simulink model "simulator_prototype_v2"  (R2021b)
(part 10 of 12)

t7179 = ct{2001};
t7181 = ct{2002};
t7185 = ct{2003};
t7187 = ct{2004};
t7188 = ct{2005};
t7193 = ct{2006};
t7195 = ct{2007};
t7198 = ct{2008};
t7200 = ct{2009};
t7201 = ct{2010};
t7204 = ct{2011};
t7209 = ct{2012};
t721 = ct{2013};
t7210 = ct{2014};
t7211 = ct{2015};
t7215 = ct{2016};
t7219 = ct{2017};
t722 = ct{2018};
t7222 = ct{2019};
t7232 = ct{2020};
t7233 = ct{2021};
t7236 = ct{2022};
t7238 = ct{2023};
t7239 = ct{2024};
t724 = ct{2025};
t7240 = ct{2026};
t7245 = ct{2027};
t7248 = ct{2028};
t725 = ct{2029};
t7257 = ct{2030};
t7259 = ct{2031};
t7263 = ct{2032};
t7264 = ct{2033};
t7265 = ct{2034};
t7271 = ct{2035};
t7277 = ct{2036};
t7278 = ct{2037};
t7280 = ct{2038};
t7281 = ct{2039};
t7282 = ct{2040};
t7292 = ct{2041};
t7293 = ct{2042};
t7294 = ct{2043};
t7295 = ct{2044};
t7296 = ct{2045};
t7297 = ct{2046};
t73 = ct{2047};
t7302 = ct{2048};
t7303 = ct{2049};
t7304 = ct{2050};
t7305 = ct{2051};
t7308 = ct{2052};
t7309 = ct{2053};
t7328 = ct{2054};
t7349 = ct{2055};
t7350 = ct{2056};
t7358 = ct{2057};
t7371 = ct{2058};
t7394 = ct{2059};
t7407 = ct{2060};
t7427 = ct{2061};
t7452 = ct{2062};
t7453 = ct{2063};
t7454 = ct{2064};
t7459 = ct{2065};
t7478 = ct{2066};
t7479 = ct{2067};
t749 = ct{2068};
t7530 = ct{2069};
t7534 = ct{2070};
t7553 = ct{2071};
t7566 = ct{2072};
t7567 = ct{2073};
t7606 = ct{2074};
t762 = ct{2075};
t7661 = ct{2076};
t768 = ct{2077};
t7730 = ct{2078};
t7731 = ct{2079};
t7732 = ct{2080};
t7733 = ct{2081};
t7734 = ct{2082};
t777 = ct{2083};
t7790 = ct{2084};
t7791 = ct{2085};
t792 = ct{2086};
t793 = ct{2087};
t801 = ct{2088};
t802 = ct{2089};
t808 = ct{2090};
t813 = ct{2091};
t819 = ct{2092};
t821 = ct{2093};
t850 = ct{2094};
t855 = ct{2095};
t874 = ct{2096};
t878 = ct{2097};
t941 = ct{2098};
t948 = ct{2099};
t951 = ct{2100};
t97 = ct{2101};
t7547 = t4790+t4791+t5152+t5153+t5233+t5234+t5238+t5244+t5277+t5280+t5281+t5287;
t7665 = t50.*t189.*t7661.*9.543032792050485e-17;
t4804 = -t4803;
t4810 = -t4806;
t4939 = t27.*t4933;
t4944 = t27.*t4936;
t5324 = t3586+t3587+t4037+t4042;
t5343 = t3632+t3633+t4086+t4096;
t5368 = t3709+t3713+t4146+t4153;
t5373 = -t5372;
t5439 = -t5436;
t5529 = -t5527;
t5614 = -t5612;
t5656 = -t5654;
t5710 = t4308+t5310;
t5713 = t4310+t5312;
t5738 = t4356+t5327;
t5800 = t56+t73+t5797;
t5801 = t71+t97+t5797;
t5811 = -t5810;
t5823 = -t5822;
t5893 = -t5892;
t5895 = t329+t346+t5849;
t5898 = t354+t387+t5849;
t5920 = -t5919;
t5949 = -t5948;
t5964 = -t5962;
t5976 = t4666+t5647;
t6025 = -t6023;
t6045 = t4316+t5182+t5186;
t6056 = -t6055;
t6072 = -t6070;
t6079 = -t6036.*(t1477-t2502);
t6080 = -t6077;
t6082 = t3057.*t6037;
t6083 = t6036.*(t1477-t2502);
t6122 = -t6121;
t6125 = -t6124;
t6127 = -t6126;
t6149 = -t6146;
t6166 = -t6164;
t6181 = -t6179;
t6192 = t188.*t6170.*8.595599785252598e-1;
t6194 = -t6191;
t6196 = t50.*t189.*t6170.*9.543032792050485e-17;
t6208 = t640+t668+t669+t677+t1604+t1605+t1607+t1628+t2302+t2670+t2680+t2693+t2700+t3276+t3291+t3307+t3589+t3596+t3603+t3616+t4043+t4044;
t6216 = -t6214;
t6229 = t5797.*(t2694-t2701+t3036-t3043).*(t1513+t1879+t2598+t2820+t2834+t3117+t3118).*7.26735e-3;
t6233 = t201.*t6203.*6.246723209935546e-3;
t6249 = -t6246;
t6254 = t50.*t202.*t6203.*6.935255936130809e-19;
t6259 = t3985.*t6036;
t6263 = -t6037.*(t3235-t3535);
t6265 = t3996.*t6036;
t6266 = t3992.*t6037;
t6286 = -t6284;
t6288 = t682+t715+t716+t725+t1741+t1742+t1750+t1754+t2401+t2697+t2712+t2715+t2721+t3324+t3336+t3357+t3635+t3639+t3643+t3657+t4097+t4098;
t6295 = -t6294;
t6300 = t3386.*t6172;
t6342 = t5849.*(t2674-t2676+t3022-t3027).*(t1488+t1874+t2519+t2740+t2747+t3096+t3097);
t6347 = -t6345;
t6358 = -t6309.*(t1477-t2502);
t6361 = t3057.*t6312;
t6362 = t6309.*(t1477-t2502);
t6392 = t3210.*t6332;
t6395 = -t6393;
t6412 = t4899+t4904+t4905+t4910;
t6413 = t4900+t4902+t4906+t4908;
t6415 = t3483.*t6332;
t6438 = t5983.*(t2694-t2701+t3036-t3043).*(t1513+t1879+t2598+t2820+t2834+t3117+t3118).*7.26735e-3;
t6443 = t3901.*t5985.*(t1513+t1879+t2598+t2820+t2834+t3117+t3118).*(-7.26735e-3);
t6444 = t3901.*t5985.*(t1513+t1879+t2598+t2820+t2834+t3117+t3118).*7.26735e-3;
t6454 = t3985.*t6309;
t6457 = -t6312.*(t3235-t3535);
t6459 = t3877.*t6332;
t6460 = t3992.*t6312;
t6461 = t6312.*(t3235-t3535);
t6462 = t3996.*t6309;
t6472 = t4510.*t6172;
t6475 = -t6172.*(t3544-t4013);
t6488 = -t6487;
t6510 = t3667+t3676+t4796+t4799+t4802+t4812;
t6513 = t3673+t3674+t4794+t4801+t4806+t4808;
t6524 = -t6522;
t6561 = t4994+t6195;
t6583 = -t6582;
t6587 = t3745+t3758+t4921+t4924+t4933+t4943;
t6588 = t3748+t3751+t4918+t4927+t4936+t4938;
t6589 = t3748+t3753+t4913+t4927+t4936+t4941;
t6590 = t3746+t3762+t4919+t4922+t4934+t4946;
t6595 = t5013+t6243;
t6609 = -t6607;
t6610 = -t6608;
t6617 = t5067+t5071+t5078+t5087;
t6618 = t5059+t5074+t5081+t5086;
t6619 = t5066+t5068+t5079+t5089;
t6620 = t5062+t5074+t5081+t5083;
t6625 = t27.*t2363.*t6594;
t6636 = t3003.*t6594;
t6650 = t3057.*t6594;
t6651 = -t6594.*(t1477-t2502);
t6704 = -t27.*t6594.*(t1896-t3232);
t6705 = t27.*t3528.*t6594;
t6712 = -t6708;
t6718 = t5181+t5183+t5187+t5188;
t6725 = t5798.*t5849;
t6727 = t5799.*t5849;
t6731 = t5797.*t5884;
t6766 = t3985.*t6594;
t6767 = -t6594.*(t3235-t3535);
t6768 = t3992.*t6594;
t6769 = t6594.*(t3235-t3535);
t6770 = t3996.*t6594;
t6773 = -t6772;
t6774 = -t3210.*(-t5181+t5185+t4541.*(t2813-t2835+t18.*(t1456-t2355).*1.02e-6+t23.*(t1456-t2355).*9.0e-8)+t4125.*(t3544-t4013));
t6775 = t3210.*(-t5181+t5185+t4541.*(t2813-t2835+t18.*(t1456-t2355).*1.02e-6+t23.*(t1456-t2355).*9.0e-8)+t4125.*(t3544-t4013));
t6791 = -t3483.*(-t5181+t5185+t4541.*(t2813-t2835+t18.*(t1456-t2355).*1.02e-6+t23.*(t1456-t2355).*9.0e-8)+t4125.*(t3544-t4013));
t6792 = t3483.*(-t5181+t5185+t4541.*(t2813-t2835+t18.*(t1456-t2355).*1.02e-6+t23.*(t1456-t2355).*9.0e-8)+t4125.*(t3544-t4013));
t6806 = t4313+t4320+t4882+t4883+t4980+t4981;
t6808 = t3875+t4276+t4970+t4972+t5006+t5008;
t6810 = -t6809;
t6817 = -t3877.*(-t5181+t5185+t4541.*(t2813-t2835+t18.*(t1456-t2355).*1.02e-6+t23.*(t1456-t2355).*9.0e-8)+t4125.*(t3544-t4013));
t6818 = t3877.*(-t5181+t5185+t4541.*(t2813-t2835+t18.*(t1456-t2355).*1.02e-6+t23.*(t1456-t2355).*9.0e-8)+t4125.*(t3544-t4013));
t6834 = -t3957.*(-t5181+t5185+t4541.*(t2813-t2835+t18.*(t1456-t2355).*1.02e-6+t23.*(t1456-t2355).*9.0e-8)+t4125.*(t3544-t4013));
t6865 = -t6863;
t6875 = t5884.*t5983;
t6877 = t5888.*t5983;
t6896 = t3819+t3821+t5106+t5119+t5134+t5138;
t6897 = t3816+t3828+t5112+t5114+t5133+t5142;
t6898 = t3814+t3833+t5113+t5117+t5132+t5139;
t6899 = t3821+t3826+t5109+t5119+t5134+t5137;
t6903 = t4814.*t6594;
t6906 = -t6594.*(t4127+t33.*(t1959-t3306+t38.*t1022.*(t855-t878).*2.196325630278387e-1));
t6918 = t3210.*t6855;
t6942 = t3483.*t6855;
t6957 = -t6956;
t6964 = -t3385.*(t3817-t5119-t5134+t5135+t3057.*(t2337+t18.*(t1456-t2355)).*9.3e-7+t4491.*(t3235-t3535).*9.3e-7);
t6967 = -t3386.*(t3811+t3833-t5114+t5117-t5133+t5139);
t6971 = t3386.*(t3811+t3833-t5114+t5117-t5133+t5139);
t6982 = t3877.*t6855;
t7071 = -t4510.*(t3811+t3833-t5114+t5117-t5133+t5139);
t7074 = -t4514.*(t3817-t5119-t5134+t5135+t3057.*(t2337+t18.*(t1456-t2355)).*9.3e-7+t4491.*(t3235-t3535).*9.3e-7);
t7078 = -t4541.*(t3817-t5119-t5134+t5135+t3057.*(t2337+t18.*(t1456-t2355)).*9.3e-7+t4491.*(t3235-t3535).*9.3e-7);
t7082 = (t3544-t4013).*(t3811+t3833-t5114+t5117-t5133+t5139);
t7097 = -t7096;
t7104 = -t7102;
t7119 = -t7118;
t7121 = -t7120;
t7162 = -t5797.*(t4795.*(t1896-t3232).*7.26735e-3+t2363.*(t684+t685-t710+t724+t1686-t1690+t1700+t1701+t2371+t2698+t2707-t2716+t2719+t3319-t3327-t3341-t3620+t3622+t3634-t3638+t4076+t4077).*7.26735e-3);
t7163 = t5797.*(t4795.*(t1896-t3232).*7.26735e-3+t2363.*(t684+t685-t710+t724+t1686-t1690+t1700+t1701+t2371+t2698+t2707-t2716+t2719+t3319-t3327-t3341-t3620+t3622+t3634-t3638+t4076+t4077).*7.26735e-3);
t7168 = -t5849.*(t4758.*(t1861-t3214)+t2297.*(t642+t643-t667+t674+t1587+t1606+t1608+t1609+t2295+t2671+t2683+t2684-t2695+t3272+t3290-t3296+t3576+t3582+t3588-t3593+t4015+t4016));
t7192 = t4297+t5000+t5101+t5102+t5604+t5606;
t7207 = t3473+t3479+t3757+t3759+t4629+t4631+t4635+t4637+t4915+t4925+t4940+t4942;
t7208 = t3475+t3477+t3749+t3768+t4628+t4633+t4634+t4639+t4917+t4920+t4935+t4947;
t7275 = t3683+t3686+t3815+t3834+t4836+t4847+t4853+t4859+t5104+t5108+t5136+t5143;
t7276 = t3682+t3687+t3822+t3827+t4835+t4845+t4852+t4858+t5103+t5116+t5140+t5141;
t7283 = -t7282;
et292 = t3681+t3684-t3834+t4849+t4857-t5104+t5105-t5136+t3360.*(t1477-t2502).*9.3e-7+t3996.*(t3493-t3972).*9.0e-8+t18.*t3946.*(t3235-t3535).*9.0e-8;
et293 = t23.*t3946.*(t3235-t3535).*9.3e-7;
t7288 = -t3385.*(et292+et293);
t7289 = -t3386.*(t3680+t3685-t3827+t4848+t4856-t5103+t5111-t5140+t18.*t4833+t3360.*(t1477-t2502).*9.0e-8+t3996.*(t3493-t3972).*1.02e-6+t23.*t3946.*(t3235-t3535).*9.0e-8);
t7290 = t3386.*(t3680+t3685-t3827+t4848+t4856-t5103+t5111-t5140+t18.*t4833+t3360.*(t1477-t2502).*9.0e-8+t3996.*(t3493-t3972).*1.02e-6+t23.*t3946.*(t3235-t3535).*9.0e-8);
t7298 = t5926+t6081+t6503;
t7314 = -t4510.*(t3680+t3685-t3827+t4848+t4856-t5103+t5111-t5140+t18.*t4833+t3360.*(t1477-t2502).*9.0e-8+t3996.*(t3493-t3972).*1.02e-6+t23.*t3946.*(t3235-t3535).*9.0e-8);
et294 = t3681+t3684-t3834+t4849+t4857-t5104+t5105-t5136+t3360.*(t1477-t2502).*9.3e-7+t3996.*(t3493-t3972).*9.0e-8+t18.*t3946.*(t3235-t3535).*9.0e-8;
et295 = t23.*t3946.*(t3235-t3535).*9.3e-7;
t7315 = -t4514.*(et294+et295);
et296 = t3681+t3684-t3834+t4849+t4857-t5104+t5105-t5136+t3360.*(t1477-t2502).*9.3e-7+t3996.*(t3493-t3972).*9.0e-8+t18.*t3946.*(t3235-t3535).*9.0e-8;
et297 = t23.*t3946.*(t3235-t3535).*9.3e-7;
t7316 = -t4541.*(et296+et297);
t7317 = (t3544-t4013).*(t3680+t3685-t3827+t4848+t4856-t5103+t5111-t5140+t18.*t4833+t3360.*(t1477-t2502).*9.0e-8+t3996.*(t3493-t3972).*1.02e-6+t23.*t3946.*(t3235-t3535).*9.0e-8);
t7325 = t5979+t6258+t6581;
t7326 = t5982+t6264+t6580;
t7353 = t4961+t5201+t6182+t7028;
t7364 = t3057.*t7358;
t7365 = t4982+t5226+t6225+t7062;
t7369 = t3522+t3530+t3533+t3539+t5073+t5075+t5080+t5088+t5386+t5387+t5391+t5395;
t7370 = t3526+t3527+t3532+t3542+t5070+t5077+t5084+t5085+t5385+t5390+t5392+t5393;
t7373 = t6123+t6363+t6793;
t7374 = -t2307.*(-t6123+t6359+t3057.*(-t4437-t4438+t4741+t4767+t3942.*(t2694-t2701+t3036-t3043).*4.0e-8+t3946.*(t2694-t2701+t3036-t3043).*2.4e-7));
t7375 = t2307.*(-t6123+t6359+t3057.*(-t4437-t4438+t4741+t4767+t3942.*(t2694-t2701+t3036-t3043).*4.0e-8+t3946.*(t2694-t2701+t3036-t3043).*2.4e-7));
t7376 = -t7358.*(t3235-t3535);
t7377 = t3992.*t7358;
t7378 = t7358.*(t3235-t3535);
t7413 = t3690+t3729+t3769+t3770+t5156+t5166+t5171+t5172+t5446+t5457+t5461+t5462;
t7414 = t3705+t3715+t3760+t3776+t5157+t5161+t5170+t5173+t5451+t5452+t5458+t5465;
et298 = t3385;
et299 = -t3705+t3706+t3756+t3774+t5158-t5170+t5448+t5449-t5458-t5465+t4491.*(t1005+t26.*(t1941-t3308+t39.*t1022.*(t855-t878).*2.196325630278387e-1)).*9.0e-8+t4113.*(t3493-t3972).*9.0e-8;
et300 = -1.0;
t7428 = et298.*et299.*et300;
et301 = t3385;
et302 = -t3705+t3706+t3756+t3774+t5158-t5170+t5448+t5449-t5458-t5465+t4491.*(t1005+t26.*(t1941-t3308+t39.*t1022.*(t855-t878).*2.196325630278387e-1)).*9.0e-8+t4113.*(t3493-t3972).*9.0e-8;
t7429 = et301.*et302;
t7430 = -t3386.*(-t3690+t3724+t3765+t3767+t5162-t5171+t5445+t5455-t5461-t5462+t4491.*(t1005+t26.*(t1941-t3308+t39.*t1022.*(t855-t878).*2.196325630278387e-1)).*1.02e-6+t4113.*(t3493-t3972).*1.02e-6);
t7434 = t6213+t6455+t6889;
t7455 = -t7453;
t7460 = -t3484.*(t6214+t3996.*(t4737+t4744+t4751+t3942.*(t2694-t2701+t3036-t3043).*5.7e-7)+t3992.*(-t4437-t4438+t4741+t4767+t3942.*(t2694-t2701+t3036-t3043).*4.0e-8+t3946.*(t2694-t2701+t3036-t3043).*2.4e-7));
t7461 = t3484.*(t6214+t3996.*(t4737+t4744+t4751+t3942.*(t2694-t2701+t3036-t3043).*5.7e-7)+t3992.*(-t4437-t4438+t4741+t4767+t3942.*(t2694-t2701+t3036-t3043).*4.0e-8+t3946.*(t2694-t2701+t3036-t3043).*2.4e-7));
t7468 = -t4510.*(-t3690+t3724+t3765+t3767+t5162-t5171+t5445+t5455-t5461-t5462+t4491.*(t1005+t26.*(t1941-t3308+t39.*t1022.*(t855-t878).*2.196325630278387e-1)).*1.02e-6+t4113.*(t3493-t3972).*1.02e-6);
et303 = t4514;
et304 = -t3705+t3706+t3756+t3774+t5158-t5170+t5448+t5449-t5458-t5465+t4491.*(t1005+t26.*(t1941-t3308+t39.*t1022.*(t855-t878).*2.196325630278387e-1)).*9.0e-8+t4113.*(t3493-t3972).*9.0e-8;
et305 = -1.0;
t7469 = et303.*et304.*et305;
t7470 = t4510.*(-t3690+t3724+t3765+t3767+t5162-t5171+t5445+t5455-t5461-t5462+t4491.*(t1005+t26.*(t1941-t3308+t39.*t1022.*(t855-t878).*2.196325630278387e-1)).*1.02e-6+t4113.*(t3493-t3972).*1.02e-6);
et306 = t4514;
et307 = -t3705+t3706+t3756+t3774+t5158-t5170+t5448+t5449-t5458-t5465+t4491.*(t1005+t26.*(t1941-t3308+t39.*t1022.*(t855-t878).*2.196325630278387e-1)).*9.0e-8+t4113.*(t3493-t3972).*9.0e-8;
t7471 = et306.*et307;
et308 = t4541;
et309 = -t3705+t3706+t3756+t3774+t5158-t5170+t5448+t5449-t5458-t5465+t4491.*(t1005+t26.*(t1941-t3308+t39.*t1022.*(t855-t878).*2.196325630278387e-1)).*9.0e-8+t4113.*(t3493-t3972).*9.0e-8;
et310 = -1.0;
t7472 = et308.*et309.*et310;
et311 = t3544-t4013;
et312 = -t3690+t3724+t3765+t3767+t5162-t5171+t5445+t5455-t5461-t5462+t4491.*(t1005+t26.*(t1941-t3308+t39.*t1022.*(t855-t878).*2.196325630278387e-1)).*1.02e-6+t4113.*(t3493-t3972).*1.02e-6;
t7473 = et311.*et312;
t7502 = t5454+t5456+t5460+t5466+t5545+t5546+t5550+t5556;
t7503 = t5450+t5459+t5463+t5464+t5542+t5551+t5553+t5554;
t7504 = -t3385.*(t5453-t5460+t5543+t5544-t5550-t5556+t4865.*(t3951+t18.*(t1861-t3214)).*9.3e-7+t4860.*(t3493-t3972).*9.0e-8);
t7505 = -t3386.*(t5447-t5463+t5541+t5547-t5553-t5554+t4865.*(t3951+t18.*(t1861-t3214)).*9.0e-8+t4860.*(t3493-t3972).*1.02e-6);
t7506 = t3386.*(t5447-t5463+t5541+t5547-t5553-t5554+t4865.*(t3951+t18.*(t1861-t3214)).*9.0e-8+t4860.*(t3493-t3972).*1.02e-6);
t7521 = t5884.*t7371;
t7523 = t5888.*t7371;
t7529 = -t4510.*(t5447-t5463+t5541+t5547-t5553-t5554+t4865.*(t3951+t18.*(t1861-t3214)).*9.0e-8+t4860.*(t3493-t3972).*1.02e-6);
t7531 = -t4514.*(t5453-t5460+t5543+t5544-t5550-t5556+t4865.*(t3951+t18.*(t1861-t3214)).*9.3e-7+t4860.*(t3493-t3972).*9.0e-8);
t7532 = t4510.*(t5447-t5463+t5541+t5547-t5553-t5554+t4865.*(t3951+t18.*(t1861-t3214)).*9.0e-8+t4860.*(t3493-t3972).*1.02e-6);
t7533 = t4514.*(t5453-t5460+t5543+t5544-t5550-t5556+t4865.*(t3951+t18.*(t1861-t3214)).*9.3e-7+t4860.*(t3493-t3972).*9.0e-8);
t7535 = -t4541.*(t5453-t5460+t5543+t5544-t5550-t5556+t4865.*(t3951+t18.*(t1861-t3214)).*9.3e-7+t4860.*(t3493-t3972).*9.0e-8);
t7536 = (t3544-t4013).*(t5447-t5463+t5541+t5547-t5553-t5554+t4865.*(t3951+t18.*(t1861-t3214)).*9.0e-8+t4860.*(t3493-t3972).*1.02e-6);
t7555 = t3795+t3801+t3803+t3804+t5418+t5419+t5421+t5424+t5569+t5570+t5574+t5579;
t7556 = t3797+t3798+t3799+t3806+t5416+t5420+t5422+t5423+t5564+t5573+t5576+t5577;
t7599 = -t7371.*(t4795.*(t1896-t3232).*7.26735e-3+t2363.*(t684+t685-t710+t724+t1686-t1690+t1700+t1701+t2371+t2698+t2707-t2716+t2719+t3319-t3327-t3341-t3620+t3622+t3634-t3638+t4076+t4077).*7.26735e-3);
t7600 = t7371.*(t4795.*(t1896-t3232).*7.26735e-3+t2363.*(t684+t685-t710+t724+t1686-t1690+t1700+t1701+t2371+t2698+t2707-t2716+t2719+t3319-t3327-t3341-t3620+t3622+t3634-t3638+t4076+t4077).*7.26735e-3);
t7637 = t5804+t5911+t5978+t6148+t6343+t6531;
t7757 = t6049+t6135+t6212+t6410+t6634+t6814;
t7758 = t6050+t6137+t6215+t6411+t6635+t6815;
t7810 = -t3209.*(-t6068+t6327-t6927+t7096+t7236+t27.*t6594.*(t1896-t3232));
t7811 = t3209.*(-t6068+t6327-t6927+t7096+t7236+t27.*t6594.*(t1896-t3232));
t7813 = (t1861-t3214).*(-t6068+t6327-t6927+t7096+t7236+t27.*t6594.*(t1896-t3232));
t7815 = (t2674-t2676+t3022-t3027).*(-t6068+t6327-t6927+t7096+t7236+t27.*t6594.*(t1896-t3232));
et313 = -t7281+t7452+t6001.*(t1005+t26.*(t1941-t3308+t39.*t1022.*(t855-t878).*2.196325630278387e-1))+t6594.*(t4127+t33.*(t1959-t3306+t38.*t1022.*(t855-t878).*2.196325630278387e-1))+t7193.*(t1896-t3232);
et314 = t4817.*(t3424-t3437+t4552+t4556+t3942.*(t1896-t3232).*5.7e-7+t3946.*(t1896-t3232).*4.0e-8);
t7922 = -t3209.*(et313+et314);
et315 = -t7281+t7452+t6001.*(t1005+t26.*(t1941-t3308+t39.*t1022.*(t855-t878).*2.196325630278387e-1))+t6594.*(t4127+t33.*(t1959-t3306+t38.*t1022.*(t855-t878).*2.196325630278387e-1))+t7193.*(t1896-t3232);
et316 = t4817.*(t3424-t3437+t4552+t4556+t3942.*(t1896-t3232).*5.7e-7+t3946.*(t1896-t3232).*4.0e-8);
t7923 = t3209.*(et315+et316);
et317 = -t7281+t7452+t6001.*(t1005+t26.*(t1941-t3308+t39.*t1022.*(t855-t878).*2.196325630278387e-1))+t6594.*(t4127+t33.*(t1959-t3306+t38.*t1022.*(t855-t878).*2.196325630278387e-1))+t7193.*(t1896-t3232);
et318 = t4817.*(t3424-t3437+t4552+t4556+t3942.*(t1896-t3232).*5.7e-7+t3946.*(t1896-t3232).*4.0e-8);
t7925 = (et317+et318).*(t1861-t3214);
et319 = -t7281+t7452+t6001.*(t1005+t26.*(t1941-t3308+t39.*t1022.*(t855-t878).*2.196325630278387e-1))+t6594.*(t4127+t33.*(t1959-t3306+t38.*t1022.*(t855-t878).*2.196325630278387e-1))+t7193.*(t1896-t3232);
et320 = t4817.*(t3424-t3437+t4552+t4556+t3942.*(t1896-t3232).*5.7e-7+t3946.*(t1896-t3232).*4.0e-8);
t7927 = (et319+et320).*(t2674-t2676+t3022-t3027);
t7952 = t6126+t6354+t6789+t7280+t7328+t7553;
t7961 = t6346+t6573+t6993+t7293+t7349+t7566;
t5355 = t50.*t189.*t5324.*9.543032792050485e-17;
t5363 = t2297.*t5324;
t5376 = t50.*t202.*t5343.*6.935255936130809e-19;
t5401 = t2363.*t5343.*7.26735e-3;
t5905 = t3901.*t5324.*(t1513+t1879+t2598+t2820+t2834+t3117+t3118).*(-7.26735e-3);
t5906 = t3901.*t5324.*(t1513+t1879+t2598+t2820+t2834+t3117+t3118).*7.26735e-3;
t5934 = -t3877.*t5368.*(t1488+t1874+t2519+t2740+t2747+t3096+t3097);
t6084 = -t6082;
t6089 = t5710.*(t2694-t2701+t3036-t3043).*(t1513+t1879+t2598+t2820+t2834+t3117+t3118).*7.26735e-3;
t6093 = t3901.*t5713.*(t1513+t1879+t2598+t2820+t2834+t3117+t3118).*(-7.26735e-3);
t6106 = -t3877.*t5738.*(t1488+t1874+t2519+t2740+t2747+t3096+t3097);
t6108 = t3901.*t3918.*t5800.*7.26735e-3;
t6110 = t3901.*t3918.*t5801.*7.26735e-3;
t6117 = t3901.*t3984.*t5800.*7.26735e-3;
t6118 = t3901.*t3984.*t5801.*7.26735e-3;
t6131 = t3901.*t4149.*t5800.*7.26735e-3;
t6133 = t3901.*t4149.*t5801.*7.26735e-3;
t6193 = -t6192;
t6197 = -t6196;
t6226 = t3877.*t3892.*t5895;
t6228 = t3877.*t3892.*t5898;
t6231 = -t6229;
t6240 = t3877.*t3941.*t5895;
t6242 = t3877.*t3941.*t5898;
t6255 = -t6254;
t6256 = t5800.*(t2694-t2701+t3036-t3043).*(t1513+t1879+t2598+t2820+t2834+t3117+t3118).*7.26735e-3;
t6261 = -t6259;
t6283 = t3877.*t4108.*t5895;
t6287 = t3877.*t4108.*t5898;
t6290 = t2297.*t6208;
t6291 = t2307.*t6208;
t6292 = t2338.*t6208;
t6301 = -t6300;
t6316 = t2363.*t6288.*7.26735e-3;
t6318 = t2388.*t6288.*7.26735e-3;
t6319 = t2419.*t6288.*7.26735e-3;
t6334 = t3877.*t4298.*t5895;
t6336 = t3877.*t4298.*t5898;
t6352 = t5895.*(t2674-t2676+t3022-t3027).*(t1488+t1874+t2519+t2740+t2747+t3096+t3097);
t6364 = -t6361;
t6376 = t5314.*t5800;
t6379 = t5314.*t5801;
t6385 = t5321.*t5800;
t6386 = t5321.*t5801;
t6420 = t5368.*t5800;
t6421 = t5368.*t5801;
t6425 = t5220.*t5895;
t6429 = t5220.*t5898;
t6432 = t3901.*t5976.*(t1513+t1879+t2598+t2820+t2834+t3117+t3118).*(-7.26735e-3);
t6448 = t5262.*t5895;
t6449 = t5262.*t5898;
t6469 = t5324.*t5895;
t6470 = t5324.*t5898;
t6476 = t3385.*t6412;
t6478 = t3386.*t6413;
et321 = -t2306-t2317+t3144+t3147+t35.*t941.*t948.*(t850-t874).*3.775747223193135e-1;
et322 = t36.*t941.*t948.*(t850-t874).*2.244797987218524e-1;
t6499 = t5895.*(et321+et322).*(t1488+t1874+t2519+t2740+t2747+t3096+t3097);
et323 = -t2306-t2317+t3144+t3147+t35.*t941.*t948.*(t850-t874).*3.775747223193135e-1;
et324 = t36.*t941.*t948.*(t850-t874).*2.244797987218524e-1;
t6501 = t5898.*(et323+et324).*(t1488+t1874+t2519+t2740+t2747+t3096+t3097);
t6509 = t3670+t3672+t4793+t4800+t4807+t4810;
t6512 = t3669+t3676+t4796+t4798+t4804+t4812;
t6535 = t34.*t3057.*t6510;
t6537 = t28.*t3057.*t6513;
t6540 = t3142.*t6510;
t6541 = t3141.*t6513;
t6546 = t3250.*t6513;
t6547 = -t6510.*(t2527-t3009);
t6549 = t3385.*t6510;
t6551 = t3386.*t6510;
t6553 = t3385.*t6513;
t6556 = t3386.*t6513;
t6562 = t5738.*t5800;
t6563 = t5738.*t5801;
t6596 = t4510.*t6413;
t6597 = t4514.*t6412;
t6598 = t4541.*t6412;
t6599 = -t6413.*(t3544-t4013);
t6621 = t5710.*t5884;
t6623 = t5710.*t5888;
t6626 = t5713.*t5895;
t6628 = t5713.*t5898;
t6637 = -t34.*t6510.*(t3235-t3535);
t6638 = t34.*t3992.*t6510;
t6639 = t34.*t6510.*(t3235-t3535);
t6640 = -t28.*t6513.*(t3235-t3535);
t6641 = t28.*t3992.*t6513;
t6642 = t28.*t6513.*(t3235-t3535);
t6643 = t34.*t3057.*t6587;
t6644 = t28.*t3057.*t6588;
t6656 = t3141.*t6588;
t6657 = t3142.*t6587;
t6665 = t3250.*t6588;
t6666 = -t6587.*(t2527-t3009);
t6668 = t6587.*(t2527-t3009);
t6669 = t4245.*t6510;
t6670 = t4246.*t6513;
t6671 = t4247.*t6510;
t6674 = t4248.*t6513;
t6675 = t28.*t3057.*t6620;
t6676 = t34.*t3057.*t6617;
t6677 = t3385.*t6587;
t6678 = t3385.*t6588;
t6679 = t3385.*t6589;
t6680 = t3386.*t6587;
t6681 = t3386.*t6588;
t6684 = t3386.*t6590;
t6695 = t3141.*t6620;
t6697 = t3142.*t6617;
t6701 = t3250.*t6620;
t6702 = -t6617.*(t2527-t3009);
t6709 = t3385.*t6617;
t6710 = t3385.*t6618;
t6711 = t3385.*t6620;
t6713 = t3386.*t6617;
t6715 = t3386.*t6619;
t6716 = t3386.*t6620;
t6726 = t5800.*t5843;
t6729 = t5801.*t5843;
t6730 = -t6727;
t6732 = t5796.*t5895;
t6734 = t5799.*t5895;
t6735 = t5801.*t5884;
t6737 = t4510.*t6510;
t6740 = t4514.*t6510;
t6741 = t4510.*t6513;
t6742 = t4514.*t6513;
t6745 = t4541.*t6510;
t6746 = -t6510.*(t3544-t4013);
t6747 = t4541.*t6513;
t6749 = -t6513.*(t3544-t4013);
t6757 = -t34.*t6587.*(t3235-t3535);
t6758 = -t28.*t6588.*(t3235-t3535);
t6759 = t34.*t3992.*t6587;
t6760 = t28.*t3992.*t6588;
t6771 = -t6770;
t6778 = t4245.*t6587;
t6780 = t4246.*t6588;
t6781 = t4247.*t6587;
t6782 = t4248.*t6588;
t6784 = -t28.*t6620.*(t3235-t3535);
t6785 = -t34.*t6617.*(t3235-t3535);
t6786 = t28.*t3992.*t6620;
t6787 = t34.*t3992.*t6617;
t6798 = t4245.*t6617;
t6800 = t4246.*t6620;
t6801 = t4247.*t6617;
t6802 = t4248.*t6620;
t6819 = t4510.*t6587;
t6820 = t4510.*t6588;
t6821 = t4510.*t6590;
t6822 = t4514.*t6587;
t6824 = t4514.*t6588;
t6825 = t4514.*t6589;
t6826 = t4541.*t6587;
t6827 = t4541.*t6588;
t6828 = t4541.*t6589;
t6829 = -t6587.*(t3544-t4013);
t6830 = -t6588.*(t3544-t4013);
t6831 = -t6590.*(t3544-t4013);
t6832 = t6587.*(t3544-t4013);
t6836 = t4510.*t6617;
t6837 = t4510.*t6619;
t6838 = t4510.*t6620;
t6839 = t3918.*t6561.*(t2694-t2701+t3036-t3043).*(-7.26735e-3);
t6840 = t4514.*t6617;
t6841 = t4514.*t6618;
t6843 = t4514.*t6620;
t6844 = t4541.*t6617;
t6845 = t4541.*t6618;
t6846 = t4541.*t6620;
t6847 = -t6617.*(t3544-t4013);
t6848 = -t6619.*(t3544-t4013);
t6849 = -t6620.*(t3544-t4013);
t6850 = t6617.*(t3544-t4013);
t6856 = t3984.*t6561.*(t2694-t2701+t3036-t3043).*(-7.26735e-3);
t6857 = t3210.*t6806;
t6867 = t4149.*t6561.*(t2694-t2701+t3036-t3043).*(-7.26735e-3);
t6868 = t4149.*t6561.*(t2694-t2701+t3036-t3043).*7.26735e-3;
t6869 = t3210.*t6808;
t6871 = t5895.*t5976;
t6872 = t5898.*t5976;
t6876 = -t6875;
t6878 = -t6877;
t6879 = t5895.*t5985;
t6881 = t5898.*t5985;
t6886 = -t3892.*t6595.*(t2674-t2676+t3022-t3027);
t6891 = t3483.*t6806;
t6901 = t3483.*t6808;
t6904 = -t4108.*t6595.*(t2674-t2676+t3022-t3027);
t6905 = t4108.*t6595.*(t2674-t2676+t3022-t3027);
t6919 = -t6918;
t6929 = t34.*t3057.*t6898;
t6930 = t28.*t3057.*t6899;
t6934 = t3877.*t6806;
t6935 = -t4298.*t6595.*(t2674-t2676+t3022-t3027);
t6936 = t3141.*t6899;
t6938 = t3142.*t6898;
t6945 = t3957.*t6806;
t6946 = t5293.*t6510;
t6947 = t5295.*t6510;
t6948 = t6513.*(t4840-t34.*(t1005+t26.*(t1941-t3308+t39.*t1022.*(t855-t878).*2.196325630278387e-1)));
t6949 = t3877.*t6808;
t6952 = -t6513.*(t4133-t4843);
t6959 = t3250.*t6899;
t6960 = -t6898.*(t2527-t3009);
t6961 = t3957.*t6808;
t6965 = t3385.*t6898;
t6966 = t3385.*t6899;
t6968 = t3386.*t6898;
t6970 = t3386.*t6899;
t6983 = -t6982;
et325 = t3563.*1.33637554986e-4+t3693-t3694+t33.*(t1896-t3232).*4.36041e-5;
et326 = t33.*t34.*(t1896-t3232).*7.26350557185e-5;
t6991 = -t6561.*(et325+et326);
t6996 = -t34.*t6898.*(t3235-t3535);
t6997 = -t28.*t6899.*(t3235-t3535);
t6998 = t34.*t3992.*t6898;
t6999 = t28.*t3992.*t6899;
t7002 = -t6595.*(t3505.*1.838876e-2-t3570+t3571+t22.*(t1861-t3214).*(3.0./5.0e+2)+t22.*t23.*(t1861-t3214).*9.99471e-3);
t7003 = -t6561.*(t3349-t3649+t28.*(t3235-t3535).*1.33637554986e-4+t34.*(t3235-t3535).*7.26350557185e-5);
t7010 = t5258.*t6595;
t7011 = t6588.*(t4840-t34.*(t1005+t26.*(t1941-t3308+t39.*t1022.*(t855-t878).*2.196325630278387e-1)));
t7013 = t5293.*t6587;
t7014 = t5295.*t6587;
t7016 = -t6588.*(t4133-t4843);
t7019 = t4245.*t6898;
t7020 = t4246.*t6899;
t7021 = t4247.*t6898;
t7024 = t4248.*t6899;
t7030 = -t6561.*(t3547.*1.33637554986e-4+t4119-t4120+t34.*(t1896-t3232).*7.26350557185e-5);
t7035 = t6620.*(t4840-t34.*(t1005+t26.*(t1941-t3308+t39.*t1022.*(t855-t878).*2.196325630278387e-1)));
t7036 = t5293.*t6617;
t7037 = t5295.*t6617;
t7038 = -t6620.*(t4133-t4843);
t7040 = -t6595.*(-t4007+t4011+t18.*(t1861-t3214).*1.838876e-2+t23.*(t1861-t3214).*9.99471e-3);
t7072 = t4510.*t6898;
t7073 = t4510.*t6899;
t7075 = t4514.*t6898;
t7077 = t4514.*t6899;
t7079 = -t4822.*t6595.*(t1488+t1874+t2519+t2740+t2747+t3096+t3097);
t7080 = t4541.*t6898;
t7081 = t4541.*t6899;
t7083 = -t6898.*(t3544-t4013);
t7084 = -t6899.*(t3544-t4013);
t7085 = t6898.*(t3544-t4013);
t7105 = t5737.*t6561;
tau_c = ft_15({t1005,t1022,t1089,t1104,t1105,t1108,t1115,t1121,t1158,t1159,t1196,t1205,t1210,t1212,t1217,t1218,t123,t1237,t1238,t1288,t1289,t1302,t1303,t1319,t1320,t1336,t1348,t1350,t1351,t1360,t1369,t1378,t1396,t14,t140,t1425,t1435,t1456,t1477,t1488,t15,t1513,t1539,t1554,t1577,t1578,t1586,t1587,t16,t1600,t1606,t1608,t1609,t1629,t1637,t1640,t1641,t1659,t1661,t1666,t1667,t1683,t1686,t1690,t1692,t17,t1700,t1701,t1705,t1712,t1758,t1759,t1775,t1776,t18,t1861,t1874,t1879,t188,t1881,t189,t1896,t19,t1901,t1941,t1959,t1973,t1993,t1994,t2,t20,t201,t202,t2023,t2053,t2060,t2089,t2090,t2098,t2099,t21,t2117,t2120,t2122,t2123,t2139,t2140,t2147,t2152,t2154,t2155,t2159,t2165,t2174,t2183,t2187,t2193,t2194,t2195,t2199,t22,t2203,t2215,t2219,t2222,t2223,t2239,t2240,t2256,t2257,t2292,t2295,t2297,t23,t2303,t2306,t2307,t2308,t2317,t2337,t2338,t2339,t2355,t236,t2361,t2362,t2363,t2367,t2368,t237,t2371,t2378,t238,t2388,t24,t241,t2414,t2419,t244,t25,t2502,t2510,t2519,t2527,t2530,t2555,t2556,t2572,t2583,t2598,t26,t2605,t2606,t2612,t2613,t2618,t2619,t262,t264,t2651,t2652,t2671,t2674,t2676,t2683,t2684,t2689,t2694,t2695,t2698,t27,t2701,t2707,t2716,t2719,t2740,t2747,t2754,t28,t2801,t2804,t2813,t2814,t2820,t2831,t2834,t2835,t2838,t2850,t2851,t2953,t2963,t2964,t2975,t2979,t2990,t2991,t2994,t3,t30,t3009,t3022,t3027,t3030,t3036,t3043,t3047,t3054,t3056,t3057,t3064,t3072,t3080,t3096,t3097,t31,t3109,t3117,t3118,t3121,t3122,t3128,t313,t3130,t3131,t3132,t314,t3144,t3147,t3156,t3157,t3170,t3189,t3190,t32,t3200,t3206,t3209,t321,t3210,t3214,t3228,t3229,t3230,t3231,t3232,t3235,t3269,t3270,t3272,t3283,t3290,t3292,t3296,t33,t3305,t3306,t3308,t3313,t3318,t3319,t332,t3327,t3330,t3334,t3341,t3349,t335,t3359,t3360,t3376,t3385,t3386,t3395,t3399,t34,t3405,t3409,t3410,t3412,t3417,t3420,t3421,t3423,t3424,t3435,t3437,t3455,t3465,t3468,t3470,t3480,t3481,t3483,t3484,t3493,t3498,t35,t350,t3505,t3524,t3528,t3535,t3544,t3547,t3560,t3563,t3570,t3571,t3576,t3582,t3588,t3590,t3593,t36,t3617,t3618,t3619,t3620,t3621,t3622,t3628,t3634,t3637,t3638,t3649,t366,t3664,t3665,t3680,t3681,t3684,t3685,t3689,t3693,t3694,t3708,t3714,t3716,t3723,t3732,t3734,t3735,t3744,t3755,t3763,t3764,t3766,t3771,t3772,t3775,t3778,t3779,t3782,t3783,t3784,t3790,t3791,t3794,t38,t3811,t3817,t3827,t3833,t3834,t3847,t3849,t3850,t3861,t3862,t3863,t3865,t3866,t3869,t3870,t3871,t3872,t3877,t3880,t3882,t3891,t3892,t3893,t3898,t39,t3901,t3904,t3910,t3918,t3922,t3928,t3934,t3940,t3941,t3942,t3946,t3951,t3957,t3959,t3967,t3972,t3974,t3984,t3985,t3992,t3996,t4,t4007,t4011,t4013,t4015,t4016,t4027,t4062,t4071,t4072,t4076,t4077,t4080,t410,t4106,t4108,t4109,t4119,t4120,t4127,t4133,t4134,t4149,t4152,t4154,t4155,t4160,t4163,t4173,t4175,t4196,t42,t4200,t4201,t4219,t4220,t4221,t4227,t4228,t4230,t4231,t4238,t4239,t4242,t4243,t4244,t4255,t4256,t4257,t4259,t4264,t4266,t4277,t4279,t4280,t4281,t4285,t4287,t4291,t4292,t4295,t4298,t43,t4304,t4311,t4321,t4322,t4323,t4324,t4362,t4363,t4400,t4405,t4406,t4409,t4413,t4421,t4428,t4429,t4432,t4436,t4437,t4438,t4444,t4447,t4458,t4491,t4496,t4499,t4500,t4504,t4507,t4510,t4513,t4514,t4519,t4520,t4531,t4540,t4541,t4543,t4552,t4554,t4555,t4556,t4560,t4571,t4572,t4576,t4579,t4582,t4588,t4589,t4595,t4599,t46,t4602,t4610,t4612,t4613,t4614,t4615,t4617,t4620,t4640,t4641,t4642,t4644,t4645,t4647,t4650,t4652,t4655,t4658,t4661,t4663,t4664,t4667,t4669,t4679,t4680,t4682,t4683,t4686,t4688,t4699,t47,t4702,t4703,t4704,t4705,t4737,t4741,t4742,t4744,t4751,t4752,t4758,t4767,t4772,t4777,t4780,t4785,t4786,t4788,t4789,t4792,t4795,t4805,t4809,t4814,t4816,t4817,t4819,t4822,t4823,t4824,t4826,t4829,t4833,t4840,t4842,t4843,t4848,t4849,t4850,t4851,t4856,t4857,t4860,t4865,t4868,t4869,t4870,t4871,t4872,t4874,t4875,t4898,t4911,t4926,t4929,t4930,t4931,t4932,t4939,t4944,t4945,t4948,t4950,t4952,t4953,t4954,t4956,t4958,t4959,t4960,t4962,t4963,t4965,t4974,t4975,t4976,t4977,t4983,t4984,t4985,t4986,t4987,t4992,t4995,t4998,t5,t50,t5005,t5007,t5014,t5031,t5033,t5034,t5035,t5036,t5038,t5039,t5040,t5041,t5042,t5047,t5048,t5049,t5051,t5052,t5055,t5056,t5057,t5058,t5063,t5069,t5076,t5092,t5103,t5104,t5105,t5111,t5114,t5117,t5119,t5133,t5134,t5135,t5136,t5139,t5140,t5144,t5147,t5148,t5149,t5150,t5151,t5152,t5155,t5164,t5184,t5186,t5189,t5191,t5192,t5195,t5196,t5198,t5202,t5203,t5204,t5207,t5209,t5210,t5220,t5223,t5224,t5225,t5227,t5230,t5231,t5235,t5240,t5241,t5243,t5245,t5246,t5247,t5248,t5250,t5252,t5254,t5257,t5262,t5273,t5276,t5277,t5278,t5281,t5282,t5285,t5286,t5288,t5289,t5291,t5293,t5295,t5301,t5304,t5306,t5307,t5308,t5314,t5316,t5317,t5320,t5321,t5322,t5324,t5328,t5329,t5330,t5331,t5332,t5335,t5337,t5338,t5339,t5340,t5342,t5344,t5345,t5346,t5347,t5348,t5349,t5350,t5355,t5356,t5357,t5358,t5359,t5361,t5362,t5363,t5365,t5367,t5368,t5372,t5373,t5376,t5377,t5379,t5380,t5381,t5383,t5384,t5388,t5389,t5396,t5397,t5399,t5400,t5401,t5402,t5403,t5405,t5407,t5411,t5412,t5413,t5414,t5426,t5427,t5428,t5429,t5432,t5433,t5434,t5435,t5436,t5437,t5438,t5439,t5440,t5441,t5443,t5444,t5453,t5460,t5468,t5480,t5481,t5482,t5483,t5484,t5486,t5487,t5488,t5489,t5490,t5491,t5492,t5493,t5494,t5495,t5496,t5498,t5499,t5500,t5501,t5502,t5503,t5504,t5505,t5506,t5507,t5509,t5512,t5513,t5514,t5515,t5516,t5517,t5518,t5520,t5521,t5522,t5523,t5524,t5525,t5526,t5527,t5528,t5529,t5530,t5531,t5532,t5533,t5534,t5535,t5536,t5537,t5538,t5539,t5543,t5544,t5550,t5552,t5556,t5557,t5558,t5559,t5561,t5563,t5566,t5568,t5575,t5578,t5580,t5581,t5582,t5583,t5585,t5586,t5588,t5589,t5592,t5593,t5594,t5595,t5596,t5597,t56,t5601,t5602,t5612,t5613,t5614,t5615,t5617,t5619,t5620,t5621,t5622,t5623,t5624,t5625,t5626,t5627,t5628,t5629,t5631,t5632,t5635,t5636,t5639,t5650,t5651,t5652,t5653,t5654,t5655,t5656,t5657,t5658,t5659,t5660,t5662,t5663,t5664,t5665,t5666,t5670,t5671,t5674,t5675,t5678,t5679,t5681,t5682,t5685,t5687,t5689,t5693,t5694,t5695,t5696,t5698,t5700,t5701,t5702,t5703,t5704,t5705,t5706,t5707,t5708,t5709,t5710,t5711,t5712,t5713,t5714,t5715,t5716,t5717,t5718,t5720,t5721,t5722,t5723,t5725,t5726,t5727,t5728,t5730,t5731,t5733,t5735,t5738,t5739,t5740,t5741,t5742,t5743,t5745,t5746,t5748,t5749,t5750,t5751,t5756,t5757,t5760,t5761,t5762,t5763,t5764,t5765,t5770,t5771,t5772,t5773,t5775,t5776,t5777,t5778,t5779,t5781,t5782,t5783,t5785,t5786,t5787,t5788,t5791,t5792,t5793,t5794,t5796,t5797,t5798,t5799,t5800,t5801,t5805,t5808,t5809,t5810,t5811,t5813,t5815,t5816,t5818,t5819,t5820,t5821,t5822,t5823,t5824,t5825,t5829,t5831,t5832,t5833,t5835,t5836,t5837,t5838,t5842,t5843,t5844,t5845,t5846,t5847,t5848,t5849,t5850,t5851,t5852,t5853,t5854,t5855,t5857,t5858,t5859,t5860,t5861,t5862,t5863,t5864,t5865,t5866,t5868,t5870,t5871,t5873,t5874,t5875,t5876,t5877,t5879,t5881,t5882,t5883,t5884,t5885,t5886,t5887,t5888,t5889,t5890,t5891,t5892,t5893,t5894,t5895,t5896,t5898,t5899,t5900,t5902,t5904,t5906,t5907,t5908,t5910,t5912,t5913,t5914,t5916,t5917,t5918,t5919,t5920,t5922,t5923,t5924,t5925,t5927,t5929,t5930,t5932,t5933,t5934,t5936,t5938,t5939,t5940,t5943,t5944,t5945,t5946,t5947,t5948,t5949,t5951,t5952,t5953,t5954,t5956,t5957,t5958,t5959,t5960,t5963,t5964,t5966,t5968,t5969,t5970,t5972,t5973,t5975,t5976,t5977,t5981,t5983,t5985,t5987,t5989,t5990,t5991,t5994,t5996,t5997,t5998,t6,t60,t6001,t6002,t6004,t6005,t6007,t6008,t6009,t6010,t6017,t6018,t6019,t6020,t6021,t6022,t6023,t6024,t6025,t6028,t6030,t6031,t6034,t6035,t6037,t6039,t6043,t6044,t6046,t6047,t6048,t6051,t6053,t6054,t6055,t6058,t6062,t6064,t6066,t6067,t6068,t6069,t6070,t6071,t6072,t6073,t6075,t6076,t6077,t6079,t6080,t6082,t6083,t6084,t6088,t6089,t6091,t6092,t6093,t6095,t6096,t6098,t6099,t6101,t6102,t6103,t6104,t6105,t6106,t6107,t6108,t6110,t6112,t6113,t6114,t6116,t6117,t6118,t6119,t6120,t6121,t6122,t6123,t6124,t6125,t6129,t6130,t6131,t6133,t6139,t6141,t6142,t6143,t6144,t6147,t6149,t6150,t6154,t6155,t6156,t6157,t6160,t6161,t6162,t6166,t6168,t6169,t6172,t6178,t6179,t6180,t6181,t6183,t6184,t6185,t6190,t6191,t6193,t6194,t6197,t6198,t6199,t6200,t6202,t6206,t6207,t6209,t6210,t6211,t6214,t6216,t6218,t6219,t6221,t6222,t6223,t6224,t6226,t6228,t6229,t6231,t6232,t6233,t6234,t6235,t6237,t6238,t6239,t6240,t6241,t6242,t6244,t6245,t6247,t6248,t6249,t6250,t6251,t6252,t6253,t6255,t6256,t6257,t6259,t6260,t6261,t6262,t6263,t6265,t6266,t6267,t6270,t6272,t6273,t6274,t6275,t6277,t6282,t6283,t6286,t6287,t6289,t6290,t6291,t6292,t6293,t6294,t6295,t6296,t6297,t6298,t6299,t6300,t6301,t6302,t6303,t6304,t6305,t6316,t6317,t6318,t6319,t6321,t6322,t6323,t6328,t6330,t6331,t6333,t6334,t6336,t6338,t6339,t6341,t6342,t6344,t6345,t6347,t6348,t6349,t6351,t6352,t6356,t6357,t6358,t6359,t6360,t6361,t6362,t6364,t6365,t6366,t6367,t6368,t6369,t6370,t6371,t6372,t6373,t6374,t6375,t6376,t6378,t6379,t6382,t6384,t6385,t6386,t6387,t6388,t6389,t6390,t6391,t6392,t6394,t6395,t6396,t6397,t6398,t6399,t6400,t6401,t6403,t6404,t6406,t6407,t6413,t6414,t6415,t6417,t6419,t642,t6420,t6421,t6422,t6423,t6424,t6425,t6427,t6429,t643,t6431,t6432,t6433,t6434,t6435,t6436,t6437,t6438,t6439,t6441,t6442,t6444,t6445,t6446,t6447,t6448,t6449,t6450,t6451,t6452,t6453,t6454,t6456,t6459,t6460,t6461,t6462,t6463,t6464,t6466,t6468,t6469,t6470,t6471,t6472,t6473,t6474,t6475,t6476,t6478,t6480,t6481,t6482,t6483,t6484,t6485,t6486,t6488,t6489,t649,t6490,t6491,t6492,t6493,t6494,t6495,t6496,t6497,t6499,t6501,t6504,t6505,t6507,t6508,t6509,t6510,t6511,t6512,t6515,t6518,t6519,t6521,t6522,t6523,t6524,t6525,t6526,t6527,t6528,t6529,t6532,t6533,t6534,t6535,t6537,t6540,t6541,t6543,t6544,t6545,t6546,t6547,t6549,t6551,t6553,t6556,t6559,t6560,t6561,t6562,t6563,t6565,t6566,t6568,t6570,t6571,t6572,t6574,t6577,t6578,t6583,t6584,t6585,t6586,t6587,t6588,t6591,t6592,t6593,t6595,t6596,t6597,t6598,t6599,t6600,t6601,t6603,t6604,t6605,t6608,t6609,t6610,t6611,t6612,t6613,t6614,t6617,t6620,t6621,t6623,t6625,t6626,t6628,t6636,t6638,t6639,t6641,t6642,t6643,t6644,t6645,t6649,t6650,t6651,t6656,t6657,t6658,t6660,t6663,t6664,t6665,t6668,t6669,t667,t6670,t6671,t6674,t6675,t6676,t6677,t6678,t6679,t6680,t6681,t6684,t6688,t6689,t6690,t6691,t6692,t6695,t6697,t670,t6701,t6702,t6703,t6704,t6705,t6707,t6709,t6710,t6711,t6712,t6713,t6715,t6716,t6720,t6722,t6725,t6726,t6727,t6729,t6730,t6731,t6732,t6734,t6735,t6737,t674,t6740,t6741,t6742,t6745,t6746,t6747,t6749,t6752,t6753,t6754,t6755,t6756,t6757,t6758,t6759,t6760,t6763,t6764,t6765,t6766,t6767,t6768,t6769,t6770,t6771,t6772,t6773,t6774,t6775,t6776,t6777,t6778,t6780,t6781,t6782,t6784,t6785,t6786,t6787,t6788,t6792,t6794,t6795,t6796,t6797,t6798,t6800,t6801,t6802,t6807,t6809,t6810,t6811,t6812,t6813,t6816,t6818,t6819,t6820,t6821,t6822,t6824,t6825,t6826,t6827,t6828,t6830,t6831,t6832,t6833,t6834,t6836,t6837,t6838,t6839,t684,t6840,t6841,t6843,t6844,t6845,t6846,t6848,t6849,t685,t6850,t6854,t6856,t6857,t686,t6860,t6861,t6863,t6864,t6865,t6866,t6868,t6869,t687,t6871,t6872,t6873,t6876,t6878,t6879,t6881,t6884,t6885,t6886,t6887,t6888,t6890,t6891,t6892,t6893,t6898,t6899,t6900,t6901,t6903,t6905,t6906,t6910,t6913,t6916,t6917,t6919,t6920,t6924,t6925,t6926,t6927,t6928,t6929,t6930,t6932,t6933,t6934,t6935,t6936,t6937,t6938,t6942,t6943,t6944,t6945,t6946,t6947,t6948,t6949,t6952,t6954,t6955,t6956,t6957,t6958,t6959,t6960,t6961,t6964,t6965,t6966,t6968,t6970,t6971,t6972,t6973,t6975,t6979,t6983,t6984,t6986,t6988,t6989,t6991,t6992,t6993,t6996,t6997,t6998,t6999,t7,t7003,t7010,t7011,t7012,t7013,t7014,t7015,t7016,t7018,t7019,t7020,t7021,t7024,t7029,t7030,t7035,t7036,t7037,t7038,t7039,t7040,t7041,t7050,t7051,t7053,t7054,t7055,t7056,t7057,t7058,t7060,t7061,t7068,t707,t7071,t7072,t7073,t7074,t7075,t7077,t7078,t7079,t708,t7080,t7081,t7082,t7084,t7085,t7087,t7089,t7091,t7093,t7094,t7097,t7098,t7099,t710,t7101,t7103,t7104,t7105,t7107,t7108,t7114,t7119,t7121,t7127,t7128,t7141,t7148,t7152,t7157,t7163,t7168,t7174,t7177,t7179,t7181,t7185,t7187,t7188,t7192,t7195,t7198,t7200,t7201,t7204,t7207,t7208,t7209,t721,t7210,t7211,t7215,t7219,t722,t7222,t7232,t7233,t7238,t7239,t724,t7240,t7245,t7248,t7257,t7259,t7263,t7264,t7265,t7271,t7277,t7278,t7281,t7282,t7283,t7288,t7290,t7292,t7293,t7294,t7295,t7296,t7297,t7298,t7302,t7303,t7304,t7305,t7308,t7309,t7314,t7315,t7316,t7317,t7325,t7326,t7349,t7350,t7353,t7364,t7365,t7369,t7370,t7371,t7375,t7376,t7377,t7378,t7394,t7407,t7427,t7429,t7430,t7453,t7454,t7455,t7459,t7461,t7470,t7471,t7472,t7473,t7478,t7479,t749,t7504,t7505,t7506,t7521,t7523,t7530,t7532,t7533,t7534,t7535,t7536,t7555,t7556,t7566,t7567,t7600,t7606,t762,t7637,t7665,t768,t7730,t7731,t7732,t7733,t7734,t7757,t7758,t777,t7790,t7791,t7811,t7813,t7815,t792,t7922,t7923,t7925,t7927,t793,t7952,t801,t802,t808,t813,t819,t821,t850,t855,t874,t878,t941,t948,t951});
end
function tau_c = ft_15(ct)
t1005 = ct{1};
t1022 = ct{2};
t1089 = ct{3};
t1104 = ct{4};
t1105 = ct{5};
t1108 = ct{6};
t1115 = ct{7};
t1121 = ct{8};
t1158 = ct{9};
t1159 = ct{10};
t1196 = ct{11};
t1205 = ct{12};
t1210 = ct{13};
t1212 = ct{14};
t1217 = ct{15};
t1218 = ct{16};
t123 = ct{17};
t1237 = ct{18};
t1238 = ct{19};
t1288 = ct{20};
t1289 = ct{21};
t1302 = ct{22};
t1303 = ct{23};
t1319 = ct{24};
t1320 = ct{25};
t1336 = ct{26};
t1348 = ct{27};
t1350 = ct{28};
t1351 = ct{29};
t1360 = ct{30};
t1369 = ct{31};
t1378 = ct{32};
t1396 = ct{33};
t14 = ct{34};
t140 = ct{35};
t1425 = ct{36};
t1435 = ct{37};
t1456 = ct{38};
t1477 = ct{39};
t1488 = ct{40};
t15 = ct{41};
t1513 = ct{42};
t1539 = ct{43};
t1554 = ct{44};
t1577 = ct{45};
t1578 = ct{46};
t1586 = ct{47};
t1587 = ct{48};
t16 = ct{49};
t1600 = ct{50};
t1606 = ct{51};
t1608 = ct{52};
t1609 = ct{53};
t1629 = ct{54};
t1637 = ct{55};
t1640 = ct{56};
t1641 = ct{57};
t1659 = ct{58};
t1661 = ct{59};
t1666 = ct{60};
t1667 = ct{61};
t1683 = ct{62};
t1686 = ct{63};
t1690 = ct{64};
t1692 = ct{65};
t17 = ct{66};
t1700 = ct{67};
t1701 = ct{68};
t1705 = ct{69};
t1712 = ct{70};
t1758 = ct{71};
t1759 = ct{72};
t1775 = ct{73};
t1776 = ct{74};
t18 = ct{75};
t1861 = ct{76};
t1874 = ct{77};
t1879 = ct{78};
t188 = ct{79};
t1881 = ct{80};
t189 = ct{81};
t1896 = ct{82};
t19 = ct{83};
t1901 = ct{84};
t1941 = ct{85};
t1959 = ct{86};
t1973 = ct{87};
t1993 = ct{88};
t1994 = ct{89};
t2 = ct{90};
t20 = ct{91};
t201 = ct{92};
t202 = ct{93};
t2023 = ct{94};
t2053 = ct{95};
t2060 = ct{96};
t2089 = ct{97};
t2090 = ct{98};
t2098 = ct{99};
t2099 = ct{100};
t21 = ct{101};
t2117 = ct{102};
t2120 = ct{103};
t2122 = ct{104};
t2123 = ct{105};
t2139 = ct{106};
t2140 = ct{107};
t2147 = ct{108};
t2152 = ct{109};
t2154 = ct{110};
t2155 = ct{111};
t2159 = ct{112};
t2165 = ct{113};
t2174 = ct{114};
t2183 = ct{115};
t2187 = ct{116};
t2193 = ct{117};
t2194 = ct{118};
t2195 = ct{119};
t2199 = ct{120};
t22 = ct{121};
t2203 = ct{122};
t2215 = ct{123};
t2219 = ct{124};
t2222 = ct{125};
t2223 = ct{126};
t2239 = ct{127};
t2240 = ct{128};
t2256 = ct{129};
t2257 = ct{130};
t2292 = ct{131};
t2295 = ct{132};
t2297 = ct{133};
t23 = ct{134};
t2303 = ct{135};
t2306 = ct{136};
t2307 = ct{137};
t2308 = ct{138};
t2317 = ct{139};
t2337 = ct{140};
t2338 = ct{141};
t2339 = ct{142};
t2355 = ct{143};
t236 = ct{144};
t2361 = ct{145};
t2362 = ct{146};
t2363 = ct{147};
t2367 = ct{148};
t2368 = ct{149};
t237 = ct{150};
t2371 = ct{151};
t2378 = ct{152};
t238 = ct{153};
t2388 = ct{154};
t24 = ct{155};
t241 = ct{156};
t2414 = ct{157};
t2419 = ct{158};
t244 = ct{159};
t25 = ct{160};
t2502 = ct{161};
t2510 = ct{162};
t2519 = ct{163};
t2527 = ct{164};
t2530 = ct{165};
t2555 = ct{166};
t2556 = ct{167};
t2572 = ct{168};
t2583 = ct{169};
t2598 = ct{170};
t26 = ct{171};
t2605 = ct{172};
t2606 = ct{173};
t2612 = ct{174};
t2613 = ct{175};
t2618 = ct{176};
t2619 = ct{177};
t262 = ct{178};
t264 = ct{179};
t2651 = ct{180};
t2652 = ct{181};
t2671 = ct{182};
t2674 = ct{183};
t2676 = ct{184};
t2683 = ct{185};
t2684 = ct{186};
t2689 = ct{187};
t2694 = ct{188};
t2695 = ct{189};
t2698 = ct{190};
t27 = ct{191};
t2701 = ct{192};
t2707 = ct{193};
t2716 = ct{194};
t2719 = ct{195};
t2740 = ct{196};
t2747 = ct{197};
t2754 = ct{198};
t28 = ct{199};
t2801 = ct{200};
t2804 = ct{201};
t2813 = ct{202};
t2814 = ct{203};
t2820 = ct{204};
t2831 = ct{205};
t2834 = ct{206};
t2835 = ct{207};
t2838 = ct{208};
t2850 = ct{209};
t2851 = ct{210};
t2953 = ct{211};
t2963 = ct{212};
t2964 = ct{213};
t2975 = ct{214};
t2979 = ct{215};
t2990 = ct{216};
t2991 = ct{217};
t2994 = ct{218};
t3 = ct{219};
t30 = ct{220};
t3009 = ct{221};
t3022 = ct{222};
t3027 = ct{223};
t3030 = ct{224};
t3036 = ct{225};
t3043 = ct{226};
t3047 = ct{227};
t3054 = ct{228};
t3056 = ct{229};
t3057 = ct{230};
t3064 = ct{231};
t3072 = ct{232};
t3080 = ct{233};
t3096 = ct{234};
t3097 = ct{235};
t31 = ct{236};
t3109 = ct{237};
t3117 = ct{238};
t3118 = ct{239};
t3121 = ct{240};
t3122 = ct{241};
t3128 = ct{242};
t313 = ct{243};
t3130 = ct{244};
t3131 = ct{245};
t3132 = ct{246};
t314 = ct{247};
t3144 = ct{248};
t3147 = ct{249};
t3156 = ct{250};
t3157 = ct{251};
t3170 = ct{252};
t3189 = ct{253};
t3190 = ct{254};
t32 = ct{255};
t3200 = ct{256};
t3206 = ct{257};
t3209 = ct{258};
t321 = ct{259};
t3210 = ct{260};
t3214 = ct{261};
t3228 = ct{262};
t3229 = ct{263};
t3230 = ct{264};
t3231 = ct{265};
t3232 = ct{266};
t3235 = ct{267};
t3269 = ct{268};
t3270 = ct{269};
t3272 = ct{270};
t3283 = ct{271};
t3290 = ct{272};
t3292 = ct{273};
t3296 = ct{274};
t33 = ct{275};
t3305 = ct{276};
t3306 = ct{277};
t3308 = ct{278};
t3313 = ct{279};
t3318 = ct{280};
t3319 = ct{281};
t332 = ct{282};
t3327 = ct{283};
t3330 = ct{284};
t3334 = ct{285};
t3341 = ct{286};
t3349 = ct{287};
t335 = ct{288};
t3359 = ct{289};
t3360 = ct{290};
t3376 = ct{291};
t3385 = ct{292};
t3386 = ct{293};
t3395 = ct{294};
t3399 = ct{295};
t34 = ct{296};
t3405 = ct{297};
t3409 = ct{298};
t3410 = ct{299};
t3412 = ct{300};
t3417 = ct{301};
t3420 = ct{302};
t3421 = ct{303};
t3423 = ct{304};
t3424 = ct{305};
t3435 = ct{306};
t3437 = ct{307};
t3455 = ct{308};
t3465 = ct{309};
t3468 = ct{310};
t3470 = ct{311};
t3480 = ct{312};
t3481 = ct{313};
t3483 = ct{314};
t3484 = ct{315};
t3493 = ct{316};
t3498 = ct{317};
t35 = ct{318};
t350 = ct{319};
t3505 = ct{320};
t3524 = ct{321};
t3528 = ct{322};
t3535 = ct{323};
t3544 = ct{324};
t3547 = ct{325};
t3560 = ct{326};
t3563 = ct{327};
t3570 = ct{328};
t3571 = ct{329};
t3576 = ct{330};
t3582 = ct{331};
t3588 = ct{332};
t3590 = ct{333};
t3593 = ct{334};
t36 = ct{335};
t3617 = ct{336};
t3618 = ct{337};
t3619 = ct{338};
t3620 = ct{339};
t3621 = ct{340};
t3622 = ct{341};
t3628 = ct{342};
t3634 = ct{343};
t3637 = ct{344};
t3638 = ct{345};
t3649 = ct{346};
t366 = ct{347};
t3664 = ct{348};
t3665 = ct{349};
t3680 = ct{350};
t3681 = ct{351};
t3684 = ct{352};
t3685 = ct{353};
t3689 = ct{354};
t3693 = ct{355};
t3694 = ct{356};
t3708 = ct{357};
t3714 = ct{358};
t3716 = ct{359};
t3723 = ct{360};
t3732 = ct{361};
t3734 = ct{362};
t3735 = ct{363};
t3744 = ct{364};
t3755 = ct{365};
t3763 = ct{366};
t3764 = ct{367};
t3766 = ct{368};
t3771 = ct{369};
t3772 = ct{370};
t3775 = ct{371};
t3778 = ct{372};
t3779 = ct{373};
t3782 = ct{374};
t3783 = ct{375};
t3784 = ct{376};
t3790 = ct{377};
t3791 = ct{378};
t3794 = ct{379};
t38 = ct{380};
t3811 = ct{381};
t3817 = ct{382};
t3827 = ct{383};
t3833 = ct{384};
t3834 = ct{385};
t3847 = ct{386};
t3849 = ct{387};
t3850 = ct{388};
t3861 = ct{389};
t3862 = ct{390};
t3863 = ct{391};
t3865 = ct{392};
t3866 = ct{393};
t3869 = ct{394};
t3870 = ct{395};
t3871 = ct{396};
t3872 = ct{397};
t3877 = ct{398};
t3880 = ct{399};
t3882 = ct{400};
t3891 = ct{401};
t3892 = ct{402};
t3893 = ct{403};
t3898 = ct{404};
t39 = ct{405};
t3901 = ct{406};
t3904 = ct{407};
t3910 = ct{408};
t3918 = ct{409};
t3922 = ct{410};
t3928 = ct{411};
t3934 = ct{412};
t3940 = ct{413};
t3941 = ct{414};
t3942 = ct{415};
t3946 = ct{416};
t3951 = ct{417};
t3957 = ct{418};
t3959 = ct{419};
t3967 = ct{420};
t3972 = ct{421};
t3974 = ct{422};
t3984 = ct{423};
t3985 = ct{424};
t3992 = ct{425};
t3996 = ct{426};
t4 = ct{427};
t4007 = ct{428};
t4011 = ct{429};
t4013 = ct{430};
t4015 = ct{431};
t4016 = ct{432};
t4027 = ct{433};
t4062 = ct{434};
t4071 = ct{435};
t4072 = ct{436};
t4076 = ct{437};
t4077 = ct{438};
t4080 = ct{439};
t410 = ct{440};
t4106 = ct{441};
t4108 = ct{442};
t4109 = ct{443};
t4119 = ct{444};
t4120 = ct{445};
t4127 = ct{446};
t4133 = ct{447};
t4134 = ct{448};
t4149 = ct{449};
t4152 = ct{450};
t4154 = ct{451};
t4155 = ct{452};
t4160 = ct{453};
t4163 = ct{454};
t4173 = ct{455};
t4175 = ct{456};
t4196 = ct{457};
t42 = ct{458};
t4200 = ct{459};
t4201 = ct{460};
t4219 = ct{461};
t4220 = ct{462};
t4221 = ct{463};
t4227 = ct{464};
t4228 = ct{465};
t4230 = ct{466};
t4231 = ct{467};
t4238 = ct{468};
t4239 = ct{469};
t4242 = ct{470};
t4243 = ct{471};
t4244 = ct{472};
t4255 = ct{473};
t4256 = ct{474};
t4257 = ct{475};
t4259 = ct{476};
t4264 = ct{477};
t4266 = ct{478};
t4277 = ct{479};
t4279 = ct{480};
t4280 = ct{481};
t4281 = ct{482};
t4285 = ct{483};
t4287 = ct{484};
t4291 = ct{485};
t4292 = ct{486};
t4295 = ct{487};
t4298 = ct{488};
t43 = ct{489};
t4304 = ct{490};
t4311 = ct{491};
t4321 = ct{492};
t4322 = ct{493};
t4323 = ct{494};
t4324 = ct{495};
t4362 = ct{496};
t4363 = ct{497};
t4400 = ct{498};
t4405 = ct{499};
t4406 = ct{500};
t4409 = ct{501};
t4413 = ct{502};
t4421 = ct{503};
t4428 = ct{504};
t4429 = ct{505};
t4432 = ct{506};
t4436 = ct{507};
t4437 = ct{508};
t4438 = ct{509};
t4444 = ct{510};
t4447 = ct{511};
t4458 = ct{512};
t4491 = ct{513};
t4496 = ct{514};
t4499 = ct{515};
t4500 = ct{516};
t4504 = ct{517};
t4507 = ct{518};
t4510 = ct{519};
t4513 = ct{520};
t4514 = ct{521};
t4519 = ct{522};
t4520 = ct{523};
t4531 = ct{524};
t4540 = ct{525};
t4541 = ct{526};
t4543 = ct{527};
t4552 = ct{528};
t4554 = ct{529};
t4555 = ct{530};
t4556 = ct{531};
t4560 = ct{532};
t4571 = ct{533};
t4572 = ct{534};
t4576 = ct{535};
t4579 = ct{536};
t4582 = ct{537};
t4588 = ct{538};
t4589 = ct{539};
t4595 = ct{540};
t4599 = ct{541};
t46 = ct{542};
t4602 = ct{543};
t4610 = ct{544};
t4612 = ct{545};
t4613 = ct{546};
t4614 = ct{547};
t4615 = ct{548};
t4617 = ct{549};
t4620 = ct{550};
t4640 = ct{551};
t4641 = ct{552};
t4642 = ct{553};
t4644 = ct{554};
t4645 = ct{555};
t4647 = ct{556};
t4650 = ct{557};
t4652 = ct{558};
t4655 = ct{559};
t4658 = ct{560};
t4661 = ct{561};
t4663 = ct{562};
t4664 = ct{563};
t4667 = ct{564};
t4669 = ct{565};
t4679 = ct{566};
t4680 = ct{567};
t4682 = ct{568};
t4683 = ct{569};
t4686 = ct{570};
t4688 = ct{571};
t4699 = ct{572};
t47 = ct{573};
t4702 = ct{574};
t4703 = ct{575};
t4704 = ct{576};
t4705 = ct{577};
t4737 = ct{578};
t4741 = ct{579};
t4742 = ct{580};
t4744 = ct{581};
t4751 = ct{582};
t4752 = ct{583};
t4758 = ct{584};
t4767 = ct{585};
t4772 = ct{586};
t4777 = ct{587};
t4780 = ct{588};
t4785 = ct{589};
t4786 = ct{590};
t4788 = ct{591};
t4789 = ct{592};
t4792 = ct{593};
t4795 = ct{594};
t4805 = ct{595};
t4809 = ct{596};
t4814 = ct{597};
t4816 = ct{598};
t4817 = ct{599};
t4819 = ct{600};
t4822 = ct{601};
t4823 = ct{602};
t4824 = ct{603};
t4826 = ct{604};
t4829 = ct{605};
t4833 = ct{606};
t4840 = ct{607};
t4842 = ct{608};
t4843 = ct{609};
t4848 = ct{610};
t4849 = ct{611};
t4850 = ct{612};
t4851 = ct{613};
t4856 = ct{614};
t4857 = ct{615};
t4860 = ct{616};
t4865 = ct{617};
t4868 = ct{618};
t4869 = ct{619};
t4870 = ct{620};
t4871 = ct{621};
t4872 = ct{622};
t4874 = ct{623};
t4875 = ct{624};
t4898 = ct{625};
t4911 = ct{626};
t4926 = ct{627};
t4929 = ct{628};
t4930 = ct{629};
t4931 = ct{630};
t4932 = ct{631};
t4939 = ct{632};
t4944 = ct{633};
t4945 = ct{634};
t4948 = ct{635};
t4950 = ct{636};
t4952 = ct{637};
t4953 = ct{638};
t4954 = ct{639};
t4956 = ct{640};
t4958 = ct{641};
t4959 = ct{642};
t4960 = ct{643};
t4962 = ct{644};
t4963 = ct{645};
t4965 = ct{646};
t4974 = ct{647};
t4975 = ct{648};
t4976 = ct{649};
t4977 = ct{650};
t4983 = ct{651};
t4984 = ct{652};
t4985 = ct{653};
t4986 = ct{654};
t4987 = ct{655};
t4992 = ct{656};
t4995 = ct{657};
t4998 = ct{658};
t5 = ct{659};
t50 = ct{660};
t5005 = ct{661};
t5007 = ct{662};
t5014 = ct{663};
t5031 = ct{664};
t5033 = ct{665};
t5034 = ct{666};
t5035 = ct{667};
t5036 = ct{668};
t5038 = ct{669};
t5039 = ct{670};
t5040 = ct{671};
t5041 = ct{672};
t5042 = ct{673};
t5047 = ct{674};
t5048 = ct{675};
t5049 = ct{676};
t5051 = ct{677};
t5052 = ct{678};
t5055 = ct{679};
t5056 = ct{680};
t5057 = ct{681};
t5058 = ct{682};
t5063 = ct{683};
t5069 = ct{684};
t5076 = ct{685};
t5092 = ct{686};
t5103 = ct{687};
t5104 = ct{688};
t5105 = ct{689};
t5111 = ct{690};
t5114 = ct{691};
t5117 = ct{692};
t5119 = ct{693};
t5133 = ct{694};
t5134 = ct{695};
t5135 = ct{696};
t5136 = ct{697};
t5139 = ct{698};
t5140 = ct{699};
t5144 = ct{700};
t5147 = ct{701};
t5148 = ct{702};
t5149 = ct{703};
t5150 = ct{704};
t5151 = ct{705};
t5152 = ct{706};
t5155 = ct{707};
t5164 = ct{708};
t5184 = ct{709};
t5186 = ct{710};
t5189 = ct{711};
t5191 = ct{712};
t5192 = ct{713};
t5195 = ct{714};
t5196 = ct{715};
t5198 = ct{716};
t5202 = ct{717};
t5203 = ct{718};
t5204 = ct{719};
t5207 = ct{720};
t5209 = ct{721};
t5210 = ct{722};
t5220 = ct{723};
t5223 = ct{724};
t5224 = ct{725};
t5225 = ct{726};
t5227 = ct{727};
t5230 = ct{728};
t5231 = ct{729};
t5235 = ct{730};
t5240 = ct{731};
t5241 = ct{732};
t5243 = ct{733};
t5245 = ct{734};
t5246 = ct{735};
t5247 = ct{736};
t5248 = ct{737};
t5250 = ct{738};
t5252 = ct{739};
t5254 = ct{740};
t5257 = ct{741};
t5262 = ct{742};
t5273 = ct{743};
t5276 = ct{744};
t5277 = ct{745};
t5278 = ct{746};
t5281 = ct{747};
t5282 = ct{748};
t5285 = ct{749};
t5286 = ct{750};
t5288 = ct{751};
t5289 = ct{752};
t5291 = ct{753};
t5293 = ct{754};
t5295 = ct{755};
t5301 = ct{756};
t5304 = ct{757};
t5306 = ct{758};
t5307 = ct{759};
t5308 = ct{760};
t5314 = ct{761};
t5316 = ct{762};
t5317 = ct{763};
t5320 = ct{764};
t5321 = ct{765};
t5322 = ct{766};
t5324 = ct{767};
t5328 = ct{768};
t5329 = ct{769};
t5330 = ct{770};
t5331 = ct{771};
t5332 = ct{772};
t5335 = ct{773};
t5337 = ct{774};
t5338 = ct{775};
t5339 = ct{776};
t5340 = ct{777};
t5342 = ct{778};
t5344 = ct{779};
t5345 = ct{780};
t5346 = ct{781};
t5347 = ct{782};
t5348 = ct{783};
t5349 = ct{784};
t5350 = ct{785};
t5355 = ct{786};
t5356 = ct{787};
t5357 = ct{788};
t5358 = ct{789};
t5359 = ct{790};
t5361 = ct{791};
t5362 = ct{792};
t5363 = ct{793};
t5365 = ct{794};
t5367 = ct{795};
t5368 = ct{796};
t5372 = ct{797};
t5373 = ct{798};
t5376 = ct{799};
t5377 = ct{800};
t5379 = ct{801};
t5380 = ct{802};
t5381 = ct{803};
t5383 = ct{804};
t5384 = ct{805};
t5388 = ct{806};
t5389 = ct{807};
t5396 = ct{808};
t5397 = ct{809};
t5399 = ct{810};
t5400 = ct{811};
t5401 = ct{812};
t5402 = ct{813};
t5403 = ct{814};
t5405 = ct{815};
t5407 = ct{816};
t5411 = ct{817};
t5412 = ct{818};
t5413 = ct{819};
t5414 = ct{820};
t5426 = ct{821};
t5427 = ct{822};
t5428 = ct{823};
t5429 = ct{824};
t5432 = ct{825};
t5433 = ct{826};
t5434 = ct{827};
t5435 = ct{828};
t5436 = ct{829};
t5437 = ct{830};
t5438 = ct{831};
t5439 = ct{832};
t5440 = ct{833};
t5441 = ct{834};
t5443 = ct{835};
t5444 = ct{836};
t5453 = ct{837};
t5460 = ct{838};
t5468 = ct{839};
t5480 = ct{840};
t5481 = ct{841};
t5482 = ct{842};
t5483 = ct{843};
t5484 = ct{844};
t5486 = ct{845};
t5487 = ct{846};
t5488 = ct{847};
t5489 = ct{848};
t5490 = ct{849};
t5491 = ct{850};
t5492 = ct{851};
t5493 = ct{852};
t5494 = ct{853};
t5495 = ct{854};
t5496 = ct{855};
t5498 = ct{856};
t5499 = ct{857};
t5500 = ct{858};
t5501 = ct{859};
t5502 = ct{860};
t5503 = ct{861};
t5504 = ct{862};
t5505 = ct{863};
t5506 = ct{864};
t5507 = ct{865};
t5509 = ct{866};
t5512 = ct{867};
t5513 = ct{868};
t5514 = ct{869};
t5515 = ct{870};
t5516 = ct{871};
t5517 = ct{872};
t5518 = ct{873};
t5520 = ct{874};
t5521 = ct{875};
t5522 = ct{876};
t5523 = ct{877};
t5524 = ct{878};
t5525 = ct{879};
t5526 = ct{880};
t5527 = ct{881};
t5528 = ct{882};
t5529 = ct{883};
t5530 = ct{884};
t5531 = ct{885};
t5532 = ct{886};
t5533 = ct{887};
t5534 = ct{888};
t5535 = ct{889};
t5536 = ct{890};
t5537 = ct{891};
t5538 = ct{892};
t5539 = ct{893};
t5543 = ct{894};
t5544 = ct{895};
t5550 = ct{896};
t5552 = ct{897};
t5556 = ct{898};
t5557 = ct{899};
t5558 = ct{900};
t5559 = ct{901};
t5561 = ct{902};
t5563 = ct{903};
t5566 = ct{904};
t5568 = ct{905};
t5575 = ct{906};
t5578 = ct{907};
t5580 = ct{908};
t5581 = ct{909};
t5582 = ct{910};
t5583 = ct{911};
t5585 = ct{912};
t5586 = ct{913};
t5588 = ct{914};
t5589 = ct{915};
t5592 = ct{916};
t5593 = ct{917};
t5594 = ct{918};
t5595 = ct{919};
t5596 = ct{920};
t5597 = ct{921};
t56 = ct{922};
t5601 = ct{923};
t5602 = ct{924};
t5612 = ct{925};
t5613 = ct{926};
t5614 = ct{927};
t5615 = ct{928};
t5617 = ct{929};
t5619 = ct{930};
t5620 = ct{931};
t5621 = ct{932};
t5622 = ct{933};
t5623 = ct{934};
t5624 = ct{935};
t5625 = ct{936};
t5626 = ct{937};
t5627 = ct{938};
t5628 = ct{939};
t5629 = ct{940};
t5631 = ct{941};
t5632 = ct{942};
t5635 = ct{943};
t5636 = ct{944};
t5639 = ct{945};
t5650 = ct{946};
t5651 = ct{947};
t5652 = ct{948};
t5653 = ct{949};
t5654 = ct{950};
t5655 = ct{951};
t5656 = ct{952};
t5657 = ct{953};
t5658 = ct{954};
t5659 = ct{955};
t5660 = ct{956};
t5662 = ct{957};
t5663 = ct{958};
t5664 = ct{959};
t5665 = ct{960};
t5666 = ct{961};
t5670 = ct{962};
t5671 = ct{963};
t5674 = ct{964};
t5675 = ct{965};
t5678 = ct{966};
t5679 = ct{967};
t5681 = ct{968};
t5682 = ct{969};
t5685 = ct{970};
t5687 = ct{971};
t5689 = ct{972};
t5693 = ct{973};
t5694 = ct{974};
t5695 = ct{975};
t5696 = ct{976};
t5698 = ct{977};
t5700 = ct{978};
t5701 = ct{979};
t5702 = ct{980};
t5703 = ct{981};
t5704 = ct{982};
t5705 = ct{983};
t5706 = ct{984};
t5707 = ct{985};
t5708 = ct{986};
t5709 = ct{987};
t5710 = ct{988};
t5711 = ct{989};
t5712 = ct{990};
t5713 = ct{991};
t5714 = ct{992};
t5715 = ct{993};
t5716 = ct{994};
t5717 = ct{995};
t5718 = ct{996};
t5720 = ct{997};
t5721 = ct{998};
t5722 = ct{999};
t5723 = ct{1000};
t5725 = ct{1001};
t5726 = ct{1002};
t5727 = ct{1003};
t5728 = ct{1004};
t5730 = ct{1005};
t5731 = ct{1006};
t5733 = ct{1007};
t5735 = ct{1008};
t5738 = ct{1009};
t5739 = ct{1010};
t5740 = ct{1011};
t5741 = ct{1012};
t5742 = ct{1013};
t5743 = ct{1014};
t5745 = ct{1015};
t5746 = ct{1016};
t5748 = ct{1017};
t5749 = ct{1018};
t5750 = ct{1019};
t5751 = ct{1020};
t5756 = ct{1021};
t5757 = ct{1022};
t5760 = ct{1023};
t5761 = ct{1024};
t5762 = ct{1025};
t5763 = ct{1026};
t5764 = ct{1027};
t5765 = ct{1028};
t5770 = ct{1029};
t5771 = ct{1030};
t5772 = ct{1031};
t5773 = ct{1032};
t5775 = ct{1033};
t5776 = ct{1034};
t5777 = ct{1035};
t5778 = ct{1036};
t5779 = ct{1037};
t5781 = ct{1038};
t5782 = ct{1039};
t5783 = ct{1040};
t5785 = ct{1041};
t5786 = ct{1042};
t5787 = ct{1043};
t5788 = ct{1044};
t5791 = ct{1045};
t5792 = ct{1046};
t5793 = ct{1047};
t5794 = ct{1048};
t5796 = ct{1049};
t5797 = ct{1050};
t5798 = ct{1051};
t5799 = ct{1052};
t5800 = ct{1053};
t5801 = ct{1054};
t5805 = ct{1055};
t5808 = ct{1056};
t5809 = ct{1057};
t5810 = ct{1058};
t5811 = ct{1059};
t5813 = ct{1060};
t5815 = ct{1061};
t5816 = ct{1062};
t5818 = ct{1063};
t5819 = ct{1064};
t5820 = ct{1065};
t5821 = ct{1066};
t5822 = ct{1067};
t5823 = ct{1068};
t5824 = ct{1069};
t5825 = ct{1070};
t5829 = ct{1071};
t5831 = ct{1072};
t5832 = ct{1073};
t5833 = ct{1074};
t5835 = ct{1075};
t5836 = ct{1076};
t5837 = ct{1077};
t5838 = ct{1078};
t5842 = ct{1079};
t5843 = ct{1080};
t5844 = ct{1081};
t5845 = ct{1082};
t5846 = ct{1083};
t5847 = ct{1084};
t5848 = ct{1085};
t5849 = ct{1086};
t5850 = ct{1087};
t5851 = ct{1088};
t5852 = ct{1089};
t5853 = ct{1090};
t5854 = ct{1091};
t5855 = ct{1092};
t5857 = ct{1093};
t5858 = ct{1094};
t5859 = ct{1095};
t5860 = ct{1096};
t5861 = ct{1097};
t5862 = ct{1098};
t5863 = ct{1099};
t5864 = ct{1100};
t5865 = ct{1101};
t5866 = ct{1102};
t5868 = ct{1103};
t5870 = ct{1104};
t5871 = ct{1105};
t5873 = ct{1106};
t5874 = ct{1107};
t5875 = ct{1108};
t5876 = ct{1109};
t5877 = ct{1110};
t5879 = ct{1111};
t5881 = ct{1112};
t5882 = ct{1113};
t5883 = ct{1114};
t5884 = ct{1115};
t5885 = ct{1116};
t5886 = ct{1117};
t5887 = ct{1118};
t5888 = ct{1119};
t5889 = ct{1120};
t5890 = ct{1121};
t5891 = ct{1122};
t5892 = ct{1123};
t5893 = ct{1124};
t5894 = ct{1125};
t5895 = ct{1126};
t5896 = ct{1127};
t5898 = ct{1128};
t5899 = ct{1129};
t5900 = ct{1130};
t5902 = ct{1131};
t5904 = ct{1132};
t5906 = ct{1133};
t5907 = ct{1134};
t5908 = ct{1135};
t5910 = ct{1136};
t5912 = ct{1137};
t5913 = ct{1138};
t5914 = ct{1139};
t5916 = ct{1140};
t5917 = ct{1141};
t5918 = ct{1142};
t5919 = ct{1143};
t5920 = ct{1144};
t5922 = ct{1145};
t5923 = ct{1146};
t5924 = ct{1147};
t5925 = ct{1148};
t5927 = ct{1149};
t5929 = ct{1150};
t5930 = ct{1151};
t5932 = ct{1152};
t5933 = ct{1153};
t5934 = ct{1154};
t5936 = ct{1155};
t5938 = ct{1156};
t5939 = ct{1157};
t5940 = ct{1158};
t5943 = ct{1159};
t5944 = ct{1160};
t5945 = ct{1161};
t5946 = ct{1162};
t5947 = ct{1163};
t5948 = ct{1164};
t5949 = ct{1165};
t5951 = ct{1166};
t5952 = ct{1167};
t5953 = ct{1168};
t5954 = ct{1169};
t5956 = ct{1170};
t5957 = ct{1171};
t5958 = ct{1172};
t5959 = ct{1173};
t5960 = ct{1174};
t5963 = ct{1175};
t5964 = ct{1176};
t5966 = ct{1177};
t5968 = ct{1178};
t5969 = ct{1179};
t5970 = ct{1180};
t5972 = ct{1181};
t5973 = ct{1182};
t5975 = ct{1183};
t5976 = ct{1184};
t5977 = ct{1185};
t5981 = ct{1186};
t5983 = ct{1187};
t5985 = ct{1188};
t5987 = ct{1189};
t5989 = ct{1190};
t5990 = ct{1191};
t5991 = ct{1192};
t5994 = ct{1193};
t5996 = ct{1194};
t5997 = ct{1195};
t5998 = ct{1196};
t6 = ct{1197};
t60 = ct{1198};
t6001 = ct{1199};
t6002 = ct{1200};
t6004 = ct{1201};
t6005 = ct{1202};
t6007 = ct{1203};
t6008 = ct{1204};
t6009 = ct{1205};
t6010 = ct{1206};
t6017 = ct{1207};
t6018 = ct{1208};
t6019 = ct{1209};
t6020 = ct{1210};
t6021 = ct{1211};
t6022 = ct{1212};
t6023 = ct{1213};
t6024 = ct{1214};
t6025 = ct{1215};
t6028 = ct{1216};
t6030 = ct{1217};
t6031 = ct{1218};
t6034 = ct{1219};
t6035 = ct{1220};
t6037 = ct{1221};
t6039 = ct{1222};
t6043 = ct{1223};
t6044 = ct{1224};
t6046 = ct{1225};
t6047 = ct{1226};
t6048 = ct{1227};
t6051 = ct{1228};
t6053 = ct{1229};
t6054 = ct{1230};
t6055 = ct{1231};
t6058 = ct{1232};
t6062 = ct{1233};
t6064 = ct{1234};
t6066 = ct{1235};
t6067 = ct{1236};
t6068 = ct{1237};
t6069 = ct{1238};
t6070 = ct{1239};
t6071 = ct{1240};
t6072 = ct{1241};
t6073 = ct{1242};
t6075 = ct{1243};
t6076 = ct{1244};
t6077 = ct{1245};
t6079 = ct{1246};
t6080 = ct{1247};
t6082 = ct{1248};
t6083 = ct{1249};
t6084 = ct{1250};
t6088 = ct{1251};
t6089 = ct{1252};
t6091 = ct{1253};
t6092 = ct{1254};
t6093 = ct{1255};
t6095 = ct{1256};
t6096 = ct{1257};
t6098 = ct{1258};
t6099 = ct{1259};
t6101 = ct{1260};
t6102 = ct{1261};
t6103 = ct{1262};
t6104 = ct{1263};
t6105 = ct{1264};
t6106 = ct{1265};
t6107 = ct{1266};
t6108 = ct{1267};
t6110 = ct{1268};
t6112 = ct{1269};
t6113 = ct{1270};
t6114 = ct{1271};
t6116 = ct{1272};
t6117 = ct{1273};
t6118 = ct{1274};
t6119 = ct{1275};
t6120 = ct{1276};
t6121 = ct{1277};
t6122 = ct{1278};
t6123 = ct{1279};
t6124 = ct{1280};
t6125 = ct{1281};
t6129 = ct{1282};
t6130 = ct{1283};
t6131 = ct{1284};
t6133 = ct{1285};
t6139 = ct{1286};
t6141 = ct{1287};
t6142 = ct{1288};
t6143 = ct{1289};
t6144 = ct{1290};
t6147 = ct{1291};
t6149 = ct{1292};
t6150 = ct{1293};
t6154 = ct{1294};
t6155 = ct{1295};
t6156 = ct{1296};
t6157 = ct{1297};
t6160 = ct{1298};
t6161 = ct{1299};
t6162 = ct{1300};
t6166 = ct{1301};
t6168 = ct{1302};
t6169 = ct{1303};
t6172 = ct{1304};
t6178 = ct{1305};
t6179 = ct{1306};
t6180 = ct{1307};
t6181 = ct{1308};
t6183 = ct{1309};
t6184 = ct{1310};
t6185 = ct{1311};
t6190 = ct{1312};
t6191 = ct{1313};
t6193 = ct{1314};
t6194 = ct{1315};
t6197 = ct{1316};
t6198 = ct{1317};
t6199 = ct{1318};
t6200 = ct{1319};
t6202 = ct{1320};
t6206 = ct{1321};
t6207 = ct{1322};
t6209 = ct{1323};
t6210 = ct{1324};
t6211 = ct{1325};
t6214 = ct{1326};
t6216 = ct{1327};
t6218 = ct{1328};
t6219 = ct{1329};
t6221 = ct{1330};
t6222 = ct{1331};
t6223 = ct{1332};
t6224 = ct{1333};
t6226 = ct{1334};
t6228 = ct{1335};
t6229 = ct{1336};
t6231 = ct{1337};
t6232 = ct{1338};
t6233 = ct{1339};
t6234 = ct{1340};
t6235 = ct{1341};
t6237 = ct{1342};
t6238 = ct{1343};
t6239 = ct{1344};
t6240 = ct{1345};
t6241 = ct{1346};
t6242 = ct{1347};
t6244 = ct{1348};
t6245 = ct{1349};
t6247 = ct{1350};
t6248 = ct{1351};
t6249 = ct{1352};
t6250 = ct{1353};
t6251 = ct{1354};
t6252 = ct{1355};
t6253 = ct{1356};
t6255 = ct{1357};
t6256 = ct{1358};
t6257 = ct{1359};
t6259 = ct{1360};
t6260 = ct{1361};
t6261 = ct{1362};
t6262 = ct{1363};
t6263 = ct{1364};
t6265 = ct{1365};
t6266 = ct{1366};
t6267 = ct{1367};
t6270 = ct{1368};
t6272 = ct{1369};
t6273 = ct{1370};
t6274 = ct{1371};
t6275 = ct{1372};
t6277 = ct{1373};
t6282 = ct{1374};
t6283 = ct{1375};
t6286 = ct{1376};
t6287 = ct{1377};
t6289 = ct{1378};
t6290 = ct{1379};
t6291 = ct{1380};
t6292 = ct{1381};
t6293 = ct{1382};
t6294 = ct{1383};
t6295 = ct{1384};
t6296 = ct{1385};
t6297 = ct{1386};
t6298 = ct{1387};
t6299 = ct{1388};
t6300 = ct{1389};
t6301 = ct{1390};
t6302 = ct{1391};
t6303 = ct{1392};
t6304 = ct{1393};
t6305 = ct{1394};
t6316 = ct{1395};
t6317 = ct{1396};
t6318 = ct{1397};
t6319 = ct{1398};
t6321 = ct{1399};
t6322 = ct{1400};
t6323 = ct{1401};
t6328 = ct{1402};
t6330 = ct{1403};
t6331 = ct{1404};
t6333 = ct{1405};
t6334 = ct{1406};
t6336 = ct{1407};
t6338 = ct{1408};
t6339 = ct{1409};
t6341 = ct{1410};
t6342 = ct{1411};
t6344 = ct{1412};
t6345 = ct{1413};
t6347 = ct{1414};
t6348 = ct{1415};
t6349 = ct{1416};
t6351 = ct{1417};
t6352 = ct{1418};
t6356 = ct{1419};
t6357 = ct{1420};
t6358 = ct{1421};
t6359 = ct{1422};
t6360 = ct{1423};
t6361 = ct{1424};
t6362 = ct{1425};
t6364 = ct{1426};
t6365 = ct{1427};
t6366 = ct{1428};
t6367 = ct{1429};
t6368 = ct{1430};
t6369 = ct{1431};
t6370 = ct{1432};
t6371 = ct{1433};
t6372 = ct{1434};
t6373 = ct{1435};
t6374 = ct{1436};
t6375 = ct{1437};
t6376 = ct{1438};
t6378 = ct{1439};
t6379 = ct{1440};
t6382 = ct{1441};
t6384 = ct{1442};
t6385 = ct{1443};
t6386 = ct{1444};
t6387 = ct{1445};
t6388 = ct{1446};
t6389 = ct{1447};
t6390 = ct{1448};
t6391 = ct{1449};
t6392 = ct{1450};
t6394 = ct{1451};
t6395 = ct{1452};
t6396 = ct{1453};
t6397 = ct{1454};
t6398 = ct{1455};
t6399 = ct{1456};
t6400 = ct{1457};
t6401 = ct{1458};
t6403 = ct{1459};
t6404 = ct{1460};
t6406 = ct{1461};
t6407 = ct{1462};
t6413 = ct{1463};
t6414 = ct{1464};
t6415 = ct{1465};
t6417 = ct{1466};
t6419 = ct{1467};
t642 = ct{1468};
t6420 = ct{1469};
t6421 = ct{1470};
t6422 = ct{1471};
t6423 = ct{1472};
t6424 = ct{1473};
t6425 = ct{1474};
t6427 = ct{1475};
t6429 = ct{1476};
t643 = ct{1477};
t6431 = ct{1478};
t6432 = ct{1479};
t6433 = ct{1480};
t6434 = ct{1481};
t6435 = ct{1482};
t6436 = ct{1483};
t6437 = ct{1484};
t6438 = ct{1485};
t6439 = ct{1486};
t6441 = ct{1487};
t6442 = ct{1488};
t6444 = ct{1489};
t6445 = ct{1490};
t6446 = ct{1491};
t6447 = ct{1492};
t6448 = ct{1493};
t6449 = ct{1494};
t6450 = ct{1495};
t6451 = ct{1496};
t6452 = ct{1497};
t6453 = ct{1498};
t6454 = ct{1499};
t6456 = ct{1500};
t6459 = ct{1501};
t6460 = ct{1502};
t6461 = ct{1503};
t6462 = ct{1504};
t6463 = ct{1505};
t6464 = ct{1506};
t6466 = ct{1507};
t6468 = ct{1508};
t6469 = ct{1509};
t6470 = ct{1510};
t6471 = ct{1511};
t6472 = ct{1512};
t6473 = ct{1513};
t6474 = ct{1514};
t6475 = ct{1515};
t6476 = ct{1516};
t6478 = ct{1517};
t6480 = ct{1518};
t6481 = ct{1519};
t6482 = ct{1520};
t6483 = ct{1521};
t6484 = ct{1522};
t6485 = ct{1523};
t6486 = ct{1524};
t6488 = ct{1525};
t6489 = ct{1526};
t649 = ct{1527};
t6490 = ct{1528};
t6491 = ct{1529};
t6492 = ct{1530};
t6493 = ct{1531};
t6494 = ct{1532};
t6495 = ct{1533};
t6496 = ct{1534};
t6497 = ct{1535};
t6499 = ct{1536};
t6501 = ct{1537};
t6504 = ct{1538};
t6505 = ct{1539};
t6507 = ct{1540};
t6508 = ct{1541};
t6509 = ct{1542};
t6510 = ct{1543};
t6511 = ct{1544};
t6512 = ct{1545};
t6515 = ct{1546};
t6518 = ct{1547};
t6519 = ct{1548};
t6521 = ct{1549};
t6522 = ct{1550};
t6523 = ct{1551};
t6524 = ct{1552};
t6525 = ct{1553};
t6526 = ct{1554};
t6527 = ct{1555};
t6528 = ct{1556};
t6529 = ct{1557};
t6532 = ct{1558};
t6533 = ct{1559};
t6534 = ct{1560};
t6535 = ct{1561};
t6537 = ct{1562};
t6540 = ct{1563};
t6541 = ct{1564};
t6543 = ct{1565};
t6544 = ct{1566};
t6545 = ct{1567};
t6546 = ct{1568};
t6547 = ct{1569};
t6549 = ct{1570};
t6551 = ct{1571};
t6553 = ct{1572};
t6556 = ct{1573};
t6559 = ct{1574};
t6560 = ct{1575};
t6561 = ct{1576};
t6562 = ct{1577};
t6563 = ct{1578};
t6565 = ct{1579};
t6566 = ct{1580};
t6568 = ct{1581};
t6570 = ct{1582};
t6571 = ct{1583};
t6572 = ct{1584};
t6574 = ct{1585};
t6577 = ct{1586};
t6578 = ct{1587};
t6583 = ct{1588};
t6584 = ct{1589};
t6585 = ct{1590};
t6586 = ct{1591};
t6587 = ct{1592};
t6588 = ct{1593};
t6591 = ct{1594};
t6592 = ct{1595};
t6593 = ct{1596};
t6595 = ct{1597};
t6596 = ct{1598};
t6597 = ct{1599};
t6598 = ct{1600};
t6599 = ct{1601};
t6600 = ct{1602};
t6601 = ct{1603};
t6603 = ct{1604};
t6604 = ct{1605};
t6605 = ct{1606};
t6608 = ct{1607};
t6609 = ct{1608};
t6610 = ct{1609};
t6611 = ct{1610};
t6612 = ct{1611};
t6613 = ct{1612};
t6614 = ct{1613};
t6617 = ct{1614};
t6620 = ct{1615};
t6621 = ct{1616};
t6623 = ct{1617};
t6625 = ct{1618};
t6626 = ct{1619};
t6628 = ct{1620};
t6636 = ct{1621};
t6638 = ct{1622};
t6639 = ct{1623};
t6641 = ct{1624};
t6642 = ct{1625};
t6643 = ct{1626};
t6644 = ct{1627};
t6645 = ct{1628};
t6649 = ct{1629};
t6650 = ct{1630};
t6651 = ct{1631};
t6656 = ct{1632};
t6657 = ct{1633};
t6658 = ct{1634};
t6660 = ct{1635};
t6663 = ct{1636};
t6664 = ct{1637};
t6665 = ct{1638};
t6668 = ct{1639};
t6669 = ct{1640};
t667 = ct{1641};
t6670 = ct{1642};
t6671 = ct{1643};
t6674 = ct{1644};
t6675 = ct{1645};
t6676 = ct{1646};
t6677 = ct{1647};
t6678 = ct{1648};
t6679 = ct{1649};
t6680 = ct{1650};
t6681 = ct{1651};
t6684 = ct{1652};
t6688 = ct{1653};
t6689 = ct{1654};
t6690 = ct{1655};
t6691 = ct{1656};
t6692 = ct{1657};
t6695 = ct{1658};
t6697 = ct{1659};
t670 = ct{1660};
t6701 = ct{1661};
t6702 = ct{1662};
t6703 = ct{1663};
t6704 = ct{1664};
t6705 = ct{1665};
t6707 = ct{1666};
t6709 = ct{1667};
t6710 = ct{1668};
t6711 = ct{1669};
t6712 = ct{1670};
t6713 = ct{1671};
t6715 = ct{1672};
t6716 = ct{1673};
t6720 = ct{1674};
t6722 = ct{1675};
t6725 = ct{1676};
t6726 = ct{1677};
t6727 = ct{1678};
t6729 = ct{1679};
t6730 = ct{1680};
t6731 = ct{1681};
t6732 = ct{1682};
t6734 = ct{1683};
t6735 = ct{1684};
t6737 = ct{1685};
t674 = ct{1686};
t6740 = ct{1687};
t6741 = ct{1688};
t6742 = ct{1689};
t6745 = ct{1690};
t6746 = ct{1691};
t6747 = ct{1692};
t6749 = ct{1693};
t6752 = ct{1694};
t6753 = ct{1695};
t6754 = ct{1696};
t6755 = ct{1697};
t6756 = ct{1698};
t6757 = ct{1699};
t6758 = ct{1700};
t6759 = ct{1701};
t6760 = ct{1702};
t6763 = ct{1703};
t6764 = ct{1704};
t6765 = ct{1705};
t6766 = ct{1706};
t6767 = ct{1707};
t6768 = ct{1708};
t6769 = ct{1709};
t6770 = ct{1710};
t6771 = ct{1711};
t6772 = ct{1712};
t6773 = ct{1713};
t6774 = ct{1714};
t6775 = ct{1715};
t6776 = ct{1716};
t6777 = ct{1717};
t6778 = ct{1718};
t6780 = ct{1719};
t6781 = ct{1720};
t6782 = ct{1721};
t6784 = ct{1722};
t6785 = ct{1723};
t6786 = ct{1724};
t6787 = ct{1725};
t6788 = ct{1726};
t6792 = ct{1727};
t6794 = ct{1728};
t6795 = ct{1729};
t6796 = ct{1730};
t6797 = ct{1731};
t6798 = ct{1732};
t6800 = ct{1733};
t6801 = ct{1734};
t6802 = ct{1735};
t6807 = ct{1736};
t6809 = ct{1737};
t6810 = ct{1738};
t6811 = ct{1739};
t6812 = ct{1740};
t6813 = ct{1741};
t6816 = ct{1742};
t6818 = ct{1743};
t6819 = ct{1744};
t6820 = ct{1745};
t6821 = ct{1746};
t6822 = ct{1747};
t6824 = ct{1748};
t6825 = ct{1749};
t6826 = ct{1750};
t6827 = ct{1751};
t6828 = ct{1752};
t6830 = ct{1753};
t6831 = ct{1754};
t6832 = ct{1755};
t6833 = ct{1756};
t6834 = ct{1757};
t6836 = ct{1758};
t6837 = ct{1759};
t6838 = ct{1760};
t6839 = ct{1761};
t684 = ct{1762};
t6840 = ct{1763};
t6841 = ct{1764};
t6843 = ct{1765};
t6844 = ct{1766};
t6845 = ct{1767};
t6846 = ct{1768};
t6848 = ct{1769};
t6849 = ct{1770};
t685 = ct{1771};
t6850 = ct{1772};
t6854 = ct{1773};
t6856 = ct{1774};
t6857 = ct{1775};
t686 = ct{1776};
t6860 = ct{1777};
t6861 = ct{1778};
t6863 = ct{1779};
t6864 = ct{1780};
t6865 = ct{1781};
t6866 = ct{1782};
t6868 = ct{1783};
t6869 = ct{1784};
t687 = ct{1785};
t6871 = ct{1786};
t6872 = ct{1787};
t6873 = ct{1788};
t6876 = ct{1789};
t6878 = ct{1790};
t6879 = ct{1791};
t6881 = ct{1792};
t6884 = ct{1793};
t6885 = ct{1794};
t6886 = ct{1795};
t6887 = ct{1796};
t6888 = ct{1797};
t6890 = ct{1798};
t6891 = ct{1799};
t6892 = ct{1800};
t6893 = ct{1801};
t6898 = ct{1802};
t6899 = ct{1803};
t6900 = ct{1804};
t6901 = ct{1805};
t6903 = ct{1806};
t6905 = ct{1807};
t6906 = ct{1808};
t6910 = ct{1809};
t6913 = ct{1810};
t6916 = ct{1811};
t6917 = ct{1812};
t6919 = ct{1813};
t6920 = ct{1814};
t6924 = ct{1815};
t6925 = ct{1816};
t6926 = ct{1817};
t6927 = ct{1818};
t6928 = ct{1819};
t6929 = ct{1820};
t6930 = ct{1821};
t6932 = ct{1822};
t6933 = ct{1823};
t6934 = ct{1824};
t6935 = ct{1825};
t6936 = ct{1826};
t6937 = ct{1827};
t6938 = ct{1828};
t6942 = ct{1829};
t6943 = ct{1830};
t6944 = ct{1831};
t6945 = ct{1832};
t6946 = ct{1833};
t6947 = ct{1834};
t6948 = ct{1835};
t6949 = ct{1836};
t6952 = ct{1837};
t6954 = ct{1838};
t6955 = ct{1839};
t6956 = ct{1840};
t6957 = ct{1841};
t6958 = ct{1842};
t6959 = ct{1843};
t6960 = ct{1844};
t6961 = ct{1845};
t6964 = ct{1846};
t6965 = ct{1847};
t6966 = ct{1848};
t6968 = ct{1849};
t6970 = ct{1850};
t6971 = ct{1851};
t6972 = ct{1852};
t6973 = ct{1853};
t6975 = ct{1854};
t6979 = ct{1855};
t6983 = ct{1856};
t6984 = ct{1857};
t6986 = ct{1858};
t6988 = ct{1859};
t6989 = ct{1860};
t6991 = ct{1861};
t6992 = ct{1862};
t6993 = ct{1863};
t6996 = ct{1864};
t6997 = ct{1865};
t6998 = ct{1866};
t6999 = ct{1867};
t7 = ct{1868};
t7003 = ct{1869};
t7010 = ct{1870};
t7011 = ct{1871};
t7012 = ct{1872};
t7013 = ct{1873};
t7014 = ct{1874};
t7015 = ct{1875};
t7016 = ct{1876};
t7018 = ct{1877};
t7019 = ct{1878};
t7020 = ct{1879};
t7021 = ct{1880};
t7024 = ct{1881};
t7029 = ct{1882};
t7030 = ct{1883};
t7035 = ct{1884};
t7036 = ct{1885};
t7037 = ct{1886};
t7038 = ct{1887};
t7039 = ct{1888};
t7040 = ct{1889};
t7041 = ct{1890};
t7050 = ct{1891};
t7051 = ct{1892};
t7053 = ct{1893};
t7054 = ct{1894};
t7055 = ct{1895};
t7056 = ct{1896};
t7057 = ct{1897};
t7058 = ct{1898};
t7060 = ct{1899};
t7061 = ct{1900};
t7068 = ct{1901};
t707 = ct{1902};
t7071 = ct{1903};
t7072 = ct{1904};
t7073 = ct{1905};
t7074 = ct{1906};
t7075 = ct{1907};
t7077 = ct{1908};
t7078 = ct{1909};
t7079 = ct{1910};
t708 = ct{1911};
t7080 = ct{1912};
t7081 = ct{1913};
t7082 = ct{1914};
t7084 = ct{1915};
t7085 = ct{1916};
t7087 = ct{1917};
t7089 = ct{1918};
t7091 = ct{1919};
t7093 = ct{1920};
t7094 = ct{1921};
t7097 = ct{1922};
t7098 = ct{1923};
t7099 = ct{1924};
t710 = ct{1925};
t7101 = ct{1926};
t7103 = ct{1927};
t7104 = ct{1928};
t7105 = ct{1929};
t7107 = ct{1930};
t7108 = ct{1931};
t7114 = ct{1932};
t7119 = ct{1933};
t7121 = ct{1934};
t7127 = ct{1935};
t7128 = ct{1936};
t7141 = ct{1937};
t7148 = ct{1938};
t7152 = ct{1939};
t7157 = ct{1940};
t7163 = ct{1941};
t7168 = ct{1942};
t7174 = ct{1943};
t7177 = ct{1944};
t7179 = ct{1945};
t7181 = ct{1946};
t7185 = ct{1947};
t7187 = ct{1948};
t7188 = ct{1949};
t7192 = ct{1950};
t7195 = ct{1951};
t7198 = ct{1952};
t7200 = ct{1953};
t7201 = ct{1954};
t7204 = ct{1955};
t7207 = ct{1956};
t7208 = ct{1957};
t7209 = ct{1958};
t721 = ct{1959};
t7210 = ct{1960};
t7211 = ct{1961};
t7215 = ct{1962};
t7219 = ct{1963};
t722 = ct{1964};
t7222 = ct{1965};
t7232 = ct{1966};
t7233 = ct{1967};
t7238 = ct{1968};
t7239 = ct{1969};
t724 = ct{1970};
t7240 = ct{1971};
t7245 = ct{1972};
t7248 = ct{1973};
t7257 = ct{1974};
t7259 = ct{1975};
t7263 = ct{1976};
t7264 = ct{1977};
t7265 = ct{1978};
t7271 = ct{1979};
t7277 = ct{1980};
t7278 = ct{1981};
t7281 = ct{1982};
t7282 = ct{1983};
t7283 = ct{1984};
t7288 = ct{1985};
t7290 = ct{1986};
t7292 = ct{1987};
t7293 = ct{1988};
t7294 = ct{1989};
t7295 = ct{1990};
t7296 = ct{1991};
t7297 = ct{1992};
t7298 = ct{1993};
t7302 = ct{1994};
t7303 = ct{1995};
t7304 = ct{1996};
t7305 = ct{1997};
t7308 = ct{1998};
t7309 = ct{1999};
t7314 = ct{2000};
t7315 = ct{2001};
t7316 = ct{2002};
t7317 = ct{2003};
t7325 = ct{2004};
t7326 = ct{2005};
t7349 = ct{2006};
t7350 = ct{2007};
t7353 = ct{2008};
t7364 = ct{2009};
t7365 = ct{2010};
t7369 = ct{2011};
t7370 = ct{2012};
t7371 = ct{2013};
t7375 = ct{2014};
t7376 = ct{2015};
t7377 = ct{2016};
t7378 = ct{2017};
t7394 = ct{2018};
t7407 = ct{2019};
t7427 = ct{2020};
t7429 = ct{2021};
t7430 = ct{2022};
t7453 = ct{2023};
t7454 = ct{2024};
t7455 = ct{2025};
t7459 = ct{2026};
t7461 = ct{2027};
t7470 = ct{2028};
t7471 = ct{2029};
t7472 = ct{2030};
t7473 = ct{2031};
t7478 = ct{2032};
t7479 = ct{2033};
t749 = ct{2034};
t7504 = ct{2035};
t7505 = ct{2036};
t7506 = ct{2037};
t7521 = ct{2038};
t7523 = ct{2039};
t7530 = ct{2040};
t7532 = ct{2041};
t7533 = ct{2042};
t7534 = ct{2043};
t7535 = ct{2044};
t7536 = ct{2045};
t7555 = ct{2046};
t7556 = ct{2047};
t7566 = ct{2048};
t7567 = ct{2049};
t7600 = ct{2050};
t7606 = ct{2051};
t762 = ct{2052};
t7637 = ct{2053};
t7665 = ct{2054};
t768 = ct{2055};
t7730 = ct{2056};
t7731 = ct{2057};
t7732 = ct{2058};
t7733 = ct{2059};
t7734 = ct{2060};
t7757 = ct{2061};
t7758 = ct{2062};
t777 = ct{2063};
t7790 = ct{2064};
t7791 = ct{2065};
t7811 = ct{2066};
t7813 = ct{2067};
t7815 = ct{2068};
t792 = ct{2069};
t7922 = ct{2070};
t7923 = ct{2071};
t7925 = ct{2072};
t7927 = ct{2073};
t793 = ct{2074};
t7952 = ct{2075};
t801 = ct{2076};
t802 = ct{2077};
t808 = ct{2078};
t813 = ct{2079};
t819 = ct{2080};
t821 = ct{2081};
t850 = ct{2082};
t855 = ct{2083};
t874 = ct{2084};
t878 = ct{2085};
t941 = ct{2086};
t948 = ct{2087};
t951 = ct{2088};
t7109 = t5710.*t6595;
t7111 = t5783.*t6561;
t7113 = t5757.*t6595;
t7122 = -t6561.*(t4610+t2363.*(t3547.*1.838876e-2+t4071-t4072+t34.*(t1896-t3232).*9.99471e-3).*7.26735e-3);
t7123 = t6561.*(t4610+t2363.*(t3547.*1.838876e-2+t4071-t4072+t34.*(t1896-t3232).*9.99471e-3).*7.26735e-3);
t7124 = t5800.*t6566;
t7125 = t5801.*t6566;
t7129 = t5895.*t6515;
t7130 = t5898.*t6515;
t7131 = -t6595.*(t5359+t4108.*(t1861-t3214));
t7132 = t6595.*(t5359+t4108.*(t1861-t3214));
t7133 = t6899.*(t4840-t34.*(t1005+t26.*(t1941-t3308+t39.*t1022.*(t855-t878).*2.196325630278387e-1)));
t7134 = t5293.*t6898;
t7135 = t5295.*t6898;
t7136 = -t6899.*(t4133-t4843);
t7138 = t5797.*t6595;
t7142 = t5800.*t6595;
t7150 = t5849.*t6561;
t7158 = t5895.*t6561;
t7166 = -t5800.*(t4795.*(t1896-t3232).*7.26735e-3+t2363.*(t684+t685-t710+t724+t1686-t1690+t1700+t1701+t2371+t2698+t2707-t2716+t2719+t3319-t3327-t3341-t3620+t3622+t3634-t3638+t4076+t4077).*7.26735e-3);
t7170 = -t5895.*(t4758.*(t1861-t3214)+t2297.*(t642+t643-t667+t674+t1587+t1606+t1608+t1609+t2295+t2671+t2683+t2684-t2695+t3272+t3290-t3296+t3576+t3582+t3588-t3593+t4015+t4016));
t7171 = t5895.*(t4758.*(t1861-t3214)+t2297.*(t642+t643-t667+t674+t1587+t1606+t1608+t1609+t2295+t2671+t2683+t2684-t2695+t3272+t3290-t3296+t3576+t3582+t3588-t3593+t4015+t4016));
t7175 = t5983.*t6595;
t7196 = t3210.*t7192;
t7202 = t3483.*t7192;
t7212 = t3877.*t7192;
t7216 = t3957.*t7192;
t7223 = t3385.*t7208;
t7224 = t3386.*t7207;
t7242 = t6595.*(-t2308+t2378+t2510-t2530-t2975+t2979+t3893+t4106+t4152+t4155+t4805+t4809);
t7249 = t6561.*t6565;
t7252 = t4510.*t7207;
t7253 = t4514.*t7208;
t7254 = t4541.*t7208;
t7255 = -t7207.*(t3544-t4013);
t7260 = t3763+t3764+t3766+t3778+t4926+t4932+t4944+t4945+t4952+t4953+t4958+t4959;
t7261 = t3755+t3771+t3772+t3775+t4929+t4930+t4939+t4948+t4950+t4954+t4956+t4960;
t7299 = t188.*t7298.*8.595599785252598e-1;
t7301 = t2338.*t7298;
t7330 = t6022+t6275+t6650;
t7336 = t3882.*t7325;
t7337 = -t7326.*(-t1901+t3122+t3270);
t7338 = t4080.*t7325;
t7340 = -t7326.*(t951+t16.*(-t1881+t3121+t3269));
t7359 = t4822.*t7325;
et327 = -t2306-t2317+t3144+t3147+t35.*t941.*t948.*(t850-t874).*3.775747223193135e-1;
et328 = t36.*t941.*t948.*(t850-t874).*2.244797987218524e-1;
t7361 = -t7326.*(et327+et328);
t7366 = t4984+t5225+t6233+t7061;
t7367 = t6069+t6394+t6769;
t7368 = t6072+t6400+t6768;
t7379 = -t7377;
et329 = t2363.*(t2368+t3330+t3563.*1.838876e-2-t3618+t3619+t27.*(t1896-t3232).*1.247162e-2+t33.*(t1896-t3232).*3.131399999999998e-4+t33.*t34.*(t1896-t3232).*9.99471e-3);
et330 = 7.26735e-3;
t7380 = -t6561.*(t4872+t5144+et329.*et330+t2388.*(t684+t685-t710+t724+t1686-t1690+t1700+t1701+t2371+t2698+t2707-t2716+t2719+t3319-t3327-t3341-t3620+t3622+t3634-t3638+t4076+t4077).*7.26735e-3);
et331 = t2363.*(t2368+t3330+t3563.*1.838876e-2-t3618+t3619+t27.*(t1896-t3232).*1.247162e-2+t33.*(t1896-t3232).*3.131399999999998e-4+t33.*t34.*(t1896-t3232).*9.99471e-3);
et332 = 7.26735e-3;
t7381 = t6561.*(t4872+t5144+et331.*et332+t2388.*(t684+t685-t710+t724+t1686-t1690+t1700+t1701+t2371+t2698+t2707-t2716+t2719+t3319-t3327-t3341-t3620+t3622+t3634-t3638+t4076+t4077).*7.26735e-3);
t7382 = -t3481.*(t6767+t6001.*(t1896-t3232)+t3985.*(t3424-t3437+t4552+t4556+t3942.*(t1896-t3232).*5.7e-7+t3946.*(t1896-t3232).*4.0e-8));
t7383 = -t3484.*(t6070-t6768+t3996.*(t3424-t3437+t4552+t4556+t3942.*(t1896-t3232).*5.7e-7+t3946.*(t1896-t3232).*4.0e-8));
t7384 = t3484.*(t6070-t6768+t3996.*(t3424-t3437+t4552+t4556+t3942.*(t1896-t3232).*5.7e-7+t3946.*(t1896-t3232).*4.0e-8));
t7386 = t3385.*t7369;
t7387 = t3386.*t7370;
t7404 = -t3882.*(t6767+t6001.*(t1896-t3232)+t3985.*(t3424-t3437+t4552+t4556+t3942.*(t1896-t3232).*5.7e-7+t3946.*(t1896-t3232).*4.0e-8));
t7405 = (-t1901+t3122+t3270).*(t6070-t6768+t3996.*(t3424-t3437+t4552+t4556+t3942.*(t1896-t3232).*5.7e-7+t3946.*(t1896-t3232).*4.0e-8));
t7410 = -t4080.*(t6767+t6001.*(t1896-t3232)+t3985.*(t3424-t3437+t4552+t4556+t3942.*(t1896-t3232).*5.7e-7+t3946.*(t1896-t3232).*4.0e-8));
t7411 = t4080.*(t6767+t6001.*(t1896-t3232)+t3985.*(t3424-t3437+t4552+t4556+t3942.*(t1896-t3232).*5.7e-7+t3946.*(t1896-t3232).*4.0e-8));
t7412 = (t951+t16.*(-t1881+t3121+t3269)).*(t6070-t6768+t3996.*(t3424-t3437+t4552+t4556+t3942.*(t1896-t3232).*5.7e-7+t3946.*(t1896-t3232).*4.0e-8));
t7418 = t4514.*t7369;
t7419 = t4510.*t7370;
t7420 = t4541.*t7369;
t7421 = -t7370.*(t3544-t4013);
t7431 = -t4822.*(t6767+t6001.*(t1896-t3232)+t3985.*(t3424-t3437+t4552+t4556+t3942.*(t1896-t3232).*5.7e-7+t3946.*(t1896-t3232).*4.0e-8));
et333 = -t2306-t2317+t3144+t3147+t35.*t941.*t948.*(t850-t874).*3.775747223193135e-1;
et334 = t36.*t941.*t948.*(t850-t874).*2.244797987218524e-1;
t7432 = (et333+et334).*(t6070-t6768+t3996.*(t3424-t3437+t4552+t4556+t3942.*(t1896-t3232).*5.7e-7+t3946.*(t1896-t3232).*4.0e-8));
t7435 = t6216+t6463+t6888;
t7444 = t7365.*(t2674-t2676+t3022-t3027).*(t1488+t1874+t2519+t2740+t2747+t3096+t3097);
t7446 = t3877.*(t4983-t5225-t6233+t7058).*(t1488+t1874+t2519+t2740+t2747+t3096+t3097);
t7481 = t6017+t6833+t6834;
t7507 = t5884.*t7353;
t7509 = t5888.*t7353;
t7515 = t5798.*t7365;
t7517 = t5799.*t7365;
t7519 = -t5800.*(t4983-t5225-t6233+t7058);
t7520 = -t5801.*(t4983-t5225-t6233+t7058);
t7522 = -t7521;
t7524 = -t7523;
t7548 = t5373+t6077+t6082+t6083+t6504;
t7563 = t3385.*t7555;
t7564 = t3386.*t7556;
t7573 = t4510.*t7556;
t7574 = t4514.*t7555;
t7577 = t4541.*t7555;
t7578 = -t7556.*(t3544-t4013);
t7579 = t6595.*t7353;
t7583 = t6561.*t7365;
t7586 = -t7353.*(t4795.*(t1896-t3232).*7.26735e-3+t2363.*(t684+t685-t710+t724+t1686-t1690+t1700+t1701+t2371+t2698+t2707-t2716+t2719+t3319-t3327-t3341-t3620+t3622+t3634-t3638+t4076+t4077).*7.26735e-3);
t7589 = -t7365.*(t4758.*(t1861-t3214)+t2297.*(t642+t643-t667+t674+t1587+t1606+t1608+t1609+t2295+t2671+t2683+t2684-t2695+t3272+t3290-t3296+t3576+t3582+t3588-t3593+t4015+t4016));
t7590 = t7365.*(t4758.*(t1861-t3214)+t2297.*(t642+t643-t667+t674+t1587+t1606+t1608+t1609+t2295+t2671+t2683+t2684-t2695+t3272+t3290-t3296+t3576+t3582+t3588-t3593+t4015+t4016));
t7591 = t6595.*t7371;
t7596 = t5502+t6262+t6265+t6266+t6583;
et335 = t5031-t7091+t4795.*(t1005+t26.*(t1941-t3308+t39.*t1022.*(t855-t878).*2.196325630278387e-1)).*7.26735e-3;
et336 = t2419.*(t684+t685-t710+t724+t1686-t1690+t1700+t1701+t2371+t2698+t2707-t2716+t2719+t3319-t3327-t3341-t3620+t3622+t3634-t3638+t4076+t4077).*7.26735e-3;
t7597 = -t6561.*(et335+et336);
t7602 = t5495+t6267+t6272+t6274+t6651;
t7603 = -t3209.*(t6259-t6578+t5329.*(t1896-t3232)+t6035.*(t3235-t3535)+t6037.*(t3235-t3535));
t7604 = t3209.*(t6259-t6578+t5329.*(t1896-t3232)+t6035.*(t3235-t3535)+t6037.*(t3235-t3535));
t7607 = (t1861-t3214).*(t6259-t6578+t5329.*(t1896-t3232)+t6035.*(t3235-t3535)+t6037.*(t3235-t3535));
t7611 = (t2674-t2676+t3022-t3027).*(t6259-t6578+t5329.*(t1896-t3232)+t6035.*(t3235-t3535)+t6037.*(t3235-t3535));
t7615 = t5761+t5794+t5927+t6055+t6162+t6488;
t7622 = t50.*t189.*(t5563+t6360+t6361+t6362+t6795).*(-9.543032792050485e-17);
t7623 = -t2297.*(t5563+t6360+t6361+t6362+t6795);
t7624 = t5613+t6395+t6396+t6398+t6766;
t7638 = t5805+t5916+t5981+t6149+t6344+t6532;
t7649 = t5696+t6454+t6456+t6461+t6885;
t7650 = t5698+t6460+t6462+t6464+t6890;
t7735 = t5996+t6021+t6125+t6349+t6533+t6776;
t7754 = -t3209.*(-t5772-t5773+t6522+t6523+t28.*t6620.*(t3235-t3535)+t34.*t6617.*(t3235-t3535));
t7759 = (t1861-t3214).*(-t5772-t5773+t6522+t6523+t28.*t6620.*(t3235-t3535)+t34.*t6617.*(t3235-t3535));
t7766 = (t2674-t2676+t3022-t3027).*(-t5772-t5773+t6522+t6523+t28.*t6620.*(t3235-t3535)+t34.*t6617.*(t3235-t3535));
t7767 = t3209.*t7757;
t7770 = t3210.*t7758;
t7771 = -t3946.*(-t5772-t5773+t6522+t6523+t28.*t6620.*(t3235-t3535)+t34.*t6617.*(t3235-t3535));
t7772 = t3946.*(-t5772-t5773+t6522+t6523+t28.*t6620.*(t3235-t3535)+t34.*t6617.*(t3235-t3535));
t7774 = -t7757.*(t1861-t3214);
t7775 = t3483.*t7758;
t7781 = -t7757.*(t2674-t2676+t3022-t3027);
t7782 = t3877.*t7758;
t7792 = t6025+t6211+t6625+t6873+t7018+t7222;
et337 = t6023+t6210-t6625+t6986.*(t1477-t2502)+t3057.*(t3130+t3131+t3170+t3435-t4238-t4239-t4257+t4259-t4264+t4266-t4520-t4531+t4560+t4576+t2388.*(t1456-t2355).*4.0e-8+(t3524.*(t1861-t3214))./1.0e+8+(t3481.*(t1896-t3232))./1.0e+8-t17.*t2297.*t2363.*2.4e-7);
et338 = t2363.*(t3156+t3157+t3376-t4255-t4256-t4499+t4504+t3524.*(t1861-t3214).*6.2e-7+t3481.*(t1896-t3232).*6.2e-7-(t17.*(t1861-t3214).*(t1896-t3232))./1.0e+8-(t17.*t2297.*t2363)./1.0e+8-(t17.*t3483.*t3528)./1.0e+8);
t7793 = t50.*t189.*(et337+et338).*(-9.543032792050485e-17);
et339 = t6023+t6210-t6625+t6986.*(t1477-t2502)+t3057.*(t3130+t3131+t3170+t3435-t4238-t4239-t4257+t4259-t4264+t4266-t4520-t4531+t4560+t4576+t2388.*(t1456-t2355).*4.0e-8+(t3524.*(t1861-t3214))./1.0e+8+(t3481.*(t1896-t3232))./1.0e+8-t17.*t2297.*t2363.*2.4e-7);
et340 = t2363.*(t3156+t3157+t3376-t4255-t4256-t4499+t4504+t3524.*(t1861-t3214).*6.2e-7+t3481.*(t1896-t3232).*6.2e-7-(t17.*(t1861-t3214).*(t1896-t3232))./1.0e+8-(t17.*t2297.*t2363)./1.0e+8-(t17.*t3483.*t3528)./1.0e+8);
t7794 = t50.*t189.*(et339+et340).*9.543032792050485e-17;
et341 = t6023+t6210-t6625+t6986.*(t1477-t2502)+t3057.*(t3130+t3131+t3170+t3435-t4238-t4239-t4257+t4259-t4264+t4266-t4520-t4531+t4560+t4576+t2388.*(t1456-t2355).*4.0e-8+(t3524.*(t1861-t3214))./1.0e+8+(t3481.*(t1896-t3232))./1.0e+8-t17.*t2297.*t2363.*2.4e-7);
et342 = t2363.*(t3156+t3157+t3376-t4255-t4256-t4499+t4504+t3524.*(t1861-t3214).*6.2e-7+t3481.*(t1896-t3232).*6.2e-7-(t17.*(t1861-t3214).*(t1896-t3232))./1.0e+8-(t17.*t2297.*t2363)./1.0e+8-(t17.*t3483.*t3528)./1.0e+8);
t7795 = -t2297.*(et341+et342);
t7808 = t6068+t6330+t6704+t6927+t7097+t7238;
t7809 = t6071+t6331+t6705+t6928+t7098+t7239;
t7853 = t5929+t6073+t6494+t7177+t7248+t7364;
et343 = t3681+t3684-t3834+t4849+t4857-t5104+t5105-t5136+t3360.*(t1477-t2502).*9.3e-7+t3996.*(t3493-t3972).*9.0e-8+t18.*t3946.*(t3235-t3535).*9.0e-8;
et344 = t23.*t3946.*(t3235-t3535).*9.3e-7;
et345 = t3209;
et346 = -t5877-t6660+t4514.*(et343+et344)+t4510.*(t3680+t3685-t3827+t4848+t4856-t5103+t5111-t5140+t18.*t4833+t3360.*(t1477-t2502).*9.0e-8+t3996.*(t3493-t3972).*1.02e-6+t23.*t3946.*(t3235-t3535).*9.0e-8)+t28.*t6899.*(t3235-t3535)+t34.*t6898.*(t3235-t3535);
et347 = -1.0;
t7876 = et345.*et346.*et347;
et348 = t3681+t3684-t3834+t4849+t4857-t5104+t5105-t5136+t3360.*(t1477-t2502).*9.3e-7+t3996.*(t3493-t3972).*9.0e-8+t18.*t3946.*(t3235-t3535).*9.0e-8;
et349 = t23.*t3946.*(t3235-t3535).*9.3e-7;
et350 = t1861-t3214;
et351 = -t5877-t6660+t4514.*(et348+et349)+t4510.*(t3680+t3685-t3827+t4848+t4856-t5103+t5111-t5140+t18.*t4833+t3360.*(t1477-t2502).*9.0e-8+t3996.*(t3493-t3972).*1.02e-6+t23.*t3946.*(t3235-t3535).*9.0e-8)+t28.*t6899.*(t3235-t3535)+t34.*t6898.*(t3235-t3535);
t7878 = et350.*et351;
et352 = t3681+t3684-t3834+t4849+t4857-t5104+t5105-t5136+t3360.*(t1477-t2502).*9.3e-7+t3996.*(t3493-t3972).*9.0e-8+t18.*t3946.*(t3235-t3535).*9.0e-8;
et353 = t23.*t3946.*(t3235-t3535).*9.3e-7;
et354 = t2674-t2676+t3022-t3027;
et355 = -t5877-t6660+t4514.*(et352+et353)+t4510.*(t3680+t3685-t3827+t4848+t4856-t5103+t5111-t5140+t18.*t4833+t3360.*(t1477-t2502).*9.0e-8+t3996.*(t3493-t3972).*1.02e-6+t23.*t3946.*(t3235-t3535).*9.0e-8)+t28.*t6899.*(t3235-t3535)+t34.*t6898.*(t3235-t3535);
t7882 = et354.*et355;
et356 = t3681+t3684-t3834+t4849+t4857-t5104+t5105-t5136+t3360.*(t1477-t2502).*9.3e-7+t3996.*(t3493-t3972).*9.0e-8+t18.*t3946.*(t3235-t3535).*9.0e-8;
et357 = t23.*t3946.*(t3235-t3535).*9.3e-7;
et358 = t3946;
et359 = -t5877-t6660+t4514.*(et356+et357)+t4510.*(t3680+t3685-t3827+t4848+t4856-t5103+t5111-t5140+t18.*t4833+t3360.*(t1477-t2502).*9.0e-8+t3996.*(t3493-t3972).*1.02e-6+t23.*t3946.*(t3235-t3535).*9.0e-8)+t28.*t6899.*(t3235-t3535)+t34.*t6898.*(t3235-t3535);
et360 = -1.0;
t7886 = et358.*et359.*et360;
t7890 = t6043+t6434+t6756+t7187+t7264+t7378;
t7892 = -t3209.*(-t6434+t7263+t7376+t5854.*(t1005+t26.*(t1941-t3308+t39.*t1022.*(t855-t878).*2.196325630278387e-1))+t6473.*(t4127+t33.*(t1959-t3306+t38.*t1022.*(t855-t878).*2.196325630278387e-1))+t7174.*(t1896-t3232));
t7893 = t3209.*(-t6434+t7263+t7376+t5854.*(t1005+t26.*(t1941-t3308+t39.*t1022.*(t855-t878).*2.196325630278387e-1))+t6473.*(t4127+t33.*(t1959-t3306+t38.*t1022.*(t855-t878).*2.196325630278387e-1))+t7174.*(t1896-t3232));
t7895 = (t1861-t3214).*(-t6434+t7263+t7376+t5854.*(t1005+t26.*(t1941-t3308+t39.*t1022.*(t855-t878).*2.196325630278387e-1))+t6473.*(t4127+t33.*(t1959-t3306+t38.*t1022.*(t855-t878).*2.196325630278387e-1))+t7174.*(t1896-t3232));
t7897 = (t2674-t2676+t3022-t3027).*(-t6434+t7263+t7376+t5854.*(t1005+t26.*(t1941-t3308+t39.*t1022.*(t855-t878).*2.196325630278387e-1))+t6473.*(t4127+t33.*(t1959-t3306+t38.*t1022.*(t855-t878).*2.196325630278387e-1))+t7174.*(t1896-t3232));
t7899 = t6024+t6244+t6636+t7198+t7271+t7427;
t7915 = t6180+t6518+t6906+t7210+t7281+t7454;
t7916 = t6181+t6519+t6903+t7211+t7283+t7455;
t7924 = -t3210.*(t6179-t6903-t7211+t7282+t7453+t4824.*(t3424-t3437+t4552+t4556+t3942.*(t1896-t3232).*5.7e-7+t3946.*(t1896-t3232).*4.0e-8));
t7926 = -t3483.*(t6179-t6903-t7211+t7282+t7453+t4824.*(t3424-t3437+t4552+t4556+t3942.*(t1896-t3232).*5.7e-7+t3946.*(t1896-t3232).*4.0e-8));
t7928 = -t7927;
t7929 = -t3877.*(t6179-t6903-t7211+t7282+t7453+t4824.*(t3424-t3437+t4552+t4556+t3942.*(t1896-t3232).*5.7e-7+t3946.*(t1896-t3232).*4.0e-8));
t7930 = t3877.*(t6179-t6903-t7211+t7282+t7453+t4824.*(t3424-t3437+t4552+t4556+t3942.*(t1896-t3232).*5.7e-7+t3946.*(t1896-t3232).*4.0e-8));
t7962 = t6347+t6574+t6992+t7294+t7350+t7567;
t5364 = -t5363;
t5758 = t4405+t5355;
t5784 = t4436+t5376;
t5803 = t4613+t5401;
t6090 = -t6089;
t6109 = -t6108;
t6111 = -t6110;
t6132 = -t6131;
t6134 = -t6133;
t6227 = -t6226;
t6230 = -t6228;
t6236 = t3877.*(t4612-t5401).*(t1488+t1874+t2519+t2740+t2747+t3096+t3097);
t6320 = -t6319;
t6335 = -t6334;
t6337 = -t6336;
t6353 = -t6352;
t6377 = -t6376;
t6380 = -t6379;
t6428 = -t6425;
t6430 = -t6429;
t6477 = -t6476;
t6479 = -t6478;
t6500 = -t6499;
t6502 = -t6501;
t6536 = -t6535;
t6538 = -t6537;
t6542 = -t6541;
t6548 = t3385.*t6509;
t6552 = -t6549;
t6554 = t3386.*t6512;
t6555 = -t6551;
t6557 = -t6553;
t6564 = t4995+t6197;
t6606 = t5014+t6255;
t6622 = -t6621;
t6624 = -t6623;
t6627 = -t6626;
t6629 = -t6628;
t6631 = t5063+t6290;
t6647 = -t6643;
t6648 = -t6644;
t6652 = -t5800.*(t4612-t5401);
t6653 = t5800.*(t4612-t5401);
t6654 = -t5801.*(t4612-t5401);
t6655 = t5801.*(t4612-t5401);
t6659 = -t6657;
t6667 = -t6665;
t6672 = -t6670;
t6673 = -t6671;
t6682 = -t6678;
t6683 = -t6679;
t6685 = -t6680;
t6686 = -t6681;
t6687 = -t6684;
t6696 = t5147+t6316;
t6698 = -t6695;
t6700 = -t6697;
t6714 = -t6709;
t6717 = -t6715;
t6728 = -t6726;
t6733 = -t6732;
t6736 = -t6735;
t6738 = t4514.*t6509;
t6739 = t4510.*t6512;
t6743 = t4541.*t6509;
t6744 = -t6742;
t6748 = -t6512.*(t3544-t4013);
t6750 = -t6747;
t6761 = -t6759;
t6762 = -t6760;
t6779 = -t6778;
t6783 = -t6782;
t6799 = -t6798;
t6803 = -t6802;
t6823 = -t6819;
t6842 = -t6836;
t6870 = -t6869;
t6880 = -t6879;
t6882 = -t6881;
t6902 = -t6901;
t6939 = -t6938;
t6950 = -t6947;
t6951 = -t6948;
t6953 = -t6949;
t6962 = -t6961;
t6969 = -t6965;
t7000 = -t6998;
t7001 = -t6999;
t7022 = -t7020;
t7023 = -t7021;
t7076 = -t7072;
t7139 = -t7138;
t7159 = -t7158;
t7183 = t4788+t5076+t5665+t6291;
t7190 = t4875+t5149+t5704+t6318;
t7203 = -t7202;
t7225 = -t7224;
t7234 = t3901.*(t4786+t5069-t5665-t6291).*(t1513+t1879+t2598+t2820+t2834+t3117+t3118).*7.26735e-3;
t7246 = t3877.*(t4874+t5148-t5704-t6318).*(t1488+t1874+t2519+t2740+t2747+t3096+t3097);
t7250 = -t7249;
t7266 = t3385.*t7261;
t7268 = t3386.*t7260;
t7284 = t4510.*t7260;
t7285 = t4514.*t7261;
t7286 = t4541.*t7261;
t7287 = -t7260.*(t3544-t4013);
t7300 = -t7299;
t7306 = -t5800.*(t4874+t5148-t5704-t6318);
t7307 = -t5801.*(t4874+t5148-t5704-t6318);
t7310 = -t5895.*(t4786+t5069-t5665-t6291);
t7311 = t5895.*(t4786+t5069-t5665-t6291);
t7312 = -t5898.*(t4786+t5069-t5665-t6291);
t7313 = t5898.*(t4786+t5069-t5665-t6291);
t7331 = t188.*t7330.*8.595599785252598e-1;
t7333 = t2307.*t7330;
t7334 = t2338.*t7330;
t7339 = -t7338;
t7342 = t188.*(-t6677+t6681+t3057.*(-t3423+t4543+t3946.*(t1896-t3232).*1.02e-6)).*(-8.595599785252598e-1);
t7343 = t188.*(-t6677+t6681+t3057.*(-t3423+t4543+t3946.*(t1896-t3232).*1.02e-6)).*8.595599785252598e-1;
t7344 = -t2307.*(-t6677+t6681+t3057.*(-t3423+t4543+t3946.*(t1896-t3232).*1.02e-6));
t7345 = -t17.*t2297.*(-t6677+t6681+t3057.*(-t3423+t4543+t3946.*(t1896-t3232).*1.02e-6));
t7346 = t2307.*(-t6677+t6681+t3057.*(-t3423+t4543+t3946.*(t1896-t3232).*1.02e-6));
t7347 = -t2338.*(-t6677+t6681+t3057.*(-t3423+t4543+t3946.*(t1896-t3232).*1.02e-6));
t7351 = -t2994.*(-t6677+t6681+t3057.*(-t3423+t4543+t3946.*(t1896-t3232).*1.02e-6));
t7354 = t4962+t5202+t6193+t7029;
t7360 = -t7359;
t7362 = t5653+t6740+t6741;
t7363 = t5651+t6745+t6749;
t7372 = t4998+t5257+t6292+t7051;
t7388 = -t7387;
t7416 = t5741+t6820+t6822;
t7417 = t5748+t6826+t6830;
t7433 = -t7432;
t7440 = t5778+t6838+t6840;
t7443 = t5777+t6844+t6849;
t7445 = -t7444;
t7447 = -t7446;
t7482 = t7.*t7481;
t7508 = -t7507;
t7510 = -t7509;
t7516 = -t7515;
t7518 = -t7517;
t7539 = t5882+t7073+t7075;
t7540 = t5881+t7080+t7084;
t7549 = t50.*t189.*t7548.*9.543032792050485e-17;
t7550 = t2297.*t7548;
t7565 = -t7564;
t7575 = -t7573;
t7576 = -t7574;
t7580 = -t7579;
t7584 = -t7583;
t7595 = t5501+t6260+t6261+t6263+t6578;
t7605 = t3210.*t7596;
t7610 = t3483.*t7596;
t7612 = -t7611;
t7613 = t3877.*t7596;
t7621 = t5568+t6357+t6358+t6364+t6794;
t7625 = t5614+t6397+t6399+t6401+t6771;
t7626 = t5435+t5439+t6120+t6121+t6535+t6537;
t7631 = t5977+t6417+t6420+t6466+t6469;
t7632 = t5977+t6419+t6421+t6466+t6469;
t7633 = t5977+t6417+t6420+t6468+t6470;
t7635 = t5977+t6419+t6421+t6468+t6470;
t7652 = t3209.*t7649;
t7655 = t3210.*t7650;
t7657 = -t7649.*(t1861-t3214);
t7658 = t7649.*(t1861-t3214);
t7659 = t3483.*t7650;
t7663 = -t7649.*(t2674-t2676+t3022-t3027);
t7664 = t7649.*(t2674-t2676+t3022-t3027);
t7666 = t3877.*t7650;
t7670 = t5529+t5530+t6302+t6305+t6643+t6644;
t7676 = t5650+t5652+t6368+t6369+t6639+t6642;
t7677 = t5656+t5657+t6370+t6371+t6638+t6641;
t7680 = t5623+t5625+t6390+t6391+t6675+t6676;
t7682 = -t3210.*(t5654+t5655-t6370-t6638-t6641+t6039.*(t3544-t4013));
t7683 = t50.*t189.*(t6389-t6391-t6675-t6676+t3057.*(t4752+t3942.*(t2694-t2701+t3036-t3043).*1.02e-6)+t5520.*(t1477-t2502)).*(-9.543032792050485e-17);
t7684 = t50.*t189.*(t6389-t6391-t6675-t6676+t3057.*(t4752+t3942.*(t2694-t2701+t3036-t3043).*1.02e-6)+t5520.*(t1477-t2502)).*9.543032792050485e-17;
t7685 = -t2297.*(t6389-t6391-t6675-t6676+t3057.*(t4752+t3942.*(t2694-t2701+t3036-t3043).*1.02e-6)+t5520.*(t1477-t2502));
t7686 = t2297.*(t6389-t6391-t6675-t6676+t3057.*(t4752+t3942.*(t2694-t2701+t3036-t3043).*1.02e-6)+t5520.*(t1477-t2502));
t7689 = -t3483.*(t5654+t5655-t6370-t6638-t6641+t6039.*(t3544-t4013));
t7691 = t6827+t6828+t6831+t6832;
t7692 = -t3047.*(t6389-t6391-t6675-t6676+t3057.*(t4752+t3942.*(t2694-t2701+t3036-t3043).*1.02e-6)+t5520.*(t1477-t2502));
t7698 = -t3877.*(t5654+t5655-t6370-t6638-t6641+t6039.*(t3544-t4013));
t7699 = t3877.*(t5654+t5655-t6370-t6638-t6641+t6039.*(t3544-t4013));
t7703 = -t3957.*(t5654+t5655-t6370-t6638-t6641+t6039.*(t3544-t4013));
t7710 = t6845+t6846+t6848+t6850;
t7736 = t50.*t189.*t7735.*9.543032792050485e-17;
t7738 = t2297.*t7735;
t7739 = t5742+t5746+t6480+t6481+t6757+t6758;
t7741 = t6964+t6966+t6968+t6971;
t7743 = -t7.*(-t5515-t6054+t6147+t6956+t6961+t17.*t3483.*(t4311-t5186+t4541.*(-t2804+t2838+t3109+t23.*(t1456-t2355).*9.3e-7)));
t7744 = t7.*(-t5515-t6054+t6147+t6956+t6961+t17.*t3483.*(t4311-t5186+t4541.*(-t2804+t2838+t3109+t23.*(t1456-t2355).*9.3e-7))).*(-1.0./2.0);
t7745 = t5933+t5934+t6273+t6283+t6816+t6818;
t7746 = t5933+t5934+t6277+t6287+t6816+t6818;
t7747 = t5557+t6031+t6257+t6270+t6943+t6945;
et361 = t6030-t6943-t6945+t3942.*(t4510.*(t2813-t2835+t18.*(t1456-t2355).*1.02e-6+t23.*(t1456-t2355).*9.0e-8)+t4514.*(-t2804+t2838+t3109+t23.*(t1456-t2355).*9.3e-7)+t3132.*(t3235-t3535))+t5489.*(t1456-t2355);
et362 = t3967.*(t4311-t5186+t4541.*(-t2804+t2838+t3109+t23.*(t1456-t2355).*9.3e-7));
t7748 = -t7.*(et361+et362);
et363 = t6030-t6943-t6945+t3942.*(t4510.*(t2813-t2835+t18.*(t1456-t2355).*1.02e-6+t23.*(t1456-t2355).*9.0e-8)+t4514.*(-t2804+t2838+t3109+t23.*(t1456-t2355).*9.3e-7)+t3132.*(t3235-t3535))+t5489.*(t1456-t2355);
et364 = t3967.*(t4311-t5186+t4541.*(-t2804+t2838+t3109+t23.*(t1456-t2355).*9.3e-7));
t7749 = t7.*(et363+et364).*(-1.0./2.0);
t7750 = t5772+t5773+t6524+t6525+t6784+t6785;
t7751 = t5776+t5781+t6526+t6527+t6786+t6787;
t7762 = -t3210.*(t5582+t5715-t6598-t6801+t6802+t6413.*(t3544-t4013));
t7765 = -t3483.*(t5582+t5715-t6598-t6801+t6802+t6413.*(t3544-t4013));
t7768 = -t7767;
t7778 = -t3877.*(t5582+t5715-t6598-t6801+t6802+t6413.*(t3544-t4013));
t7780 = -t3957.*(t5582+t5715-t6598-t6801+t6802+t6413.*(t3544-t4013));
t7784 = t7078+t7081+t7082+t7085;
t7787 = t5535+t6198+t6431+t6433+t7215+t7216;
t7803 = t3734+t3735+t4227+t4228+t4321+t4322+t5750+t5936+t5939+t5987+t5990+t6382+t6385+t6446+t6448;
t7804 = t3734+t3735+t4227+t4228+t4321+t4322+t5750+t5938+t5940+t5987+t5990+t6384+t6386+t6446+t6448;
t7805 = t3734+t3735+t4227+t4228+t4321+t4322+t5750+t5936+t5939+t5989+t5991+t6382+t6385+t6447+t6449;
t7806 = t3734+t3735+t4227+t4228+t4321+t4322+t5750+t5938+t5940+t5989+t5991+t6384+t6386+t6447+t6449;
t7807 = t5597+t5602+t5617+t5619+t5858+t5863+t5874+t5886+t6224+t6231+t6250+t6256;
t7812 = t3210.*t7809;
t7814 = t3483.*t7809;
t7816 = t3877.*t7809;
t7819 = -t3209.*(t5632+t6778-t6780-t7252-t7253+t6008.*(t3235-t3535));
t7820 = -t3210.*(t6191-t6781+t6782-t7254+t7207.*(t3544-t4013)+t27.*t3528.*(-t3423+t4543+t3946.*(t1896-t3232).*1.02e-6));
t7821 = (t1861-t3214).*(t5632+t6778-t6780-t7252-t7253+t6008.*(t3235-t3535));
t7823 = -t3483.*(t6191-t6781+t6782-t7254+t7207.*(t3544-t4013)+t27.*t3528.*(-t3423+t4543+t3946.*(t1896-t3232).*1.02e-6));
t7824 = (t2674-t2676+t3022-t3027).*(t5632+t6778-t6780-t7252-t7253+t6008.*(t3235-t3535));
t7826 = -t3877.*(t6191-t6781+t6782-t7254+t7207.*(t3544-t4013)+t27.*t3528.*(-t3423+t4543+t3946.*(t1896-t3232).*1.02e-6));
t7827 = -t3946.*(t5632+t6778-t6780-t7252-t7253+t6008.*(t3235-t3535));
t7828 = t3946.*(t5632+t6778-t6780-t7252-t7253+t6008.*(t3235-t3535));
t7829 = -t3957.*(t6191-t6781+t6782-t7254+t7207.*(t3544-t4013)+t27.*t3528.*(-t3423+t4543+t3946.*(t1896-t3232).*1.02e-6));
t7830 = t3957.*(t6191-t6781+t6782-t7254+t7207.*(t3544-t4013)+t27.*t3528.*(-t3423+t4543+t3946.*(t1896-t3232).*1.02e-6));
t7840 = t5788+t6545+t6929+t6930+t7288+t7290;
et365 = t50.*t189.*(t6929+t6930+t7288+t7290-t5739.*(t1477-t2502)-t3057.*(t4819+t4850+t4851+t3057.*(t1456-t2355).*1.02e-6+t3047.*(t1477-t2502).*1.02e-6+t3942.*(t3235-t3535).*1.02e-6));
et366 = 9.543032792050485e-17;
t7841 = et365.*et366;
t7843 = t2297.*(t6929+t6930+t7288+t7290-t5739.*(t1477-t2502)-t3057.*(t4819+t4850+t4851+t3057.*(t1456-t2355).*1.02e-6+t3047.*(t1477-t2502).*1.02e-6+t3942.*(t3235-t3535).*1.02e-6));
t7844 = t3047.*(t6929+t6930+t7288+t7290-t5739.*(t1477-t2502)-t3057.*(t4819+t4850+t4851+t3057.*(t1456-t2355).*1.02e-6+t3047.*(t1477-t2502).*1.02e-6+t3942.*(t3235-t3535).*1.02e-6));
t7854 = t50.*t189.*t7853.*9.543032792050485e-17;
t7856 = t2297.*t7853;
t7868 = t3560+t3790+t3791+t3861+t3862+t4154+t4898+t5533+t5536+t5659+t5662+t5844+t5848+t5946+t5948+t6018+t6373+t6376+t6423+t6425;
t7874 = t5877+t6660+t6996+t6997+t7314+t7315;
t7879 = -t7878;
t7891 = t6044+t6435+t6755+t7188+t7265+t7379;
t7900 = t50.*t189.*t7899.*9.543032792050485e-17;
t7902 = t2297.*t7899;
t7909 = t5829+t6712+t6946+t6952+t7420+t7421;
t7931 = t5615+t6701+t6702+t6955+t7504+t7506;
t7933 = t5902+t6796+t7011+t7014+t7470+t7471;
t7934 = t5899+t6797+t7013+t7016+t7472+t7473;
t7953 = t5957+t7012+t7035+t7037+t7532+t7533;
t7954 = t5956+t7015+t7036+t7038+t7535+t7536;
t7967 = t6046+t7104+t7134+t7136+t7577+t7578;
t7968 = -t3209.*(t7101-t7133-t7135+t7573+t7574+t5739.*(t4127+t33.*(t1959-t3306+t38.*t1022.*(t855-t878).*2.196325630278387e-1)));
t7969 = t3209.*(t7101-t7133-t7135+t7573+t7574+t5739.*(t4127+t33.*(t1959-t3306+t38.*t1022.*(t855-t878).*2.196325630278387e-1)));
t7971 = (t1861-t3214).*(t7101-t7133-t7135+t7573+t7574+t5739.*(t4127+t33.*(t1959-t3306+t38.*t1022.*(t855-t878).*2.196325630278387e-1)));
t7973 = (t2674-t2676+t3022-t3027).*(t7101-t7133-t7135+t7573+t7574+t5739.*(t4127+t33.*(t1959-t3306+t38.*t1022.*(t855-t878).*2.196325630278387e-1)));
t7975 = -t3946.*(t7101-t7133-t7135+t7573+t7574+t5739.*(t4127+t33.*(t1959-t3306+t38.*t1022.*(t855-t878).*2.196325630278387e-1)));
t7976 = t3946.*(t7101-t7133-t7135+t7573+t7574+t5739.*(t4127+t33.*(t1959-t3306+t38.*t1022.*(t855-t878).*2.196325630278387e-1)));
t7989 = t2963+t2964+t3664+t3665+t3744+t3794+t3872+t3922+t4201+t4243+t4400+t4406+t4428+t4429+t4599+t4602+t4641+t4645+t5191+t6064+t6067+t6092+t6096+t6570+t6572+t6591+t6593+t7121+t7125+t7128+t7130;
t7990 = t2963+t2964+t3664+t3665+t3744+t3794+t3872+t3922+t4201+t4243+t4400+t4406+t4428+t4429+t4614+t4617+t4641+t4645+t5191+t6062+t6066+t6092+t6096+t6568+t6571+t6591+t6593+t7119+t7124+t7128+t7130;
t7991 = t2963+t2964+t3664+t3665+t3744+t3794+t3872+t3922+t4201+t4243+t4400+t4406+t4428+t4429+t4599+t4602+t4667+t4669+t5191+t6064+t6067+t6091+t6095+t6570+t6572+t6586+t6592+t7121+t7125+t7127+t7129;
t7992 = t2963+t2964+t3664+t3665+t3744+t3794+t3872+t3922+t4201+t4243+t4400+t4406+t4428+t4429+t4614+t4617+t4667+t4669+t5191+t6062+t6066+t6091+t6095+t6568+t6571+t6586+t6592+t7119+t7124+t7127+t7129;
t5790 = t4588+t5364;
t6158 = t3901.*t5758.*(t1513+t1879+t2598+t2820+t2834+t3117+t3118).*(-7.26735e-3);
t6159 = t3901.*t5758.*(t1513+t1879+t2598+t2820+t2834+t3117+t3118).*7.26735e-3;
t6186 = -t3877.*t5784.*(t1488+t1874+t2519+t2740+t2747+t3096+t3097);
t6188 = t3877.*t5784.*(t1488+t1874+t2519+t2740+t2747+t3096+t3097);
t6550 = -t6548;
t6558 = -t6554;
t6615 = t5784.*t5800;
t6616 = t5784.*t5801;
t6694 = t5758.*t5895;
t6699 = t5758.*t5898;
t6851 = t3901.*t3918.*t6564.*7.26735e-3;
t6858 = t3901.*t3984.*t6564.*7.26735e-3;
t6874 = t3901.*t4149.*t6564.*7.26735e-3;
t6894 = t3877.*t3892.*t6606;
t6907 = t3877.*t4108.*t6606;
t6911 = t3901.*t3918.*t6631.*7.26735e-3;
t6921 = t3901.*t3984.*t6631.*7.26735e-3;
t6931 = t3901.*t4149.*t6631.*7.26735e-3;
t6940 = t3877.*t4298.*t6606;
t6963 = t3877.*t3941.*t6696;
t6976 = t3877.*t4108.*t6696;
t6985 = t3877.*t4298.*t6696;
t6994 = t5314.*t6564;
t7004 = t5220.*t6606;
t7006 = t5321.*t6564;
t7017 = t5262.*t6606;
t7033 = t5368.*t6564;
t7047 = t5324.*t6606;
t7052 = t5314.*t6631;
t7063 = t5321.*t6631;
t7066 = t5220.*t6696;
t7069 = t5262.*t6696;
et367 = -t2306-t2317+t3144+t3147+t35.*t941.*t948.*(t850-t874).*3.775747223193135e-1;
et368 = t36.*t941.*t948.*(t850-t874).*2.244797987218524e-1;
t7086 = t6606.*(et367+et368).*(t1488+t1874+t2519+t2740+t2747+t3096+t3097);
t7090 = t5368.*t6631;
t7095 = t5324.*t6696;
et369 = -t2306-t2317+t3144+t3147+t35.*t941.*t948.*(t850-t874).*3.775747223193135e-1;
et370 = t36.*t941.*t948.*(t850-t874).*2.244797987218524e-1;
t7100 = t6696.*(et369+et370).*(t1488+t1874+t2519+t2740+t2747+t3096+t3097);
t7106 = t5738.*t6564;
t7110 = t5713.*t6606;
t7112 = t5784.*t6564;
t7115 = t5758.*t6606;
t7116 = t5738.*t6631;
t7126 = -t6564.*(t4612-t5401);
t7140 = t5796.*t6606;
t7143 = t5784.*t6631;
t7145 = t5798.*t6606;
t7149 = t5758.*t6696;
t7153 = t5843.*t6564;
t7155 = -t6631.*(t4612-t5401);
t7156 = t6631.*(t4612-t5401);
t7160 = t5884.*t6564;
t7164 = t5796.*t6696;
t7167 = t5798.*t6696;
t7169 = t5843.*t6631;
t7172 = t5884.*t6631;
t7176 = t5985.*t6606;
t7186 = t5976.*t6696;
t7235 = -t7234;
tau_c = ft_16({t1005,t1022,t1089,t1104,t1105,t1108,t1115,t1121,t1158,t1159,t1196,t1205,t1210,t1212,t1217,t1218,t123,t1237,t1238,t1288,t1289,t1302,t1303,t1319,t1320,t1336,t1348,t1350,t1351,t1360,t1369,t1378,t1396,t14,t140,t1425,t1435,t1456,t1477,t1488,t15,t1513,t1539,t1554,t1577,t1578,t1586,t1587,t16,t1600,t1606,t1608,t1609,t1629,t1637,t1640,t1641,t1659,t1661,t1666,t1667,t1683,t1686,t1690,t1692,t17,t1700,t1701,t1705,t1712,t1758,t1759,t1775,t1776,t18,t1861,t1874,t1879,t188,t1881,t189,t1896,t19,t1901,t1941,t1959,t1973,t1993,t1994,t2,t20,t201,t202,t2023,t2053,t2060,t2089,t2090,t2098,t2099,t21,t2117,t2120,t2122,t2123,t2139,t2140,t2147,t2152,t2154,t2155,t2159,t2165,t2174,t2183,t2187,t2193,t2194,t2195,t2199,t22,t2203,t2215,t2219,t2222,t2223,t2239,t2240,t2256,t2257,t2292,t2295,t2297,t23,t2303,t2306,t2307,t2317,t2337,t2338,t2339,t2355,t236,t2361,t2362,t2363,t2367,t237,t2371,t238,t2388,t24,t241,t2414,t2419,t244,t25,t2502,t2519,t2527,t2555,t2556,t2572,t2583,t2598,t26,t2605,t2606,t2612,t2613,t2618,t2619,t262,t264,t2651,t2652,t2671,t2674,t2676,t2683,t2684,t2689,t2694,t2695,t2698,t27,t2701,t2707,t2716,t2719,t2740,t2747,t2754,t28,t2801,t2804,t2813,t2814,t2820,t2831,t2834,t2835,t2838,t2850,t2851,t2953,t2990,t2991,t2994,t3,t30,t3009,t3022,t3027,t3030,t3036,t3043,t3047,t3054,t3056,t3057,t3064,t3072,t3080,t3096,t3097,t31,t3109,t3117,t3118,t3121,t3122,t3128,t313,t3130,t3131,t3132,t314,t3144,t3147,t3156,t3157,t3170,t3189,t3190,t32,t3200,t3206,t3209,t321,t3210,t3214,t3228,t3229,t3230,t3231,t3232,t3235,t3269,t3270,t3272,t3283,t3290,t3292,t3296,t33,t3305,t3306,t3308,t3313,t3318,t3319,t332,t3327,t3334,t3341,t3349,t335,t3359,t3360,t3376,t3385,t3386,t3395,t3399,t34,t3405,t3409,t3410,t3412,t3417,t3420,t3421,t3423,t3424,t3435,t3437,t3455,t3465,t3468,t3470,t3480,t3481,t3483,t3484,t3493,t3498,t35,t350,t3505,t3524,t3528,t3535,t3544,t3547,t3560,t3563,t3570,t3571,t3576,t3582,t3588,t3590,t3593,t36,t3617,t3620,t3621,t3622,t3628,t3634,t3637,t3638,t3649,t366,t3680,t3681,t3684,t3685,t3689,t3693,t3694,t3708,t3714,t3716,t3723,t3732,t3779,t3782,t3783,t3784,t3790,t3791,t38,t3811,t3817,t3827,t3833,t3834,t3847,t3849,t3850,t3861,t3862,t3863,t3865,t3866,t3869,t3870,t3871,t3877,t3880,t3882,t3891,t3892,t3898,t39,t3901,t3904,t3910,t3918,t3928,t3934,t3940,t3941,t3942,t3946,t3951,t3957,t3959,t3967,t3972,t3974,t3984,t3985,t3992,t3996,t4,t4007,t4011,t4013,t4015,t4016,t4027,t4062,t4071,t4072,t4076,t4077,t4080,t410,t4108,t4109,t4119,t4120,t4134,t4149,t4154,t4160,t4163,t4173,t4175,t4196,t42,t4200,t4219,t4220,t4221,t4230,t4231,t4238,t4239,t4242,t4244,t4255,t4256,t4257,t4259,t4264,t4266,t4277,t4279,t4280,t4281,t4285,t4287,t4291,t4292,t4295,t4298,t43,t4304,t4311,t4323,t4324,t4362,t4363,t4409,t4413,t4421,t4432,t4437,t4438,t4444,t4447,t4458,t4491,t4496,t4499,t4500,t4504,t4507,t4510,t4513,t4514,t4519,t4520,t4531,t4540,t4541,t4543,t4552,t4554,t4555,t4556,t4560,t4571,t4572,t4576,t4579,t4582,t4589,t4595,t46,t4610,t4615,t4620,t4640,t4642,t4644,t4647,t4650,t4652,t4655,t4658,t4661,t4663,t4664,t4679,t4680,t4682,t4683,t4686,t4688,t4699,t47,t4702,t4703,t4704,t4705,t4737,t4741,t4742,t4744,t4751,t4752,t4758,t4767,t4772,t4777,t4780,t4785,t4786,t4789,t4792,t4795,t4814,t4816,t4817,t4819,t4822,t4823,t4824,t4826,t4829,t4833,t4842,t4848,t4849,t4850,t4851,t4856,t4857,t4860,t4865,t4868,t4869,t4870,t4871,t4874,t4898,t4911,t4931,t4963,t4965,t4974,t4975,t4976,t4977,t4983,t4985,t4986,t4987,t4992,t5,t50,t5005,t5007,t5031,t5033,t5034,t5035,t5036,t5038,t5039,t5040,t5041,t5042,t5047,t5048,t5049,t5051,t5052,t5055,t5056,t5057,t5058,t5069,t5092,t5103,t5104,t5105,t5111,t5114,t5117,t5119,t5133,t5134,t5135,t5136,t5139,t5140,t5148,t5150,t5151,t5152,t5155,t5164,t5184,t5186,t5189,t5192,t5195,t5196,t5198,t5203,t5204,t5207,t5209,t5210,t5220,t5223,t5224,t5225,t5227,t5230,t5231,t5235,t5240,t5241,t5243,t5245,t5246,t5247,t5248,t5250,t5252,t5254,t5262,t5273,t5276,t5277,t5278,t5281,t5282,t5285,t5286,t5288,t5289,t5291,t5301,t5304,t5306,t5307,t5308,t5314,t5316,t5317,t5320,t5321,t5322,t5328,t5330,t5331,t5332,t5335,t5337,t5338,t5339,t5340,t5342,t5344,t5345,t5346,t5347,t5348,t5349,t5350,t5356,t5357,t5358,t5361,t5362,t5365,t5367,t5372,t5377,t5379,t5380,t5381,t5383,t5384,t5388,t5389,t5396,t5397,t5399,t5400,t5402,t5403,t5405,t5407,t5411,t5412,t5413,t5414,t5426,t5427,t5428,t5429,t5432,t5433,t5434,t5436,t5437,t5438,t5440,t5441,t5443,t5444,t5453,t5460,t5468,t5480,t5481,t5482,t5483,t5484,t5486,t5487,t5488,t5489,t5490,t5491,t5492,t5493,t5494,t5496,t5498,t5499,t5500,t5503,t5504,t5505,t5506,t5507,t5509,t5512,t5513,t5514,t5515,t5516,t5517,t5518,t5520,t5521,t5522,t5523,t5524,t5525,t5526,t5527,t5528,t5531,t5532,t5534,t5537,t5538,t5539,t5543,t5544,t5550,t5552,t5556,t5558,t5559,t5561,t5563,t5566,t5575,t5578,t5580,t5581,t5582,t5583,t5585,t5586,t5588,t5589,t5592,t5593,t5594,t5595,t5596,t56,t5601,t5612,t5615,t5617,t5619,t5620,t5621,t5622,t5624,t5626,t5627,t5628,t5629,t5631,t5635,t5636,t5639,t5654,t5655,t5658,t5659,t5660,t5662,t5663,t5664,t5665,t5666,t5670,t5671,t5674,t5675,t5678,t5679,t5681,t5682,t5685,t5687,t5689,t5693,t5694,t5695,t5700,t5701,t5702,t5703,t5704,t5705,t5706,t5707,t5708,t5709,t5710,t5711,t5712,t5713,t5714,t5715,t5716,t5717,t5718,t5720,t5721,t5722,t5723,t5725,t5726,t5727,t5728,t5730,t5731,t5733,t5735,t5738,t5739,t5740,t5743,t5745,t5749,t5751,t5756,t5760,t5762,t5763,t5764,t5765,t5770,t5771,t5772,t5773,t5775,t5779,t5782,t5785,t5786,t5787,t5790,t5791,t5792,t5793,t5796,t5797,t5798,t5799,t5800,t5801,t5808,t5809,t5810,t5811,t5813,t5815,t5816,t5818,t5819,t5820,t5821,t5822,t5823,t5824,t5825,t5831,t5832,t5833,t5835,t5836,t5837,t5838,t5842,t5845,t5846,t5847,t5850,t5851,t5852,t5853,t5855,t5857,t5858,t5859,t5860,t5861,t5862,t5864,t5865,t5866,t5868,t5870,t5871,t5873,t5875,t5876,t5877,t5879,t5883,t5884,t5885,t5887,t5888,t5889,t5890,t5891,t5892,t5893,t5894,t5895,t5896,t5898,t5900,t5904,t5906,t5907,t5908,t5910,t5912,t5913,t5914,t5917,t5918,t5919,t5920,t5922,t5923,t5924,t5925,t5930,t5932,t5943,t5944,t5945,t5946,t5947,t5948,t5949,t5951,t5952,t5953,t5954,t5958,t5959,t5960,t5963,t5964,t5966,t5968,t5969,t5970,t5972,t5973,t5975,t5976,t5983,t5985,t5994,t5997,t5998,t6,t60,t6001,t6002,t6004,t6005,t6007,t6009,t6010,t6018,t6019,t6020,t6023,t6028,t6030,t6034,t6039,t6047,t6048,t6051,t6053,t6054,t6058,t6075,t6076,t6079,t6080,t6084,t6088,t6089,t6090,t6093,t6098,t6099,t6101,t6102,t6103,t6104,t6105,t6106,t6107,t6108,t6109,t6110,t6111,t6112,t6113,t6114,t6116,t6117,t6118,t6119,t6122,t6123,t6124,t6129,t6130,t6132,t6134,t6139,t6141,t6142,t6143,t6144,t6147,t6150,t6154,t6155,t6156,t6157,t6159,t6160,t6161,t6166,t6168,t6169,t6172,t6178,t6179,t6183,t6184,t6185,t6188,t6190,t6194,t6199,t6200,t6202,t6206,t6207,t6209,t6210,t6214,t6218,t6219,t6221,t6222,t6223,t6226,t6227,t6229,t6230,t6232,t6233,t6234,t6235,t6236,t6237,t6238,t6239,t6240,t6241,t6242,t6245,t6247,t6248,t6249,t6251,t6252,t6253,t6256,t6282,t6286,t6289,t6291,t6293,t6294,t6295,t6296,t6297,t6298,t6299,t6300,t6301,t6303,t6304,t6317,t6318,t6320,t6321,t6322,t6323,t6328,t6333,t6335,t6337,t6338,t6339,t6341,t6342,t6345,t6348,t6351,t6353,t6356,t6359,t6360,t6361,t6362,t6365,t6366,t6367,t6370,t6372,t6374,t6375,t6377,t6378,t6379,t6380,t6387,t6388,t6389,t6391,t6392,t6399,t6401,t6403,t6404,t6406,t6407,t6413,t6414,t6415,t642,t6422,t6423,t6424,t6425,t6427,t6428,t643,t6430,t6432,t6436,t6437,t6438,t6439,t6441,t6442,t6444,t6445,t6450,t6451,t6452,t6453,t6459,t6471,t6472,t6474,t6475,t6476,t6477,t6478,t6479,t6482,t6483,t6484,t6485,t6486,t6489,t649,t6490,t6491,t6492,t6493,t6495,t6496,t6497,t6500,t6502,t6505,t6507,t6508,t6510,t6511,t6512,t6515,t6521,t6522,t6523,t6528,t6529,t6534,t6536,t6538,t6540,t6541,t6542,t6543,t6544,t6546,t6547,t6548,t6550,t6551,t6552,t6553,t6554,t6555,t6556,t6557,t6558,t6559,t6560,t6561,t6562,t6563,t6564,t6565,t6566,t6577,t6584,t6585,t6587,t6588,t6595,t6596,t6597,t6598,t6599,t6600,t6601,t6603,t6604,t6605,t6606,t6608,t6609,t6610,t6611,t6612,t6613,t6614,t6615,t6616,t6617,t6620,t6622,t6623,t6624,t6625,t6627,t6628,t6629,t6631,t6638,t6641,t6645,t6647,t6648,t6649,t6653,t6655,t6656,t6657,t6658,t6659,t6660,t6663,t6664,t6667,t6668,t6669,t667,t6671,t6672,t6673,t6674,t6675,t6676,t6677,t6678,t6679,t6680,t6681,t6682,t6683,t6684,t6685,t6686,t6687,t6688,t6689,t6690,t6691,t6692,t6694,t6695,t6696,t6697,t6698,t6699,t670,t6700,t6701,t6703,t6707,t6710,t6711,t6713,t6714,t6716,t6717,t6720,t6722,t6725,t6727,t6728,t6729,t6730,t6731,t6733,t6734,t6735,t6736,t6737,t6738,t6739,t674,t6743,t6744,t6746,t6747,t6748,t6750,t6752,t6753,t6754,t6761,t6762,t6763,t6764,t6765,t6767,t6770,t6772,t6773,t6774,t6775,t6777,t6779,t6780,t6781,t6783,t6788,t6792,t6795,t6799,t6800,t6801,t6802,t6803,t6807,t6809,t6810,t6811,t6812,t6813,t6821,t6823,t6824,t6825,t6837,t6839,t684,t6841,t6842,t6843,t685,t6851,t6854,t6856,t6857,t6858,t686,t6860,t6861,t6863,t6864,t6865,t6866,t6868,t6869,t687,t6870,t6871,t6872,t6874,t6876,t6878,t6880,t6882,t6884,t6886,t6887,t6891,t6892,t6893,t6894,t6898,t6899,t6900,t6902,t6903,t6905,t6907,t6910,t6911,t6913,t6916,t6917,t6919,t6920,t6921,t6924,t6925,t6926,t6929,t6930,t6931,t6932,t6933,t6934,t6935,t6936,t6937,t6938,t6939,t6940,t6942,t6943,t6944,t6945,t6949,t6950,t6951,t6953,t6954,t6956,t6957,t6958,t6959,t6960,t6961,t6962,t6963,t6969,t6970,t6972,t6973,t6975,t6976,t6979,t6983,t6984,t6985,t6986,t6988,t6989,t6991,t6993,t6994,t7,t7000,t7001,t7003,t7004,t7006,t7010,t7017,t7019,t7022,t7023,t7024,t7030,t7033,t7039,t7040,t7041,t7047,t7050,t7052,t7053,t7054,t7055,t7056,t7057,t7058,t7060,t7063,t7066,t7068,t7069,t707,t7071,t7072,t7074,t7076,t7077,t7079,t708,t7086,t7087,t7089,t7090,t7091,t7093,t7094,t7095,t7099,t710,t7100,t7103,t7105,t7106,t7107,t7108,t7109,t7110,t7111,t7112,t7113,t7114,t7115,t7116,t7123,t7126,t7132,t7133,t7135,t7138,t7139,t7140,t7141,t7142,t7143,t7145,t7148,t7149,t7150,t7152,t7153,t7156,t7157,t7159,t7160,t7163,t7164,t7166,t7167,t7168,t7169,t7171,t7172,t7175,t7176,t7179,t7181,t7185,t7186,t7195,t7196,t7200,t7201,t7202,t7203,t7204,t7209,t721,t7211,t7212,t7219,t722,t7223,t7224,t7225,t7232,t7233,t7235,t724,t7240,t7242,t7245,t7246,t7250,t7252,t7253,t7254,t7255,t7257,t7259,t7266,t7268,t7277,t7278,t7282,t7284,t7285,t7286,t7287,t7288,t7290,t7292,t7293,t7295,t7296,t7297,t7298,t7299,t7300,t7301,t7302,t7303,t7304,t7305,t7306,t7307,t7308,t7309,t7311,t7313,t7316,t7317,t7325,t7326,t7331,t7333,t7334,t7336,t7337,t7339,t7340,t7342,t7343,t7345,t7346,t7347,t7349,t7351,t7353,t7354,t7359,t7360,t7361,t7362,t7363,t7371,t7372,t7375,t7381,t7382,t7384,t7386,t7388,t7394,t7404,t7405,t7407,t7411,t7412,t7416,t7417,t7418,t7419,t7429,t7430,t7431,t7432,t7433,t7440,t7443,t7444,t7445,t7446,t7447,t7453,t7459,t7461,t7478,t7479,t7482,t749,t7505,t7508,t7510,t7516,t7518,t7519,t7520,t7521,t7522,t7523,t7524,t7530,t7534,t7539,t7540,t7549,t7550,t7563,t7565,t7566,t7575,t7576,t7579,t7580,t7583,t7584,t7586,t7590,t7591,t7597,t7600,t7602,t7604,t7605,t7606,t7607,t7610,t7611,t7612,t7613,t7615,t762,t7621,t7622,t7623,t7624,t7631,t7632,t7633,t7635,t7637,t7638,t7652,t7655,t7658,t7659,t7664,t7665,t7666,t7676,t768,t7680,t7682,t7683,t7684,t7686,t7689,t7691,t7692,t7698,t7699,t7703,t7710,t7730,t7731,t7732,t7733,t7734,t7735,t7736,t7738,t7741,t7745,t7746,t7748,t7749,t7751,t7754,t7757,t7759,t7762,t7765,t7766,t7768,t777,t7770,t7771,t7772,t7774,t7775,t7778,t7780,t7781,t7782,t7784,t7787,t7790,t7791,t7792,t7794,t7795,t7803,t7804,t7805,t7806,t7811,t7812,t7813,t7814,t7815,t7816,t7819,t7820,t7821,t7823,t7824,t7826,t7828,t7830,t7841,t7843,t7844,t7853,t7854,t7856,t7868,t7876,t7879,t7882,t7886,t7891,t7892,t7893,t7895,t7897,t7899,t7900,t7902,t7909,t792,t7922,t7923,t7924,t7925,t7926,t7927,t7928,t7929,t793,t7930,t7931,t7933,t7934,t7952,t7953,t7954,t7967,t7968,t7969,t7971,t7973,t7975,t7976,t7989,t7990,t7991,t7992,t801,t802,t808,t813,t819,t821,t850,t855,t874,t878,t941,t948,t951});
end
function tau_c = ft_16(ct)
t1005 = ct{1};
t1022 = ct{2};
t1089 = ct{3};
t1104 = ct{4};
t1105 = ct{5};
t1108 = ct{6};
t1115 = ct{7};
t1121 = ct{8};
t1158 = ct{9};
t1159 = ct{10};
t1196 = ct{11};
t1205 = ct{12};
t1210 = ct{13};
t1212 = ct{14};
t1217 = ct{15};
t1218 = ct{16};
t123 = ct{17};
t1237 = ct{18};
t1238 = ct{19};
t1288 = ct{20};
t1289 = ct{21};
t1302 = ct{22};
t1303 = ct{23};
t1319 = ct{24};
t1320 = ct{25};
t1336 = ct{26};
t1348 = ct{27};
t1350 = ct{28};
t1351 = ct{29};
t1360 = ct{30};
t1369 = ct{31};
t1378 = ct{32};
t1396 = ct{33};
t14 = ct{34};
t140 = ct{35};
t1425 = ct{36};
t1435 = ct{37};
t1456 = ct{38};
t1477 = ct{39};
t1488 = ct{40};
t15 = ct{41};
t1513 = ct{42};
t1539 = ct{43};
t1554 = ct{44};
t1577 = ct{45};
t1578 = ct{46};
t1586 = ct{47};
t1587 = ct{48};
t16 = ct{49};
t1600 = ct{50};
t1606 = ct{51};
t1608 = ct{52};
t1609 = ct{53};
t1629 = ct{54};
t1637 = ct{55};
t1640 = ct{56};
t1641 = ct{57};
t1659 = ct{58};
t1661 = ct{59};
t1666 = ct{60};
t1667 = ct{61};
t1683 = ct{62};
t1686 = ct{63};
t1690 = ct{64};
t1692 = ct{65};
t17 = ct{66};
t1700 = ct{67};
t1701 = ct{68};
t1705 = ct{69};
t1712 = ct{70};
t1758 = ct{71};
t1759 = ct{72};
t1775 = ct{73};
t1776 = ct{74};
t18 = ct{75};
t1861 = ct{76};
t1874 = ct{77};
t1879 = ct{78};
t188 = ct{79};
t1881 = ct{80};
t189 = ct{81};
t1896 = ct{82};
t19 = ct{83};
t1901 = ct{84};
t1941 = ct{85};
t1959 = ct{86};
t1973 = ct{87};
t1993 = ct{88};
t1994 = ct{89};
t2 = ct{90};
t20 = ct{91};
t201 = ct{92};
t202 = ct{93};
t2023 = ct{94};
t2053 = ct{95};
t2060 = ct{96};
t2089 = ct{97};
t2090 = ct{98};
t2098 = ct{99};
t2099 = ct{100};
t21 = ct{101};
t2117 = ct{102};
t2120 = ct{103};
t2122 = ct{104};
t2123 = ct{105};
t2139 = ct{106};
t2140 = ct{107};
t2147 = ct{108};
t2152 = ct{109};
t2154 = ct{110};
t2155 = ct{111};
t2159 = ct{112};
t2165 = ct{113};
t2174 = ct{114};
t2183 = ct{115};
t2187 = ct{116};
t2193 = ct{117};
t2194 = ct{118};
t2195 = ct{119};
t2199 = ct{120};
t22 = ct{121};
t2203 = ct{122};
t2215 = ct{123};
t2219 = ct{124};
t2222 = ct{125};
t2223 = ct{126};
t2239 = ct{127};
t2240 = ct{128};
t2256 = ct{129};
t2257 = ct{130};
t2292 = ct{131};
t2295 = ct{132};
t2297 = ct{133};
t23 = ct{134};
t2303 = ct{135};
t2306 = ct{136};
t2307 = ct{137};
t2317 = ct{138};
t2337 = ct{139};
t2338 = ct{140};
t2339 = ct{141};
t2355 = ct{142};
t236 = ct{143};
t2361 = ct{144};
t2362 = ct{145};
t2363 = ct{146};
t2367 = ct{147};
t237 = ct{148};
t2371 = ct{149};
t238 = ct{150};
t2388 = ct{151};
t24 = ct{152};
t241 = ct{153};
t2414 = ct{154};
t2419 = ct{155};
t244 = ct{156};
t25 = ct{157};
t2502 = ct{158};
t2519 = ct{159};
t2527 = ct{160};
t2555 = ct{161};
t2556 = ct{162};
t2572 = ct{163};
t2583 = ct{164};
t2598 = ct{165};
t26 = ct{166};
t2605 = ct{167};
t2606 = ct{168};
t2612 = ct{169};
t2613 = ct{170};
t2618 = ct{171};
t2619 = ct{172};
t262 = ct{173};
t264 = ct{174};
t2651 = ct{175};
t2652 = ct{176};
t2671 = ct{177};
t2674 = ct{178};
t2676 = ct{179};
t2683 = ct{180};
t2684 = ct{181};
t2689 = ct{182};
t2694 = ct{183};
t2695 = ct{184};
t2698 = ct{185};
t27 = ct{186};
t2701 = ct{187};
t2707 = ct{188};
t2716 = ct{189};
t2719 = ct{190};
t2740 = ct{191};
t2747 = ct{192};
t2754 = ct{193};
t28 = ct{194};
t2801 = ct{195};
t2804 = ct{196};
t2813 = ct{197};
t2814 = ct{198};
t2820 = ct{199};
t2831 = ct{200};
t2834 = ct{201};
t2835 = ct{202};
t2838 = ct{203};
t2850 = ct{204};
t2851 = ct{205};
t2953 = ct{206};
t2990 = ct{207};
t2991 = ct{208};
t2994 = ct{209};
t3 = ct{210};
t30 = ct{211};
t3009 = ct{212};
t3022 = ct{213};
t3027 = ct{214};
t3030 = ct{215};
t3036 = ct{216};
t3043 = ct{217};
t3047 = ct{218};
t3054 = ct{219};
t3056 = ct{220};
t3057 = ct{221};
t3064 = ct{222};
t3072 = ct{223};
t3080 = ct{224};
t3096 = ct{225};
t3097 = ct{226};
t31 = ct{227};
t3109 = ct{228};
t3117 = ct{229};
t3118 = ct{230};
t3121 = ct{231};
t3122 = ct{232};
t3128 = ct{233};
t313 = ct{234};
t3130 = ct{235};
t3131 = ct{236};
t3132 = ct{237};
t314 = ct{238};
t3144 = ct{239};
t3147 = ct{240};
t3156 = ct{241};
t3157 = ct{242};
t3170 = ct{243};
t3189 = ct{244};
t3190 = ct{245};
t32 = ct{246};
t3200 = ct{247};
t3206 = ct{248};
t3209 = ct{249};
t321 = ct{250};
t3210 = ct{251};
t3214 = ct{252};
t3228 = ct{253};
t3229 = ct{254};
t3230 = ct{255};
t3231 = ct{256};
t3232 = ct{257};
t3235 = ct{258};
t3269 = ct{259};
t3270 = ct{260};
t3272 = ct{261};
t3283 = ct{262};
t3290 = ct{263};
t3292 = ct{264};
t3296 = ct{265};
t33 = ct{266};
t3305 = ct{267};
t3306 = ct{268};
t3308 = ct{269};
t3313 = ct{270};
t3318 = ct{271};
t3319 = ct{272};
t332 = ct{273};
t3327 = ct{274};
t3334 = ct{275};
t3341 = ct{276};
t3349 = ct{277};
t335 = ct{278};
t3359 = ct{279};
t3360 = ct{280};
t3376 = ct{281};
t3385 = ct{282};
t3386 = ct{283};
t3395 = ct{284};
t3399 = ct{285};
t34 = ct{286};
t3405 = ct{287};
t3409 = ct{288};
t3410 = ct{289};
t3412 = ct{290};
t3417 = ct{291};
t3420 = ct{292};
t3421 = ct{293};
t3423 = ct{294};
t3424 = ct{295};
t3435 = ct{296};
t3437 = ct{297};
t3455 = ct{298};
t3465 = ct{299};
t3468 = ct{300};
t3470 = ct{301};
t3480 = ct{302};
t3481 = ct{303};
t3483 = ct{304};
t3484 = ct{305};
t3493 = ct{306};
t3498 = ct{307};
t35 = ct{308};
t350 = ct{309};
t3505 = ct{310};
t3524 = ct{311};
t3528 = ct{312};
t3535 = ct{313};
t3544 = ct{314};
t3547 = ct{315};
t3560 = ct{316};
t3563 = ct{317};
t3570 = ct{318};
t3571 = ct{319};
t3576 = ct{320};
t3582 = ct{321};
t3588 = ct{322};
t3590 = ct{323};
t3593 = ct{324};
t36 = ct{325};
t3617 = ct{326};
t3620 = ct{327};
t3621 = ct{328};
t3622 = ct{329};
t3628 = ct{330};
t3634 = ct{331};
t3637 = ct{332};
t3638 = ct{333};
t3649 = ct{334};
t366 = ct{335};
t3680 = ct{336};
t3681 = ct{337};
t3684 = ct{338};
t3685 = ct{339};
t3689 = ct{340};
t3693 = ct{341};
t3694 = ct{342};
t3708 = ct{343};
t3714 = ct{344};
t3716 = ct{345};
t3723 = ct{346};
t3732 = ct{347};
t3779 = ct{348};
t3782 = ct{349};
t3783 = ct{350};
t3784 = ct{351};
t3790 = ct{352};
t3791 = ct{353};
t38 = ct{354};
t3811 = ct{355};
t3817 = ct{356};
t3827 = ct{357};
t3833 = ct{358};
t3834 = ct{359};
t3847 = ct{360};
t3849 = ct{361};
t3850 = ct{362};
t3861 = ct{363};
t3862 = ct{364};
t3863 = ct{365};
t3865 = ct{366};
t3866 = ct{367};
t3869 = ct{368};
t3870 = ct{369};
t3871 = ct{370};
t3877 = ct{371};
t3880 = ct{372};
t3882 = ct{373};
t3891 = ct{374};
t3892 = ct{375};
t3898 = ct{376};
t39 = ct{377};
t3901 = ct{378};
t3904 = ct{379};
t3910 = ct{380};
t3918 = ct{381};
t3928 = ct{382};
t3934 = ct{383};
t3940 = ct{384};
t3941 = ct{385};
t3942 = ct{386};
t3946 = ct{387};
t3951 = ct{388};
t3957 = ct{389};
t3959 = ct{390};
t3967 = ct{391};
t3972 = ct{392};
t3974 = ct{393};
t3984 = ct{394};
t3985 = ct{395};
t3992 = ct{396};
t3996 = ct{397};
t4 = ct{398};
t4007 = ct{399};
t4011 = ct{400};
t4013 = ct{401};
t4015 = ct{402};
t4016 = ct{403};
t4027 = ct{404};
t4062 = ct{405};
t4071 = ct{406};
t4072 = ct{407};
t4076 = ct{408};
t4077 = ct{409};
t4080 = ct{410};
t410 = ct{411};
t4108 = ct{412};
t4109 = ct{413};
t4119 = ct{414};
t4120 = ct{415};
t4134 = ct{416};
t4149 = ct{417};
t4154 = ct{418};
t4160 = ct{419};
t4163 = ct{420};
t4173 = ct{421};
t4175 = ct{422};
t4196 = ct{423};
t42 = ct{424};
t4200 = ct{425};
t4219 = ct{426};
t4220 = ct{427};
t4221 = ct{428};
t4230 = ct{429};
t4231 = ct{430};
t4238 = ct{431};
t4239 = ct{432};
t4242 = ct{433};
t4244 = ct{434};
t4255 = ct{435};
t4256 = ct{436};
t4257 = ct{437};
t4259 = ct{438};
t4264 = ct{439};
t4266 = ct{440};
t4277 = ct{441};
t4279 = ct{442};
t4280 = ct{443};
t4281 = ct{444};
t4285 = ct{445};
t4287 = ct{446};
t4291 = ct{447};
t4292 = ct{448};
t4295 = ct{449};
t4298 = ct{450};
t43 = ct{451};
t4304 = ct{452};
t4311 = ct{453};
t4323 = ct{454};
t4324 = ct{455};
t4362 = ct{456};
t4363 = ct{457};
t4409 = ct{458};
t4413 = ct{459};
t4421 = ct{460};
t4432 = ct{461};
t4437 = ct{462};
t4438 = ct{463};
t4444 = ct{464};
t4447 = ct{465};
t4458 = ct{466};
t4491 = ct{467};
t4496 = ct{468};
t4499 = ct{469};
t4500 = ct{470};
t4504 = ct{471};
t4507 = ct{472};
t4510 = ct{473};
t4513 = ct{474};
t4514 = ct{475};
t4519 = ct{476};
t4520 = ct{477};
t4531 = ct{478};
t4540 = ct{479};
t4541 = ct{480};
t4543 = ct{481};
t4552 = ct{482};
t4554 = ct{483};
t4555 = ct{484};
t4556 = ct{485};
t4560 = ct{486};
t4571 = ct{487};
t4572 = ct{488};
t4576 = ct{489};
t4579 = ct{490};
t4582 = ct{491};
t4589 = ct{492};
t4595 = ct{493};
t46 = ct{494};
t4610 = ct{495};
t4615 = ct{496};
t4620 = ct{497};
t4640 = ct{498};
t4642 = ct{499};
t4644 = ct{500};
t4647 = ct{501};
t4650 = ct{502};
t4652 = ct{503};
t4655 = ct{504};
t4658 = ct{505};
t4661 = ct{506};
t4663 = ct{507};
t4664 = ct{508};
t4679 = ct{509};
t4680 = ct{510};
t4682 = ct{511};
t4683 = ct{512};
t4686 = ct{513};
t4688 = ct{514};
t4699 = ct{515};
t47 = ct{516};
t4702 = ct{517};
t4703 = ct{518};
t4704 = ct{519};
t4705 = ct{520};
t4737 = ct{521};
t4741 = ct{522};
t4742 = ct{523};
t4744 = ct{524};
t4751 = ct{525};
t4752 = ct{526};
t4758 = ct{527};
t4767 = ct{528};
t4772 = ct{529};
t4777 = ct{530};
t4780 = ct{531};
t4785 = ct{532};
t4786 = ct{533};
t4789 = ct{534};
t4792 = ct{535};
t4795 = ct{536};
t4814 = ct{537};
t4816 = ct{538};
t4817 = ct{539};
t4819 = ct{540};
t4822 = ct{541};
t4823 = ct{542};
t4824 = ct{543};
t4826 = ct{544};
t4829 = ct{545};
t4833 = ct{546};
t4842 = ct{547};
t4848 = ct{548};
t4849 = ct{549};
t4850 = ct{550};
t4851 = ct{551};
t4856 = ct{552};
t4857 = ct{553};
t4860 = ct{554};
t4865 = ct{555};
t4868 = ct{556};
t4869 = ct{557};
t4870 = ct{558};
t4871 = ct{559};
t4874 = ct{560};
t4898 = ct{561};
t4911 = ct{562};
t4931 = ct{563};
t4963 = ct{564};
t4965 = ct{565};
t4974 = ct{566};
t4975 = ct{567};
t4976 = ct{568};
t4977 = ct{569};
t4983 = ct{570};
t4985 = ct{571};
t4986 = ct{572};
t4987 = ct{573};
t4992 = ct{574};
t5 = ct{575};
t50 = ct{576};
t5005 = ct{577};
t5007 = ct{578};
t5031 = ct{579};
t5033 = ct{580};
t5034 = ct{581};
t5035 = ct{582};
t5036 = ct{583};
t5038 = ct{584};
t5039 = ct{585};
t5040 = ct{586};
t5041 = ct{587};
t5042 = ct{588};
t5047 = ct{589};
t5048 = ct{590};
t5049 = ct{591};
t5051 = ct{592};
t5052 = ct{593};
t5055 = ct{594};
t5056 = ct{595};
t5057 = ct{596};
t5058 = ct{597};
t5069 = ct{598};
t5092 = ct{599};
t5103 = ct{600};
t5104 = ct{601};
t5105 = ct{602};
t5111 = ct{603};
t5114 = ct{604};
t5117 = ct{605};
t5119 = ct{606};
t5133 = ct{607};
t5134 = ct{608};
t5135 = ct{609};
t5136 = ct{610};
t5139 = ct{611};
t5140 = ct{612};
t5148 = ct{613};
t5150 = ct{614};
t5151 = ct{615};
t5152 = ct{616};
t5155 = ct{617};
t5164 = ct{618};
t5184 = ct{619};
t5186 = ct{620};
t5189 = ct{621};
t5192 = ct{622};
t5195 = ct{623};
t5196 = ct{624};
t5198 = ct{625};
t5203 = ct{626};
t5204 = ct{627};
t5207 = ct{628};
t5209 = ct{629};
t5210 = ct{630};
t5220 = ct{631};
t5223 = ct{632};
t5224 = ct{633};
t5225 = ct{634};
t5227 = ct{635};
t5230 = ct{636};
t5231 = ct{637};
t5235 = ct{638};
t5240 = ct{639};
t5241 = ct{640};
t5243 = ct{641};
t5245 = ct{642};
t5246 = ct{643};
t5247 = ct{644};
t5248 = ct{645};
t5250 = ct{646};
t5252 = ct{647};
t5254 = ct{648};
t5262 = ct{649};
t5273 = ct{650};
t5276 = ct{651};
t5277 = ct{652};
t5278 = ct{653};
t5281 = ct{654};
t5282 = ct{655};
t5285 = ct{656};
t5286 = ct{657};
t5288 = ct{658};
t5289 = ct{659};
t5291 = ct{660};
t5301 = ct{661};
t5304 = ct{662};
t5306 = ct{663};
t5307 = ct{664};
t5308 = ct{665};
t5314 = ct{666};
t5316 = ct{667};
t5317 = ct{668};
t5320 = ct{669};
t5321 = ct{670};
t5322 = ct{671};
t5328 = ct{672};
t5330 = ct{673};
t5331 = ct{674};
t5332 = ct{675};
t5335 = ct{676};
t5337 = ct{677};
t5338 = ct{678};
t5339 = ct{679};
t5340 = ct{680};
t5342 = ct{681};
t5344 = ct{682};
t5345 = ct{683};
t5346 = ct{684};
t5347 = ct{685};
t5348 = ct{686};
t5349 = ct{687};
t5350 = ct{688};
t5356 = ct{689};
t5357 = ct{690};
t5358 = ct{691};
t5361 = ct{692};
t5362 = ct{693};
t5365 = ct{694};
t5367 = ct{695};
t5372 = ct{696};
t5377 = ct{697};
t5379 = ct{698};
t5380 = ct{699};
t5381 = ct{700};
t5383 = ct{701};
t5384 = ct{702};
t5388 = ct{703};
t5389 = ct{704};
t5396 = ct{705};
t5397 = ct{706};
t5399 = ct{707};
t5400 = ct{708};
t5402 = ct{709};
t5403 = ct{710};
t5405 = ct{711};
t5407 = ct{712};
t5411 = ct{713};
t5412 = ct{714};
t5413 = ct{715};
t5414 = ct{716};
t5426 = ct{717};
t5427 = ct{718};
t5428 = ct{719};
t5429 = ct{720};
t5432 = ct{721};
t5433 = ct{722};
t5434 = ct{723};
t5436 = ct{724};
t5437 = ct{725};
t5438 = ct{726};
t5440 = ct{727};
t5441 = ct{728};
t5443 = ct{729};
t5444 = ct{730};
t5453 = ct{731};
t5460 = ct{732};
t5468 = ct{733};
t5480 = ct{734};
t5481 = ct{735};
t5482 = ct{736};
t5483 = ct{737};
t5484 = ct{738};
t5486 = ct{739};
t5487 = ct{740};
t5488 = ct{741};
t5489 = ct{742};
t5490 = ct{743};
t5491 = ct{744};
t5492 = ct{745};
t5493 = ct{746};
t5494 = ct{747};
t5496 = ct{748};
t5498 = ct{749};
t5499 = ct{750};
t5500 = ct{751};
t5503 = ct{752};
t5504 = ct{753};
t5505 = ct{754};
t5506 = ct{755};
t5507 = ct{756};
t5509 = ct{757};
t5512 = ct{758};
t5513 = ct{759};
t5514 = ct{760};
t5515 = ct{761};
t5516 = ct{762};
t5517 = ct{763};
t5518 = ct{764};
t5520 = ct{765};
t5521 = ct{766};
t5522 = ct{767};
t5523 = ct{768};
t5524 = ct{769};
t5525 = ct{770};
t5526 = ct{771};
t5527 = ct{772};
t5528 = ct{773};
t5531 = ct{774};
t5532 = ct{775};
t5534 = ct{776};
t5537 = ct{777};
t5538 = ct{778};
t5539 = ct{779};
t5543 = ct{780};
t5544 = ct{781};
t5550 = ct{782};
t5552 = ct{783};
t5556 = ct{784};
t5558 = ct{785};
t5559 = ct{786};
t5561 = ct{787};
t5563 = ct{788};
t5566 = ct{789};
t5575 = ct{790};
t5578 = ct{791};
t5580 = ct{792};
t5581 = ct{793};
t5582 = ct{794};
t5583 = ct{795};
t5585 = ct{796};
t5586 = ct{797};
t5588 = ct{798};
t5589 = ct{799};
t5592 = ct{800};
t5593 = ct{801};
t5594 = ct{802};
t5595 = ct{803};
t5596 = ct{804};
t56 = ct{805};
t5601 = ct{806};
t5612 = ct{807};
t5615 = ct{808};
t5617 = ct{809};
t5619 = ct{810};
t5620 = ct{811};
t5621 = ct{812};
t5622 = ct{813};
t5624 = ct{814};
t5626 = ct{815};
t5627 = ct{816};
t5628 = ct{817};
t5629 = ct{818};
t5631 = ct{819};
t5635 = ct{820};
t5636 = ct{821};
t5639 = ct{822};
t5654 = ct{823};
t5655 = ct{824};
t5658 = ct{825};
t5659 = ct{826};
t5660 = ct{827};
t5662 = ct{828};
t5663 = ct{829};
t5664 = ct{830};
t5665 = ct{831};
t5666 = ct{832};
t5670 = ct{833};
t5671 = ct{834};
t5674 = ct{835};
t5675 = ct{836};
t5678 = ct{837};
t5679 = ct{838};
t5681 = ct{839};
t5682 = ct{840};
t5685 = ct{841};
t5687 = ct{842};
t5689 = ct{843};
t5693 = ct{844};
t5694 = ct{845};
t5695 = ct{846};
t5700 = ct{847};
t5701 = ct{848};
t5702 = ct{849};
t5703 = ct{850};
t5704 = ct{851};
t5705 = ct{852};
t5706 = ct{853};
t5707 = ct{854};
t5708 = ct{855};
t5709 = ct{856};
t5710 = ct{857};
t5711 = ct{858};
t5712 = ct{859};
t5713 = ct{860};
t5714 = ct{861};
t5715 = ct{862};
t5716 = ct{863};
t5717 = ct{864};
t5718 = ct{865};
t5720 = ct{866};
t5721 = ct{867};
t5722 = ct{868};
t5723 = ct{869};
t5725 = ct{870};
t5726 = ct{871};
t5727 = ct{872};
t5728 = ct{873};
t5730 = ct{874};
t5731 = ct{875};
t5733 = ct{876};
t5735 = ct{877};
t5738 = ct{878};
t5739 = ct{879};
t5740 = ct{880};
t5743 = ct{881};
t5745 = ct{882};
t5749 = ct{883};
t5751 = ct{884};
t5756 = ct{885};
t5760 = ct{886};
t5762 = ct{887};
t5763 = ct{888};
t5764 = ct{889};
t5765 = ct{890};
t5770 = ct{891};
t5771 = ct{892};
t5772 = ct{893};
t5773 = ct{894};
t5775 = ct{895};
t5779 = ct{896};
t5782 = ct{897};
t5785 = ct{898};
t5786 = ct{899};
t5787 = ct{900};
t5790 = ct{901};
t5791 = ct{902};
t5792 = ct{903};
t5793 = ct{904};
t5796 = ct{905};
t5797 = ct{906};
t5798 = ct{907};
t5799 = ct{908};
t5800 = ct{909};
t5801 = ct{910};
t5808 = ct{911};
t5809 = ct{912};
t5810 = ct{913};
t5811 = ct{914};
t5813 = ct{915};
t5815 = ct{916};
t5816 = ct{917};
t5818 = ct{918};
t5819 = ct{919};
t5820 = ct{920};
t5821 = ct{921};
t5822 = ct{922};
t5823 = ct{923};
t5824 = ct{924};
t5825 = ct{925};
t5831 = ct{926};
t5832 = ct{927};
t5833 = ct{928};
t5835 = ct{929};
t5836 = ct{930};
t5837 = ct{931};
t5838 = ct{932};
t5842 = ct{933};
t5845 = ct{934};
t5846 = ct{935};
t5847 = ct{936};
t5850 = ct{937};
t5851 = ct{938};
t5852 = ct{939};
t5853 = ct{940};
t5855 = ct{941};
t5857 = ct{942};
t5858 = ct{943};
t5859 = ct{944};
t5860 = ct{945};
t5861 = ct{946};
t5862 = ct{947};
t5864 = ct{948};
t5865 = ct{949};
t5866 = ct{950};
t5868 = ct{951};
t5870 = ct{952};
t5871 = ct{953};
t5873 = ct{954};
t5875 = ct{955};
t5876 = ct{956};
t5877 = ct{957};
t5879 = ct{958};
t5883 = ct{959};
t5884 = ct{960};
t5885 = ct{961};
t5887 = ct{962};
t5888 = ct{963};
t5889 = ct{964};
t5890 = ct{965};
t5891 = ct{966};
t5892 = ct{967};
t5893 = ct{968};
t5894 = ct{969};
t5895 = ct{970};
t5896 = ct{971};
t5898 = ct{972};
t5900 = ct{973};
t5904 = ct{974};
t5906 = ct{975};
t5907 = ct{976};
t5908 = ct{977};
t5910 = ct{978};
t5912 = ct{979};
t5913 = ct{980};
t5914 = ct{981};
t5917 = ct{982};
t5918 = ct{983};
t5919 = ct{984};
t5920 = ct{985};
t5922 = ct{986};
t5923 = ct{987};
t5924 = ct{988};
t5925 = ct{989};
t5930 = ct{990};
t5932 = ct{991};
t5943 = ct{992};
t5944 = ct{993};
t5945 = ct{994};
t5946 = ct{995};
t5947 = ct{996};
t5948 = ct{997};
t5949 = ct{998};
t5951 = ct{999};
t5952 = ct{1000};
t5953 = ct{1001};
t5954 = ct{1002};
t5958 = ct{1003};
t5959 = ct{1004};
t5960 = ct{1005};
t5963 = ct{1006};
t5964 = ct{1007};
t5966 = ct{1008};
t5968 = ct{1009};
t5969 = ct{1010};
t5970 = ct{1011};
t5972 = ct{1012};
t5973 = ct{1013};
t5975 = ct{1014};
t5976 = ct{1015};
t5983 = ct{1016};
t5985 = ct{1017};
t5994 = ct{1018};
t5997 = ct{1019};
t5998 = ct{1020};
t6 = ct{1021};
t60 = ct{1022};
t6001 = ct{1023};
t6002 = ct{1024};
t6004 = ct{1025};
t6005 = ct{1026};
t6007 = ct{1027};
t6009 = ct{1028};
t6010 = ct{1029};
t6018 = ct{1030};
t6019 = ct{1031};
t6020 = ct{1032};
t6023 = ct{1033};
t6028 = ct{1034};
t6030 = ct{1035};
t6034 = ct{1036};
t6039 = ct{1037};
t6047 = ct{1038};
t6048 = ct{1039};
t6051 = ct{1040};
t6053 = ct{1041};
t6054 = ct{1042};
t6058 = ct{1043};
t6075 = ct{1044};
t6076 = ct{1045};
t6079 = ct{1046};
t6080 = ct{1047};
t6084 = ct{1048};
t6088 = ct{1049};
t6089 = ct{1050};
t6090 = ct{1051};
t6093 = ct{1052};
t6098 = ct{1053};
t6099 = ct{1054};
t6101 = ct{1055};
t6102 = ct{1056};
t6103 = ct{1057};
t6104 = ct{1058};
t6105 = ct{1059};
t6106 = ct{1060};
t6107 = ct{1061};
t6108 = ct{1062};
t6109 = ct{1063};
t6110 = ct{1064};
t6111 = ct{1065};
t6112 = ct{1066};
t6113 = ct{1067};
t6114 = ct{1068};
t6116 = ct{1069};
t6117 = ct{1070};
t6118 = ct{1071};
t6119 = ct{1072};
t6122 = ct{1073};
t6123 = ct{1074};
t6124 = ct{1075};
t6129 = ct{1076};
t6130 = ct{1077};
t6132 = ct{1078};
t6134 = ct{1079};
t6139 = ct{1080};
t6141 = ct{1081};
t6142 = ct{1082};
t6143 = ct{1083};
t6144 = ct{1084};
t6147 = ct{1085};
t6150 = ct{1086};
t6154 = ct{1087};
t6155 = ct{1088};
t6156 = ct{1089};
t6157 = ct{1090};
t6159 = ct{1091};
t6160 = ct{1092};
t6161 = ct{1093};
t6166 = ct{1094};
t6168 = ct{1095};
t6169 = ct{1096};
t6172 = ct{1097};
t6178 = ct{1098};
t6179 = ct{1099};
t6183 = ct{1100};
t6184 = ct{1101};
t6185 = ct{1102};
t6188 = ct{1103};
t6190 = ct{1104};
t6194 = ct{1105};
t6199 = ct{1106};
t6200 = ct{1107};
t6202 = ct{1108};
t6206 = ct{1109};
t6207 = ct{1110};
t6209 = ct{1111};
t6210 = ct{1112};
t6214 = ct{1113};
t6218 = ct{1114};
t6219 = ct{1115};
t6221 = ct{1116};
t6222 = ct{1117};
t6223 = ct{1118};
t6226 = ct{1119};
t6227 = ct{1120};
t6229 = ct{1121};
t6230 = ct{1122};
t6232 = ct{1123};
t6233 = ct{1124};
t6234 = ct{1125};
t6235 = ct{1126};
t6236 = ct{1127};
t6237 = ct{1128};
t6238 = ct{1129};
t6239 = ct{1130};
t6240 = ct{1131};
t6241 = ct{1132};
t6242 = ct{1133};
t6245 = ct{1134};
t6247 = ct{1135};
t6248 = ct{1136};
t6249 = ct{1137};
t6251 = ct{1138};
t6252 = ct{1139};
t6253 = ct{1140};
t6256 = ct{1141};
t6282 = ct{1142};
t6286 = ct{1143};
t6289 = ct{1144};
t6291 = ct{1145};
t6293 = ct{1146};
t6294 = ct{1147};
t6295 = ct{1148};
t6296 = ct{1149};
t6297 = ct{1150};
t6298 = ct{1151};
t6299 = ct{1152};
t6300 = ct{1153};
t6301 = ct{1154};
t6303 = ct{1155};
t6304 = ct{1156};
t6317 = ct{1157};
t6318 = ct{1158};
t6320 = ct{1159};
t6321 = ct{1160};
t6322 = ct{1161};
t6323 = ct{1162};
t6328 = ct{1163};
t6333 = ct{1164};
t6335 = ct{1165};
t6337 = ct{1166};
t6338 = ct{1167};
t6339 = ct{1168};
t6341 = ct{1169};
t6342 = ct{1170};
t6345 = ct{1171};
t6348 = ct{1172};
t6351 = ct{1173};
t6353 = ct{1174};
t6356 = ct{1175};
t6359 = ct{1176};
t6360 = ct{1177};
t6361 = ct{1178};
t6362 = ct{1179};
t6365 = ct{1180};
t6366 = ct{1181};
t6367 = ct{1182};
t6370 = ct{1183};
t6372 = ct{1184};
t6374 = ct{1185};
t6375 = ct{1186};
t6377 = ct{1187};
t6378 = ct{1188};
t6379 = ct{1189};
t6380 = ct{1190};
t6387 = ct{1191};
t6388 = ct{1192};
t6389 = ct{1193};
t6391 = ct{1194};
t6392 = ct{1195};
t6399 = ct{1196};
t6401 = ct{1197};
t6403 = ct{1198};
t6404 = ct{1199};
t6406 = ct{1200};
t6407 = ct{1201};
t6413 = ct{1202};
t6414 = ct{1203};
t6415 = ct{1204};
t642 = ct{1205};
t6422 = ct{1206};
t6423 = ct{1207};
t6424 = ct{1208};
t6425 = ct{1209};
t6427 = ct{1210};
t6428 = ct{1211};
t643 = ct{1212};
t6430 = ct{1213};
t6432 = ct{1214};
t6436 = ct{1215};
t6437 = ct{1216};
t6438 = ct{1217};
t6439 = ct{1218};
t6441 = ct{1219};
t6442 = ct{1220};
t6444 = ct{1221};
t6445 = ct{1222};
t6450 = ct{1223};
t6451 = ct{1224};
t6452 = ct{1225};
t6453 = ct{1226};
t6459 = ct{1227};
t6471 = ct{1228};
t6472 = ct{1229};
t6474 = ct{1230};
t6475 = ct{1231};
t6476 = ct{1232};
t6477 = ct{1233};
t6478 = ct{1234};
t6479 = ct{1235};
t6482 = ct{1236};
t6483 = ct{1237};
t6484 = ct{1238};
t6485 = ct{1239};
t6486 = ct{1240};
t6489 = ct{1241};
t649 = ct{1242};
t6490 = ct{1243};
t6491 = ct{1244};
t6492 = ct{1245};
t6493 = ct{1246};
t6495 = ct{1247};
t6496 = ct{1248};
t6497 = ct{1249};
t6500 = ct{1250};
t6502 = ct{1251};
t6505 = ct{1252};
t6507 = ct{1253};
t6508 = ct{1254};
t6510 = ct{1255};
t6511 = ct{1256};
t6512 = ct{1257};
t6515 = ct{1258};
t6521 = ct{1259};
t6522 = ct{1260};
t6523 = ct{1261};
t6528 = ct{1262};
t6529 = ct{1263};
t6534 = ct{1264};
t6536 = ct{1265};
t6538 = ct{1266};
t6540 = ct{1267};
t6541 = ct{1268};
t6542 = ct{1269};
t6543 = ct{1270};
t6544 = ct{1271};
t6546 = ct{1272};
t6547 = ct{1273};
t6548 = ct{1274};
t6550 = ct{1275};
t6551 = ct{1276};
t6552 = ct{1277};
t6553 = ct{1278};
t6554 = ct{1279};
t6555 = ct{1280};
t6556 = ct{1281};
t6557 = ct{1282};
t6558 = ct{1283};
t6559 = ct{1284};
t6560 = ct{1285};
t6561 = ct{1286};
t6562 = ct{1287};
t6563 = ct{1288};
t6564 = ct{1289};
t6565 = ct{1290};
t6566 = ct{1291};
t6577 = ct{1292};
t6584 = ct{1293};
t6585 = ct{1294};
t6587 = ct{1295};
t6588 = ct{1296};
t6595 = ct{1297};
t6596 = ct{1298};
t6597 = ct{1299};
t6598 = ct{1300};
t6599 = ct{1301};
t6600 = ct{1302};
t6601 = ct{1303};
t6603 = ct{1304};
t6604 = ct{1305};
t6605 = ct{1306};
t6606 = ct{1307};
t6608 = ct{1308};
t6609 = ct{1309};
t6610 = ct{1310};
t6611 = ct{1311};
t6612 = ct{1312};
t6613 = ct{1313};
t6614 = ct{1314};
t6615 = ct{1315};
t6616 = ct{1316};
t6617 = ct{1317};
t6620 = ct{1318};
t6622 = ct{1319};
t6623 = ct{1320};
t6624 = ct{1321};
t6625 = ct{1322};
t6627 = ct{1323};
t6628 = ct{1324};
t6629 = ct{1325};
t6631 = ct{1326};
t6638 = ct{1327};
t6641 = ct{1328};
t6645 = ct{1329};
t6647 = ct{1330};
t6648 = ct{1331};
t6649 = ct{1332};
t6653 = ct{1333};
t6655 = ct{1334};
t6656 = ct{1335};
t6657 = ct{1336};
t6658 = ct{1337};
t6659 = ct{1338};
t6660 = ct{1339};
t6663 = ct{1340};
t6664 = ct{1341};
t6667 = ct{1342};
t6668 = ct{1343};
t6669 = ct{1344};
t667 = ct{1345};
t6671 = ct{1346};
t6672 = ct{1347};
t6673 = ct{1348};
t6674 = ct{1349};
t6675 = ct{1350};
t6676 = ct{1351};
t6677 = ct{1352};
t6678 = ct{1353};
t6679 = ct{1354};
t6680 = ct{1355};
t6681 = ct{1356};
t6682 = ct{1357};
t6683 = ct{1358};
t6684 = ct{1359};
t6685 = ct{1360};
t6686 = ct{1361};
t6687 = ct{1362};
t6688 = ct{1363};
t6689 = ct{1364};
t6690 = ct{1365};
t6691 = ct{1366};
t6692 = ct{1367};
t6694 = ct{1368};
t6695 = ct{1369};
t6696 = ct{1370};
t6697 = ct{1371};
t6698 = ct{1372};
t6699 = ct{1373};
t670 = ct{1374};
t6700 = ct{1375};
t6701 = ct{1376};
t6703 = ct{1377};
t6707 = ct{1378};
t6710 = ct{1379};
t6711 = ct{1380};
t6713 = ct{1381};
t6714 = ct{1382};
t6716 = ct{1383};
t6717 = ct{1384};
t6720 = ct{1385};
t6722 = ct{1386};
t6725 = ct{1387};
t6727 = ct{1388};
t6728 = ct{1389};
t6729 = ct{1390};
t6730 = ct{1391};
t6731 = ct{1392};
t6733 = ct{1393};
t6734 = ct{1394};
t6735 = ct{1395};
t6736 = ct{1396};
t6737 = ct{1397};
t6738 = ct{1398};
t6739 = ct{1399};
t674 = ct{1400};
t6743 = ct{1401};
t6744 = ct{1402};
t6746 = ct{1403};
t6747 = ct{1404};
t6748 = ct{1405};
t6750 = ct{1406};
t6752 = ct{1407};
t6753 = ct{1408};
t6754 = ct{1409};
t6761 = ct{1410};
t6762 = ct{1411};
t6763 = ct{1412};
t6764 = ct{1413};
t6765 = ct{1414};
t6767 = ct{1415};
t6770 = ct{1416};
t6772 = ct{1417};
t6773 = ct{1418};
t6774 = ct{1419};
t6775 = ct{1420};
t6777 = ct{1421};
t6779 = ct{1422};
t6780 = ct{1423};
t6781 = ct{1424};
t6783 = ct{1425};
t6788 = ct{1426};
t6792 = ct{1427};
t6795 = ct{1428};
t6799 = ct{1429};
t6800 = ct{1430};
t6801 = ct{1431};
t6802 = ct{1432};
t6803 = ct{1433};
t6807 = ct{1434};
t6809 = ct{1435};
t6810 = ct{1436};
t6811 = ct{1437};
t6812 = ct{1438};
t6813 = ct{1439};
t6821 = ct{1440};
t6823 = ct{1441};
t6824 = ct{1442};
t6825 = ct{1443};
t6837 = ct{1444};
t6839 = ct{1445};
t684 = ct{1446};
t6841 = ct{1447};
t6842 = ct{1448};
t6843 = ct{1449};
t685 = ct{1450};
t6851 = ct{1451};
t6854 = ct{1452};
t6856 = ct{1453};
t6857 = ct{1454};
t6858 = ct{1455};
t686 = ct{1456};
t6860 = ct{1457};
t6861 = ct{1458};
t6863 = ct{1459};
t6864 = ct{1460};
t6865 = ct{1461};
t6866 = ct{1462};
t6868 = ct{1463};
t6869 = ct{1464};
t687 = ct{1465};
t6870 = ct{1466};
t6871 = ct{1467};
t6872 = ct{1468};
t6874 = ct{1469};
t6876 = ct{1470};
t6878 = ct{1471};
t6880 = ct{1472};
t6882 = ct{1473};
t6884 = ct{1474};
t6886 = ct{1475};
t6887 = ct{1476};
t6891 = ct{1477};
t6892 = ct{1478};
t6893 = ct{1479};
t6894 = ct{1480};
t6898 = ct{1481};
t6899 = ct{1482};
t6900 = ct{1483};
t6902 = ct{1484};
t6903 = ct{1485};
t6905 = ct{1486};
t6907 = ct{1487};
t6910 = ct{1488};
t6911 = ct{1489};
t6913 = ct{1490};
t6916 = ct{1491};
t6917 = ct{1492};
t6919 = ct{1493};
t6920 = ct{1494};
t6921 = ct{1495};
t6924 = ct{1496};
t6925 = ct{1497};
t6926 = ct{1498};
t6929 = ct{1499};
t6930 = ct{1500};
t6931 = ct{1501};
t6932 = ct{1502};
t6933 = ct{1503};
t6934 = ct{1504};
t6935 = ct{1505};
t6936 = ct{1506};
t6937 = ct{1507};
t6938 = ct{1508};
t6939 = ct{1509};
t6940 = ct{1510};
t6942 = ct{1511};
t6943 = ct{1512};
t6944 = ct{1513};
t6945 = ct{1514};
t6949 = ct{1515};
t6950 = ct{1516};
t6951 = ct{1517};
t6953 = ct{1518};
t6954 = ct{1519};
t6956 = ct{1520};
t6957 = ct{1521};
t6958 = ct{1522};
t6959 = ct{1523};
t6960 = ct{1524};
t6961 = ct{1525};
t6962 = ct{1526};
t6963 = ct{1527};
t6969 = ct{1528};
t6970 = ct{1529};
t6972 = ct{1530};
t6973 = ct{1531};
t6975 = ct{1532};
t6976 = ct{1533};
t6979 = ct{1534};
t6983 = ct{1535};
t6984 = ct{1536};
t6985 = ct{1537};
t6986 = ct{1538};
t6988 = ct{1539};
t6989 = ct{1540};
t6991 = ct{1541};
t6993 = ct{1542};
t6994 = ct{1543};
t7 = ct{1544};
t7000 = ct{1545};
t7001 = ct{1546};
t7003 = ct{1547};
t7004 = ct{1548};
t7006 = ct{1549};
t7010 = ct{1550};
t7017 = ct{1551};
t7019 = ct{1552};
t7022 = ct{1553};
t7023 = ct{1554};
t7024 = ct{1555};
t7030 = ct{1556};
t7033 = ct{1557};
t7039 = ct{1558};
t7040 = ct{1559};
t7041 = ct{1560};
t7047 = ct{1561};
t7050 = ct{1562};
t7052 = ct{1563};
t7053 = ct{1564};
t7054 = ct{1565};
t7055 = ct{1566};
t7056 = ct{1567};
t7057 = ct{1568};
t7058 = ct{1569};
t7060 = ct{1570};
t7063 = ct{1571};
t7066 = ct{1572};
t7068 = ct{1573};
t7069 = ct{1574};
t707 = ct{1575};
t7071 = ct{1576};
t7072 = ct{1577};
t7074 = ct{1578};
t7076 = ct{1579};
t7077 = ct{1580};
t7079 = ct{1581};
t708 = ct{1582};
t7086 = ct{1583};
t7087 = ct{1584};
t7089 = ct{1585};
t7090 = ct{1586};
t7091 = ct{1587};
t7093 = ct{1588};
t7094 = ct{1589};
t7095 = ct{1590};
t7099 = ct{1591};
t710 = ct{1592};
t7100 = ct{1593};
t7103 = ct{1594};
t7105 = ct{1595};
t7106 = ct{1596};
t7107 = ct{1597};
t7108 = ct{1598};
t7109 = ct{1599};
t7110 = ct{1600};
t7111 = ct{1601};
t7112 = ct{1602};
t7113 = ct{1603};
t7114 = ct{1604};
t7115 = ct{1605};
t7116 = ct{1606};
t7123 = ct{1607};
t7126 = ct{1608};
t7132 = ct{1609};
t7133 = ct{1610};
t7135 = ct{1611};
t7138 = ct{1612};
t7139 = ct{1613};
t7140 = ct{1614};
t7141 = ct{1615};
t7142 = ct{1616};
t7143 = ct{1617};
